simulink model "simulator_prototype_v2"  (R2021b)
(part 9 of 12)

t6280 = -t2307.*(t642+t643-t667+t674+t1587+t1606+t1608+t1609+t2295+t2671+t2683+t2684-t2695+t3272+t3290-t3296+t3576+t3582+t3588-t3593+t4015+t4016);
t6281 = -t2338.*(t642+t643-t667+t674+t1587+t1606+t1608+t1609+t2295+t2671+t2683+t2684-t2695+t3272+t3290-t3296+t3576+t3582+t3588-t3593+t4015+t4016);
t6282 = t5413.*t5588;
t6285 = t2338.*(t642+t643-t667+t674+t1587+t1606+t1608+t1609+t2295+t2671+t2683+t2684-t2695+t3272+t3290-t3296+t3576+t3582+t3588-t3593+t4015+t4016);
t6297 = -t5588.*(t410-t5413);
t6298 = t5588.*(t410-t5413);
t6304 = -t3386.*(t4554+t4572-t18.*t2363.*t3047.*1.02e-6-t23.*t2363.*t3047.*9.0e-8+t18.*t3946.*(t1896-t3232).*1.02e-6+t23.*t3946.*(t1896-t3232).*9.0e-8);
t6305 = t3386.*(t4554+t4572-t18.*t2363.*t3047.*1.02e-6-t23.*t2363.*t3047.*9.0e-8+t18.*t3946.*(t1896-t3232).*1.02e-6+t23.*t3946.*(t1896-t3232).*9.0e-8);
t6307 = t2363.*(t684+t685-t710+t724+t1686-t1690+t1700+t1701+t2371+t2698+t2707-t2716+t2719+t3319-t3327-t3341-t3620+t3622+t3634-t3638+t4076+t4077).*(-7.26735e-3);
t6308 = t2388.*(t684+t685-t710+t724+t1686-t1690+t1700+t1701+t2371+t2698+t2707-t2716+t2719+t3319-t3327-t3341-t3620+t3622+t3634-t3638+t4076+t4077).*(-7.26735e-3);
t6311 = t2419.*(t684+t685-t710+t724+t1686-t1690+t1700+t1701+t2371+t2698+t2707-t2716+t2719+t3319-t3327-t3341-t3620+t3622+t3634-t3638+t4076+t4077).*(-7.26735e-3);
t6314 = t3968+t4203+t4287+t4358+t4411+t4584;
t6315 = t4739+t4748+t4759+t4769;
t6327 = t33.*(t1896-t3232).*(t3424-t3437+t4552+t4556+t3942.*(t1896-t3232).*5.7e-7+t3946.*(t1896-t3232).*4.0e-8);
t6329 = -t33.*t3528.*(t3424-t3437+t4552+t4556+t3942.*(t1896-t3232).*5.7e-7+t3946.*(t1896-t3232).*4.0e-8);
t6331 = t33.*t3528.*(t3424-t3437+t4552+t4556+t3942.*(t1896-t3232).*5.7e-7+t3946.*(t1896-t3232).*4.0e-8);
t6338 = -t3877.*t5843.*(t1488+t1874+t2519+t2740+t2747+t3096+t3097);
t6348 = -t33.*t2363.*(t4737+t4744+t4751+t3942.*(t2694-t2701+t3036-t3043).*5.7e-7);
t6349 = t33.*t2363.*(t4737+t4744+t4751+t3942.*(t2694-t2701+t3036-t3043).*5.7e-7);
t6354 = -t2998.*(t4737+t4744+t4751+t3942.*(t2694-t2701+t3036-t3043).*5.7e-7);
t6355 = t2998.*(t4737+t4744+t4751+t3942.*(t2694-t2701+t3036-t3043).*5.7e-7);
t6357 = -t3057.*(t4737+t4744+t4751+t3942.*(t2694-t2701+t3036-t3043).*5.7e-7);
t6359 = (t1477-t2502).*(t4737+t4744+t4751+t3942.*(t2694-t2701+t3036-t3043).*5.7e-7);
t6360 = t3057.*(t4737+t4744+t4751+t3942.*(t2694-t2701+t3036-t3043).*5.7e-7);
t6369 = t4514.*t6038;
t6389 = t3385.*t6313;
t6394 = -t3985.*(t3424-t3437+t4552+t4556+t3942.*(t1896-t3232).*5.7e-7+t3946.*(t1896-t3232).*4.0e-8);
t6396 = (t3235-t3535).*(t3424-t3437+t4552+t4556+t3942.*(t1896-t3232).*5.7e-7+t3946.*(t1896-t3232).*4.0e-8);
t6397 = -t3992.*(t3424-t3437+t4552+t4556+t3942.*(t1896-t3232).*5.7e-7+t3946.*(t1896-t3232).*4.0e-8);
t6400 = -t3996.*(t3424-t3437+t4552+t4556+t3942.*(t1896-t3232).*5.7e-7+t3946.*(t1896-t3232).*4.0e-8);
t6408 = t33.*(t1896-t3232).*(t4737+t4744+t4751+t3942.*(t2694-t2701+t3036-t3043).*5.7e-7);
t6409 = -t33.*t3528.*(t4737+t4744+t4751+t3942.*(t2694-t2701+t3036-t3043).*5.7e-7);
t6411 = t33.*t3528.*(t4737+t4744+t4751+t3942.*(t2694-t2701+t3036-t3043).*5.7e-7);
t6427 = -t6426;
t6436 = t5588.*t5722;
t6437 = t5589.*t5722;
t6455 = -t3985.*(t4737+t4744+t4751+t3942.*(t2694-t2701+t3036-t3043).*5.7e-7);
t6456 = (t3235-t3535).*(t4737+t4744+t4751+t3942.*(t2694-t2701+t3036-t3043).*5.7e-7);
t6458 = -t3992.*(t4737+t4744+t4751+t3942.*(t2694-t2701+t3036-t3043).*5.7e-7);
t6463 = -t3996.*(t4737+t4744+t4751+t3942.*(t2694-t2701+t3036-t3043).*5.7e-7);
t6464 = t3992.*(t4737+t4744+t4751+t3942.*(t2694-t2701+t3036-t3043).*5.7e-7);
t6473 = t3049+t3256+t3266+t3976+t3980+t4373+t4378+t4387+t4394;
t6480 = -t4510.*(t4554+t4572-t18.*t2363.*t3047.*1.02e-6-t23.*t2363.*t3047.*9.0e-8+t18.*t3946.*(t1896-t3232).*1.02e-6+t23.*t3946.*(t1896-t3232).*9.0e-8);
t6483 = (t3544-t4013).*(t4554+t4572-t18.*t2363.*t3047.*1.02e-6-t23.*t2363.*t3047.*9.0e-8+t18.*t3946.*(t1896-t3232).*1.02e-6+t23.*t3946.*(t1896-t3232).*9.0e-8);
t6489 = t5426.*t5839;
t6490 = t5429.*t5839;
t6492 = -t5840.*(t410-t5413);
t6518 = -t4817.*(t3424-t3437+t4552+t4556+t3942.*(t1896-t3232).*5.7e-7+t3946.*(t1896-t3232).*4.0e-8);
t6519 = -t4824.*(t3424-t3437+t4552+t4556+t3942.*(t1896-t3232).*5.7e-7+t3946.*(t1896-t3232).*4.0e-8);
t6523 = t4514.*t6313;
t6534 = -t6533;
t6539 = t3180+t3196+t4735+t4743+t5017+t5022;
t6545 = -t3057.*(t4819+t4850+t4851+t3057.*(t1456-t2355).*1.02e-6+t3047.*(t1477-t2502).*1.02e-6+t3942.*(t3235-t3535).*1.02e-6);
et198 = -t2137+t2777+t2778+t2779-t2787+t4012-t4205+t4207+t27.*(t1959-t3306+t38.*t1022.*(t855-t878).*2.196325630278387e-1).*6.1855407534e-5;
et199 = t33.*(t1959-t3306+t38.*t1022.*(t855-t878).*2.196325630278387e-1).*1.35652563578e-4;
t6567 = -t5426.*(et198+et199);
et200 = -t2137+t2777+t2778+t2779-t2787+t4012-t4205+t4207+t27.*(t1959-t3306+t38.*t1022.*(t855-t878).*2.196325630278387e-1).*6.1855407534e-5;
et201 = t33.*(t1959-t3306+t38.*t1022.*(t855-t878).*2.196325630278387e-1).*1.35652563578e-4;
t6568 = t5426.*(et200+et201);
et202 = -t2137+t2777+t2778+t2779-t2787+t4012-t4205+t4207+t27.*(t1959-t3306+t38.*t1022.*(t855-t878).*2.196325630278387e-1).*6.1855407534e-5;
et203 = t33.*(t1959-t3306+t38.*t1022.*(t855-t878).*2.196325630278387e-1).*1.35652563578e-4;
t6569 = -t5429.*(et202+et203);
et204 = -t2137+t2777+t2778+t2779-t2787+t4012-t4205+t4207+t27.*(t1959-t3306+t38.*t1022.*(t855-t878).*2.196325630278387e-1).*6.1855407534e-5;
et205 = t33.*(t1959-t3306+t38.*t1022.*(t855-t878).*2.196325630278387e-1).*1.35652563578e-4;
t6570 = t5429.*(et204+et205);
t6572 = -t5992.*(t410-t5413);
t6573 = -t4817.*(t4737+t4744+t4751+t3942.*(t2694-t2701+t3036-t3043).*5.7e-7);
t6574 = -t4824.*(t4737+t4744+t4751+t3942.*(t2694-t2701+t3036-t3043).*5.7e-7);
t6585 = t5548.*t5951;
t6586 = t5588.*t5941;
t6591 = t5589.*t5941;
t6600 = t5588.*t5953;
et206 = t707+t708-t721-t722-t749+t762+t768-t777-t792-t793-t801-t802-t808+t813-t819+t821-t1629+t1637-t1640-t1641-t1659-t1661+t1666+t1667+t1683+t1692+t1705-t1712+t1758+t1759+t1775+t1776+t1973+t1993+t1994+t2023+t2053+t2060-t2089-t2090+t2098+t2099-t14.*t15.*t21.*t50.*t189.*3.670836568391568e-22;
et207 = t16.*t19.*t20.*t50.*t189.*(-3.279367663374749e-19)-t14.*t15.*t17.*t21.*t50.*t189.*7.075931802640439e-19;
et208 = t14.*t17.*t20.*t21.*t50.*t189.*(-1.190170786299927e-18)-t15.*t17.*t19.*t21.*t50.*t189.*1.190170786299927e-18;
et209 = t19.*t20.*t21.*t22.*t50.*t189.*(-3.226512155691387e-19);
t6602 = -t5588.*(et206+et207+et208+et209);
et210 = t707+t708-t721-t722-t749+t762+t768-t777-t792-t793-t801-t802-t808+t813-t819+t821-t1629+t1637-t1640-t1641-t1659-t1661+t1666+t1667+t1683+t1692+t1705-t1712+t1758+t1759+t1775+t1776+t1973+t1993+t1994+t2023+t2053+t2060-t2089-t2090+t2098+t2099-t14.*t15.*t21.*t50.*t189.*3.670836568391568e-22;
et211 = t16.*t19.*t20.*t50.*t189.*(-3.279367663374749e-19)-t14.*t15.*t17.*t21.*t50.*t189.*7.075931802640439e-19;
et212 = t14.*t17.*t20.*t21.*t50.*t189.*(-1.190170786299927e-18)-t15.*t17.*t19.*t21.*t50.*t189.*1.190170786299927e-18;
et213 = t19.*t20.*t21.*t22.*t50.*t189.*(-3.226512155691387e-19);
t6603 = t5588.*(et210+et211+et212+et213);
t6604 = t5589.*t5953;
t6635 = -t6633;
t6660 = (t3235-t3535).*(t4819+t4850+t4851+t3057.*(t1456-t2355).*1.02e-6+t3047.*(t1477-t2502).*1.02e-6+t3942.*(t3235-t3535).*1.02e-6);
t6662 = -t3992.*(t4819+t4850+t4851+t3057.*(t1456-t2355).*1.02e-6+t3047.*(t1477-t2502).*1.02e-6+t3942.*(t3235-t3535).*1.02e-6);
t6664 = t3992.*(t4819+t4850+t4851+t3057.*(t1456-t2355).*1.02e-6+t3047.*(t1477-t2502).*1.02e-6+t3942.*(t3235-t3535).*1.02e-6);
t6703 = t3057.*t6646;
t6706 = t5176+t5177+t5179+t5180;
t6753 = t5413.*t6183;
et214 = t1288+t1289+t1302+t1303-t1319-t1320+t1336-t1348+t1350+t1351-t1360+t1369-t1378+t1396-t1425+t1435-t2174+t2183-t2187+t2193-t2194-t2195+t2199-t2203-t2215+t2219-t2222-t2223+t2239+t2240-t2256-t2257+t2555+t2556+t2572+t2583-t2605-t2606+t2612+t2613-t2618-t2619+t2651+t2652;
et215 = t24.*t25.*t26.*t50.*t202.*(-3.566935413776081e-21);
et216 = t30.*t31.*t32.*t50.*t202.*(-3.992732227073824e-24);
et217 = t24.*t25.*t32.*t33.*t50.*t202.*(-3.509445006623964e-21);
et218 = t27.*t30.*t31.*t32.*t50.*t202.*(-7.696420262413979e-21);
t6763 = -t5426.*(et214+et215+et216+et217+et218);
et219 = t1288+t1289+t1302+t1303-t1319-t1320+t1336-t1348+t1350+t1351-t1360+t1369-t1378+t1396-t1425+t1435-t2174+t2183-t2187+t2193-t2194-t2195+t2199-t2203-t2215+t2219-t2222-t2223+t2239+t2240-t2256-t2257+t2555+t2556+t2572+t2583-t2605-t2606+t2612+t2613-t2618-t2619+t2651+t2652;
et220 = t24.*t25.*t26.*t50.*t202.*(-3.566935413776081e-21);
et221 = t30.*t31.*t32.*t50.*t202.*(-3.992732227073824e-24);
et222 = t24.*t25.*t32.*t33.*t50.*t202.*(-3.509445006623964e-21);
et223 = t27.*t30.*t31.*t32.*t50.*t202.*(-7.696420262413979e-21);
t6764 = t5426.*(et219+et220+et221+et222+et223);
t6776 = -t27.*t2363.*(-t4437-t4438+t4741+t4767+t3942.*(t2694-t2701+t3036-t3043).*4.0e-8+t3946.*(t2694-t2701+t3036-t3043).*2.4e-7);
t6777 = t27.*t2363.*(-t4437-t4438+t4741+t4767+t3942.*(t2694-t2701+t3036-t3043).*4.0e-8+t3946.*(t2694-t2701+t3036-t3043).*2.4e-7);
t6789 = -t3003.*(-t4437-t4438+t4741+t4767+t3942.*(t2694-t2701+t3036-t3043).*4.0e-8+t3946.*(t2694-t2701+t3036-t3043).*2.4e-7);
t6790 = t3003.*(-t4437-t4438+t4741+t4767+t3942.*(t2694-t2701+t3036-t3043).*4.0e-8+t3946.*(t2694-t2701+t3036-t3043).*2.4e-7);
t6793 = -t3057.*(-t4437-t4438+t4741+t4767+t3942.*(t2694-t2701+t3036-t3043).*4.0e-8+t3946.*(t2694-t2701+t3036-t3043).*2.4e-7);
t6794 = (t1477-t2502).*(-t4437-t4438+t4741+t4767+t3942.*(t2694-t2701+t3036-t3043).*4.0e-8+t3946.*(t2694-t2701+t3036-t3043).*2.4e-7);
t6796 = -t6646.*(t3235-t3535);
t6797 = t3992.*t6646;
t6804 = t4307+t4314+t4876+t4877+t4978+t4979;
t6805 = t5053+t5676+t5690;
t6807 = t3876+t4274+t4968+t4969+t5003+t5004;
t6814 = t27.*(t1896-t3232).*(-t4437-t4438+t4741+t4767+t3942.*(t2694-t2701+t3036-t3043).*4.0e-8+t3946.*(t2694-t2701+t3036-t3043).*2.4e-7);
t6815 = -t27.*t3528.*(-t4437-t4438+t4741+t4767+t3942.*(t2694-t2701+t3036-t3043).*4.0e-8+t3946.*(t2694-t2701+t3036-t3043).*2.4e-7);
t6835 = t3133+t3160+t3161+t3379+t4236+t4240+t4249+t4250+t4255+t4256+t4499+t4505;
t6885 = -t3985.*(-t4437-t4438+t4741+t4767+t3942.*(t2694-t2701+t3036-t3043).*4.0e-8+t3946.*(t2694-t2701+t3036-t3043).*2.4e-7);
t6887 = (t3235-t3535).*(-t4437-t4438+t4741+t4767+t3942.*(t2694-t2701+t3036-t3043).*4.0e-8+t3946.*(t2694-t2701+t3036-t3043).*2.4e-7);
t6888 = -t3992.*(-t4437-t4438+t4741+t4767+t3942.*(t2694-t2701+t3036-t3043).*4.0e-8+t3946.*(t2694-t2701+t3036-t3043).*2.4e-7);
t6890 = -t3996.*(-t4437-t4438+t4741+t4767+t3942.*(t2694-t2701+t3036-t3043).*4.0e-8+t3946.*(t2694-t2701+t3036-t3043).*2.4e-7);
t6908 = t5229+t5237+t5274+t5279;
t6909 = t3918.*(t4758.*(t1861-t3214)+t2297.*(t642+t643-t667+t674+t1587+t1606+t1608+t1609+t2295+t2671+t2683+t2684-t2695+t3272+t3290-t3296+t3576+t3582+t3588-t3593+t4015+t4016)).*(t2694-t2701+t3036-t3043).*7.26735e-3;
t6920 = t3984.*(t4758.*(t1861-t3214)+t2297.*(t642+t643-t667+t674+t1587+t1606+t1608+t1609+t2295+t2671+t2683+t2684-t2695+t3272+t3290-t3296+t3576+t3582+t3588-t3593+t4015+t4016)).*(t2694-t2701+t3036-t3043).*7.26735e-3;
t6923 = -t3877.*t6566.*(t1488+t1874+t2519+t2740+t2747+t3096+t3097);
t6925 = t3877.*t6566.*(t1488+t1874+t2519+t2740+t2747+t3096+t3097);
t6926 = t4149.*(t4758.*(t1861-t3214)+t2297.*(t642+t643-t667+t674+t1587+t1606+t1608+t1609+t2295+t2671+t2683+t2684-t2695+t3272+t3290-t3296+t3576+t3582+t3588-t3593+t4015+t4016)).*(t2694-t2701+t3036-t3043).*7.26735e-3;
t6958 = t3941.*(t4795.*(t1896-t3232).*7.26735e-3+t2363.*(t684+t685-t710+t724+t1686-t1690+t1700+t1701+t2371+t2698+t2707-t2716+t2719+t3319-t3327-t3341-t3620+t3622+t3634-t3638+t4076+t4077).*7.26735e-3).*(t2674-t2676+t3022-t3027);
t6972 = t4108.*(t4795.*(t1896-t3232).*7.26735e-3+t2363.*(t684+t685-t710+t724+t1686-t1690+t1700+t1701+t2371+t2698+t2707-t2716+t2719+t3319-t3327-t3341-t3620+t3622+t3634-t3638+t4076+t4077).*7.26735e-3).*(t2674-t2676+t3022-t3027);
t6974 = t5209+t5753+t5766;
t6984 = t4298.*(t4795.*(t1896-t3232).*7.26735e-3+t2363.*(t684+t685-t710+t724+t1686-t1690+t1700+t1701+t2371+t2698+t2707-t2716+t2719+t3319-t3327-t3341-t3620+t3622+t3634-t3638+t4076+t4077).*7.26735e-3).*(t2674-t2676+t3022-t3027);
t6986 = t3158+t3171+t3438+t3442+t4253+t4260+t4262+t4267+t4516+t4537+t4562+t4566;
t6992 = -t4814.*(-t4437-t4438+t4741+t4767+t3942.*(t2694-t2701+t3036-t3043).*4.0e-8+t3946.*(t2694-t2701+t3036-t3043).*2.4e-7);
et224 = t4127+t33.*(t1959-t3306+t38.*t1022.*(t855-t878).*2.196325630278387e-1);
et225 = -t4437-t4438+t4741+t4767+t3942.*(t2694-t2701+t3036-t3043).*4.0e-8+t3946.*(t2694-t2701+t3036-t3043).*2.4e-7;
t6993 = et224.*et225;
t7046 = t3558+t3559+t5260+t5261+t5268+t5269;
et226 = t3563.*1.33637554986e-4+t3693-t3694+t33.*(t1896-t3232).*4.36041e-5;
et227 = t33.*t34.*(t1896-t3232).*7.26350557185e-5;
t7050 = (et226+et227).*(t4758.*(t1861-t3214)+t2297.*(t642+t643-t667+t674+t1587+t1606+t1608+t1609+t2295+t2671+t2683+t2684-t2695+t3272+t3290-t3296+t3576+t3582+t3588-t3593+t4015+t4016));
et228 = t4758.*(t1861-t3214)+t2297.*(t642+t643-t667+t674+t1587+t1606+t1608+t1609+t2295+t2671+t2683+t2684-t2695+t3272+t3290-t3296+t3576+t3582+t3588-t3593+t4015+t4016);
et229 = t3349-t3649+t28.*(t3235-t3535).*1.33637554986e-4+t34.*(t3235-t3535).*7.26350557185e-5;
t7053 = et228.*et229;
t7056 = -t6975.*(-t1901+t3122+t3270);
et230 = t4795.*(t1896-t3232).*7.26735e-3+t2363.*(t684+t685-t710+t724+t1686-t1690+t1700+t1701+t2371+t2698+t2707-t2716+t2719+t3319-t3327-t3341-t3620+t3622+t3634-t3638+t4076+t4077).*7.26735e-3;
et231 = t3505.*1.838876e-2-t3570+t3571+t22.*(t1861-t3214).*(3.0./5.0e+2)+t22.*t23.*(t1861-t3214).*9.99471e-3;
t7057 = et230.*et231;
t7058 = t50.*t202.*t7042.*6.935255936130809e-19;
tau_c = ft_13({t1005,t1022,t1089,t1104,t1105,t1108,t1115,t1121,t1158,t1159,t1196,t1205,t1210,t1212,t1217,t1218,t123,t1237,t1238,t1288,t1289,t1302,t1303,t1319,t1320,t1336,t1348,t1350,t1351,t1360,t1369,t1378,t1396,t14,t140,t1425,t1435,t1456,t1477,t1488,t15,t1513,t1539,t1554,t1577,t1578,t1586,t1587,t16,t1600,t1604,t1605,t1606,t1607,t1608,t1609,t1615,t1616,t1628,t1629,t1637,t1640,t1641,t1659,t1660,t1661,t1666,t1667,t1683,t1686,t1690,t1692,t17,t1700,t1701,t1705,t1712,t1717,t1741,t1742,t1750,t1754,t1758,t1759,t1775,t1776,t18,t1861,t1874,t1879,t188,t1881,t189,t1896,t19,t1901,t1941,t1959,t1973,t1993,t1994,t2,t20,t201,t202,t2023,t2053,t2060,t2089,t2090,t2098,t2099,t21,t2117,t2120,t2122,t2123,t2139,t2140,t2147,t2152,t2154,t2155,t2159,t2165,t2174,t2183,t2187,t2193,t2194,t2195,t2199,t22,t2203,t2215,t2219,t2222,t2223,t2239,t2240,t2256,t2257,t2292,t2295,t2297,t23,t2302,t2303,t2306,t2307,t2308,t2317,t2337,t2338,t2339,t2355,t236,t2361,t2362,t2363,t2367,t2368,t237,t2371,t2378,t238,t2388,t24,t2401,t2403,t241,t2414,t2419,t244,t2493,t25,t2502,t2510,t2519,t2527,t2530,t2555,t2556,t2572,t2583,t2598,t26,t2605,t2606,t2612,t2613,t2618,t2619,t262,t264,t2651,t2652,t2670,t2671,t2673,t2674,t2676,t2680,t2683,t2684,t2685,t2686,t2687,t2689,t2692,t2693,t2694,t2695,t2697,t2698,t27,t2700,t2701,t2704,t2707,t2708,t2709,t2712,t2715,t2716,t2719,t2720,t2721,t2740,t2747,t2754,t28,t2801,t2804,t2813,t2814,t2820,t2831,t2834,t2835,t2838,t2850,t2851,t2945,t2950,t2953,t2955,t2957,t2963,t2964,t2975,t2979,t2990,t2991,t2993,t2994,t2998,t3,t30,t3003,t3009,t3017,t3022,t3027,t3030,t3036,t3043,t3045,t3047,t3054,t3055,t3056,t3057,t3063,t3064,t3072,t3079,t3080,t3096,t3097,t31,t3109,t3117,t3118,t3121,t3122,t3128,t3129,t313,t3130,t3131,t3132,t3134,t3135,t3139,t314,t3140,t3141,t3142,t3144,t3147,t3155,t3156,t3157,t3164,t3166,t3170,t3172,t3184,t3186,t3187,t3188,t3189,t3190,t3191,t3193,t3194,t3197,t3198,t3199,t32,t3200,t3201,t3206,t3209,t321,t3210,t3214,t3225,t3228,t3229,t3230,t3231,t3232,t3235,t3245,t3250,t3254,t3260,t3261,t3263,t3269,t3270,t3272,t3276,t3283,t329,t3290,t3291,t3292,t3296,t33,t3305,t3306,t3307,t3308,t3313,t3316,t3318,t3319,t332,t3324,t3326,t3327,t3330,t3334,t3335,t3336,t3337,t3341,t3344,t3349,t335,t3353,t3354,t3357,t3359,t3360,t3376,t3385,t3386,t3395,t3399,t34,t3405,t3409,t3410,t3412,t3415,t3417,t3419,t3420,t3421,t3423,t3424,t3428,t3432,t3433,t3435,t3437,t3440,t3444,t3449,t3450,t3451,t3453,t3455,t3456,t346,t3465,t3468,t3470,t3473,t3475,t3477,t3479,t3480,t3481,t3483,t3484,t3493,t3498,t35,t350,t3505,t3518,t3522,t3524,t3526,t3527,t3528,t3530,t3531,t3532,t3533,t3535,t3539,t354,t3542,t3544,t3547,t3560,t3563,t3569,t3570,t3571,t3576,t358,t3582,t3585,t3586,t3587,t3588,t3589,t359,t3590,t3593,t3596,t36,t3600,t3603,t3616,t3617,t3618,t3619,t3620,t3621,t3622,t3628,t3631,t3632,t3633,t3634,t3635,t3637,t3638,t3639,t3641,t3643,t3649,t3657,t366,t3663,t3664,t3665,t3667,t3669,t3670,t3672,t3673,t3674,t3676,t3678,t3679,t3680,t3681,t3682,t3683,t3684,t3685,t3686,t3687,t3689,t3690,t3693,t3694,t3705,t3706,t3708,t3709,t3712,t3713,t3714,t3715,t3716,t3718,t3723,t3724,t3729,t3732,t3734,t3735,t3736,t3744,t3745,t3746,t3748,t3749,t3751,t3753,t3755,t3756,t3757,t3758,t3759,t3760,t3762,t3763,t3764,t3765,t3766,t3767,t3768,t3769,t3770,t3771,t3772,t3774,t3775,t3776,t3778,t3779,t378,t3782,t3783,t3784,t3790,t3791,t3794,t3795,t3797,t3798,t3799,t38,t3801,t3803,t3804,t3806,t3811,t3814,t3815,t3816,t3817,t3819,t382,t3821,t3822,t3826,t3827,t3828,t3833,t3834,t3844,t3847,t3849,t3850,t3860,t3861,t3862,t3863,t3865,t3866,t3869,t387,t3870,t3871,t3872,t3875,t3877,t3880,t3882,t3891,t3892,t3893,t3898,t39,t3901,t3904,t3910,t3918,t3922,t3928,t3934,t3940,t3941,t3942,t3943,t3946,t3951,t3957,t3959,t3967,t3972,t3974,t3984,t3985,t3992,t3996,t4,t4007,t4011,t4013,t4015,t4016,t4027,t4034,t4035,t4036,t4037,t4062,t4071,t4072,t4076,t4077,t4080,t4086,t4089,t4090,t4091,t410,t4106,t4108,t4109,t4113,t4119,t4120,t4122,t4125,t4127,t4133,t4134,t4145,t4146,t4147,t4148,t4149,t4152,t4154,t4155,t4160,t4163,t4168,t4173,t4175,t4196,t42,t4200,t4201,t4219,t4220,t4221,t4227,t4228,t4230,t4231,t4233,t4234,t4235,t4237,t4238,t4239,t4242,t4243,t4244,t4245,t4246,t4247,t4248,t4255,t4256,t4257,t4259,t4263,t4264,t4266,t4268,t4276,t4277,t4279,t4280,t4281,t4285,t4287,t4291,t4292,t4295,t4296,t4297,t4298,t43,t4304,t4308,t4310,t4311,t4313,t4316,t4320,t4321,t4322,t4323,t4324,t4356,t4362,t4363,t4374,t4376,t4377,t4379,t4382,t4388,t4397,t4398,t4400,t4405,t4406,t4409,t4410,t4412,t4413,t4421,t4424,t4427,t4428,t4429,t4432,t4436,t4437,t4438,t4439,t4440,t4444,t4447,t4458,t4473,t4475,t4491,t4494,t4496,t4499,t4500,t4504,t4507,t4508,t4510,t4511,t4513,t4514,t4515,t4517,t4519,t4520,t4523,t4525,t4529,t4531,t4534,t4535,t4536,t4540,t4541,t4543,t4552,t4554,t4555,t4556,t4559,t4560,t4561,t4565,t4568,t4571,t4572,t4575,t4576,t4579,t4580,t4581,t4582,t4588,t4589,t4591,t4593,t4594,t4595,t4597,t4599,t46,t4600,t4602,t4610,t4612,t4613,t4614,t4615,t4617,t4620,t4623,t4625,t4627,t4628,t4629,t4631,t4633,t4634,t4635,t4636,t4638,t4640,t4641,t4642,t4644,t4645,t4647,t4650,t4651,t4652,t4655,t4658,t4659,t4661,t4663,t4664,t4666,t4667,t4669,t4676,t4677,t4678,t4679,t4680,t4682,t4683,t4685,t4686,t4688,t4699,t47,t4702,t4703,t4704,t4705,t4706,t4709,t4713,t4715,t4718,t4719,t4720,t4721,t4725,t4727,t4728,t4729,t4732,t4733,t4737,t4738,t4741,t4742,t4744,t4751,t4752,t4753,t4755,t4757,t4758,t4760,t4761,t4762,t4763,t4766,t4767,t4770,t4771,t4772,t4773,t4775,t4777,t4780,t4785,t4786,t4787,t4788,t4789,t4790,t4791,t4792,t4793,t4794,t4795,t4796,t4798,t4799,t4800,t4801,t4805,t4807,t4808,t4809,t4812,t4814,t4816,t4817,t4818,t4819,t4822,t4823,t4824,t4825,t4826,t4829,t4832,t4833,t4835,t4836,t4839,t4840,t4842,t4843,t4845,t4847,t4848,t4849,t4850,t4851,t4852,t4853,t4854,t4855,t4856,t4857,t4858,t4859,t4860,t4865,t4868,t4869,t4870,t4871,t4872,t4873,t4874,t4875,t4880,t4882,t4883,t4884,t4885,t4887,t4890,t4893,t4895,t4896,t4897,t4898,t4899,t4900,t4902,t4904,t4905,t4906,t4907,t4909,t4911,t4913,t4915,t4917,t4918,t4919,t4920,t4921,t4922,t4924,t4925,t4926,t4927,t4929,t4930,t4931,t4932,t4938,t4941,t4942,t4943,t4946,t4947,t4950,t4952,t4953,t4954,t4956,t4958,t4959,t4960,t4961,t4962,t4963,t4965,t4970,t4972,t4974,t4975,t4976,t4977,t4981,t4982,t4983,t4984,t4985,t4986,t4987,t4992,t4994,t4995,t4996,t4998,t5,t50,t5000,t5001,t5002,t5005,t5007,t5008,t5010,t5012,t5013,t5014,t5015,t5021,t5023,t5025,t5026,t5027,t5028,t5030,t5031,t5032,t5033,t5034,t5035,t5036,t5038,t5039,t5040,t5041,t5042,t5047,t5048,t5049,t5051,t5052,t5054,t5055,t5056,t5057,t5058,t5059,t5061,t5062,t5063,t5064,t5066,t5067,t5068,t5069,t5070,t5071,t5073,t5074,t5075,t5076,t5077,t5083,t5085,t5086,t5087,t5088,t5089,t5092,t5097,t5098,t5099,t5100,t5102,t5103,t5104,t5105,t5106,t5108,t5109,t5111,t5112,t5113,t5114,t5115,t5116,t5117,t5119,t5121,t5123,t5126,t5127,t5128,t5130,t5131,t5135,t5137,t5138,t5139,t5141,t5142,t5143,t5144,t5145,t5146,t5147,t5148,t5149,t5150,t5151,t5152,t5153,t5155,t5156,t5157,t5158,t5161,t5162,t5164,t5165,t5166,t5169,t5172,t5173,t5184,t5185,t5186,t5187,t5189,t5190,t5191,t5192,t5193,t5194,t5195,t5196,t5198,t5201,t5202,t5203,t5204,t5206,t5207,t5208,t5209,t5210,t5212,t5214,t5215,t5216,t5217,t5220,t5221,t5222,t5223,t5224,t5225,t5226,t5227,t5228,t5230,t5231,t5233,t5234,t5235,t5236,t5238,t5239,t5240,t5241,t5242,t5243,t5244,t5245,t5246,t5247,t5248,t5250,t5252,t5254,t5255,t5257,t5258,t5262,t5271,t5272,t5273,t5276,t5277,t5278,t5280,t5281,t5282,t5283,t5284,t5285,t5286,t5287,t5288,t5289,t5291,t5293,t5295,t5301,t5302,t5304,t5306,t5307,t5308,t5309,t5311,t5314,t5316,t5317,t5320,t5321,t5322,t5326,t5328,t5329,t5330,t5331,t5332,t5333,t5335,t5336,t5337,t5338,t5339,t5340,t5342,t5344,t5345,t5346,t5347,t5348,t5349,t5350,t5352,t5356,t5357,t5358,t5359,t5361,t5362,t5365,t5367,t5371,t5377,t5379,t5380,t5381,t5383,t5384,t5385,t5386,t5387,t5388,t5389,t5390,t5391,t5392,t5393,t5395,t5396,t5397,t5399,t5400,t5402,t5403,t5405,t5407,t5408,t5409,t5411,t5412,t5413,t5414,t5416,t5418,t5419,t5420,t5423,t5424,t5426,t5427,t5428,t5429,t5430,t5432,t5433,t5434,t5435,t5437,t5438,t5440,t5441,t5443,t5444,t5445,t5446,t5447,t5448,t5449,t5450,t5451,t5452,t5453,t5454,t5455,t5456,t5457,t5458,t5459,t5461,t5462,t5464,t5465,t5466,t5467,t5468,t5469,t5473,t5474,t5476,t5477,t5479,t5480,t5481,t5482,t5483,t5484,t5485,t5486,t5487,t5488,t5489,t5490,t5491,t5492,t5493,t5494,t5496,t5498,t5499,t5500,t5503,t5504,t5505,t5506,t5507,t5509,t5512,t5513,t5514,t5515,t5516,t5517,t5518,t5520,t5521,t5522,t5523,t5524,t5525,t5526,t5528,t5530,t5531,t5532,t5533,t5534,t5535,t5536,t5537,t5538,t5539,t5541,t5542,t5543,t5544,t5545,t5546,t5547,t5550,t5551,t5552,t5553,t5554,t5556,t5557,t5558,t5559,t5561,t5563,t5564,t5566,t5568,t5569,t5570,t5573,t5574,t5575,t5576,t5577,t5578,t5579,t5580,t5581,t5582,t5583,t5585,t5588,t5589,t5590,t5592,t5593,t5594,t5595,t5596,t5597,t56,t5600,t5601,t5602,t5603,t5604,t5605,t5606,t5610,t5615,t5617,t5619,t5620,t5621,t5622,t5623,t5624,t5625,t5626,t5627,t5628,t5629,t5631,t5632,t5635,t5636,t5639,t5641,t5644,t5648,t5651,t5653,t5655,t5658,t5659,t5660,t5661,t5662,t5663,t5664,t5665,t5666,t5667,t5670,t5671,t5674,t5675,t5678,t5679,t5680,t5681,t5682,t5685,t5686,t5687,t5689,t5691,t5693,t5694,t5695,t5696,t5698,t5699,t5700,t5701,t5702,t5703,t5704,t5705,t5706,t5707,t5708,t5709,t5711,t5712,t5714,t5715,t5717,t5718,t5720,t5721,t5722,t5723,t5725,t5726,t5727,t5728,t5730,t5731,t5733,t5735,t5737,t5739,t5740,t5741,t5742,t5748,t5749,t5750,t5751,t5756,t5757,t5760,t5761,t5762,t5764,t5765,t5768,t5770,t5771,t5772,t5773,t5775,t5776,t5777,t5778,t5779,t5780,t5782,t5783,t5785,t5786,t5787,t5788,t5791,t5792,t5793,t5794,t5796,t5798,t5799,t5804,t5805,t5807,t5808,t5809,t5813,t5815,t5816,t5818,t5820,t5821,t5824,t5825,t5828,t5829,t5831,t5832,t5833,t5835,t5836,t5838,t5840,t5842,t5843,t5845,t5846,t5850,t5851,t5852,t5853,t5854,t5855,t5857,t5858,t5859,t5860,t5861,t5862,t5863,t5864,t5865,t5866,t5868,t5870,t5871,t5873,t5876,t5877,t5879,t5881,t5882,t5883,t5884,t5887,t5888,t5889,t5890,t5891,t5894,t5896,t5899,t5900,t5902,t5904,t5907,t5908,t5910,t5911,t5912,t5913,t5914,t5916,t5917,t5918,t5922,t5923,t5924,t5926,t5927,t5929,t5930,t5932,t5933,t5935,t5937,t5940,t5943,t5944,t5945,t5947,t5951,t5952,t5953,t5954,t5956,t5957,t5958,t5959,t5960,t5963,t5966,t5968,t5969,t5970,t5972,t5975,t5977,t5978,t5979,t5980,t5981,t5986,t5988,t5991,t5992,t5994,t5996,t5997,t5998,t6,t60,t6000,t6001,t6002,t6004,t6008,t6009,t6010,t6012,t6015,t6016,t6017,t6018,t6019,t6020,t6021,t6028,t6030,t6031,t6034,t6035,t6038,t6039,t6042,t6043,t6046,t6047,t6049,t6050,t6051,t6054,t6057,t6058,t6060,t6062,t6064,t6066,t6067,t6075,t6076,t6087,t6088,t6091,t6092,t6095,t6096,t6100,t6101,t6103,t6104,t6112,t6119,t6135,t6137,t6138,t6140,t6143,t6144,t6147,t6150,t6151,t6156,t6160,t6161,t6162,t6165,t6168,t6169,t6173,t6175,t6183,t6184,t6185,t6189,t6198,t6199,t6200,t6201,t6202,t6206,t6207,t6209,t6210,t6211,t6219,t6221,t6223,t6224,t6232,t6238,t6244,t6245,t6247,t6248,t6251,t6253,t6257,t6267,t6271,t6279,t6280,t6282,t6285,t6293,t6297,t6298,t6302,t6303,t6304,t6305,t6307,t6308,t6311,t6313,t6315,t6317,t6321,t6322,t6323,t6327,t6331,t6338,t6339,t6341,t6343,t6344,t6348,t6349,t6354,t6356,t6357,t6359,t6360,t6365,t6366,t6367,t6369,t6375,t6378,t6387,t6388,t6389,t6394,t6396,t6397,t640,t6400,t6406,t6407,t6408,t6411,t6414,t642,t6427,t643,t6431,t6436,t6437,t6441,t6442,t6450,t6451,t6452,t6453,t6455,t6456,t6463,t6464,t6473,t6480,t6481,t6483,t6484,t6485,t6486,t6489,t649,t6490,t6492,t6493,t6497,t6507,t6508,t6511,t6515,t6518,t6519,t6521,t6523,t6528,t6529,t6533,t6534,t6539,t6543,t6544,t6545,t656,t6565,t6566,t6568,t6570,t6572,t6573,t6574,t6575,t6584,t6585,t6586,t659,t6591,t6593,t660,t6600,t6603,t6604,t6611,t6612,t6634,t6635,t6658,t6660,t6663,t6664,t667,t668,t6689,t669,t6691,t6692,t67,t670,t6703,t6706,t674,t6752,t6753,t6763,t6764,t677,t6776,t6777,t6789,t6793,t6794,t6796,t6797,t68,t6804,t6805,t6807,t681,t6811,t6812,t6813,t6814,t6815,t682,t684,t685,t686,t6860,t6861,t687,t6873,t6885,t6887,t6888,t6890,t6892,t6893,t6909,t6913,t6916,t6917,t6920,t6924,t6925,t6926,t6927,t6928,t6937,t694,t6954,t6955,t6958,t6972,t6975,t6979,t6984,t6986,t6987,t6988,t6989,t6990,t6992,t6993,t7,t7012,t7015,t7027,t7028,t7029,t7039,t7041,t7044,t7046,t7049,t7050,t7051,t7053,t7054,t7055,t7056,t7057,t7058,t7062,t7065,t707,t708,t7091,t71,t710,t7107,t715,t716,t7181,t7193,t7204,t721,t7219,t722,t7228,t7229,t724,t725,t7280,t7291,t7292,t7294,t73,t736,t740,t741,t749,t762,t768,t7723,t7731,t7732,t7734,t777,t7790,t792,t793,t801,t802,t808,t813,t819,t821,t850,t855,t874,t878,t89,t92,t941,t948,t951,t97});
end
function tau_c = ft_13(ct)
t1005 = ct{1};
t1022 = ct{2};
t1089 = ct{3};
t1104 = ct{4};
t1105 = ct{5};
t1108 = ct{6};
t1115 = ct{7};
t1121 = ct{8};
t1158 = ct{9};
t1159 = ct{10};
t1196 = ct{11};
t1205 = ct{12};
t1210 = ct{13};
t1212 = ct{14};
t1217 = ct{15};
t1218 = ct{16};
t123 = ct{17};
t1237 = ct{18};
t1238 = ct{19};
t1288 = ct{20};
t1289 = ct{21};
t1302 = ct{22};
t1303 = ct{23};
t1319 = ct{24};
t1320 = ct{25};
t1336 = ct{26};
t1348 = ct{27};
t1350 = ct{28};
t1351 = ct{29};
t1360 = ct{30};
t1369 = ct{31};
t1378 = ct{32};
t1396 = ct{33};
t14 = ct{34};
t140 = ct{35};
t1425 = ct{36};
t1435 = ct{37};
t1456 = ct{38};
t1477 = ct{39};
t1488 = ct{40};
t15 = ct{41};
t1513 = ct{42};
t1539 = ct{43};
t1554 = ct{44};
t1577 = ct{45};
t1578 = ct{46};
t1586 = ct{47};
t1587 = ct{48};
t16 = ct{49};
t1600 = ct{50};
t1604 = ct{51};
t1605 = ct{52};
t1606 = ct{53};
t1607 = ct{54};
t1608 = ct{55};
t1609 = ct{56};
t1615 = ct{57};
t1616 = ct{58};
t1628 = ct{59};
t1629 = ct{60};
t1637 = ct{61};
t1640 = ct{62};
t1641 = ct{63};
t1659 = ct{64};
t1660 = ct{65};
t1661 = ct{66};
t1666 = ct{67};
t1667 = ct{68};
t1683 = ct{69};
t1686 = ct{70};
t1690 = ct{71};
t1692 = ct{72};
t17 = ct{73};
t1700 = ct{74};
t1701 = ct{75};
t1705 = ct{76};
t1712 = ct{77};
t1717 = ct{78};
t1741 = ct{79};
t1742 = ct{80};
t1750 = ct{81};
t1754 = ct{82};
t1758 = ct{83};
t1759 = ct{84};
t1775 = ct{85};
t1776 = ct{86};
t18 = ct{87};
t1861 = ct{88};
t1874 = ct{89};
t1879 = ct{90};
t188 = ct{91};
t1881 = ct{92};
t189 = ct{93};
t1896 = ct{94};
t19 = ct{95};
t1901 = ct{96};
t1941 = ct{97};
t1959 = ct{98};
t1973 = ct{99};
t1993 = ct{100};
t1994 = ct{101};
t2 = ct{102};
t20 = ct{103};
t201 = ct{104};
t202 = ct{105};
t2023 = ct{106};
t2053 = ct{107};
t2060 = ct{108};
t2089 = ct{109};
t2090 = ct{110};
t2098 = ct{111};
t2099 = ct{112};
t21 = ct{113};
t2117 = ct{114};
t2120 = ct{115};
t2122 = ct{116};
t2123 = ct{117};
t2139 = ct{118};
t2140 = ct{119};
t2147 = ct{120};
t2152 = ct{121};
t2154 = ct{122};
t2155 = ct{123};
t2159 = ct{124};
t2165 = ct{125};
t2174 = ct{126};
t2183 = ct{127};
t2187 = ct{128};
t2193 = ct{129};
t2194 = ct{130};
t2195 = ct{131};
t2199 = ct{132};
t22 = ct{133};
t2203 = ct{134};
t2215 = ct{135};
t2219 = ct{136};
t2222 = ct{137};
t2223 = ct{138};
t2239 = ct{139};
t2240 = ct{140};
t2256 = ct{141};
t2257 = ct{142};
t2292 = ct{143};
t2295 = ct{144};
t2297 = ct{145};
t23 = ct{146};
t2302 = ct{147};
t2303 = ct{148};
t2306 = ct{149};
t2307 = ct{150};
t2308 = ct{151};
t2317 = ct{152};
t2337 = ct{153};
t2338 = ct{154};
t2339 = ct{155};
t2355 = ct{156};
t236 = ct{157};
t2361 = ct{158};
t2362 = ct{159};
t2363 = ct{160};
t2367 = ct{161};
t2368 = ct{162};
t237 = ct{163};
t2371 = ct{164};
t2378 = ct{165};
t238 = ct{166};
t2388 = ct{167};
t24 = ct{168};
t2401 = ct{169};
t2403 = ct{170};
t241 = ct{171};
t2414 = ct{172};
t2419 = ct{173};
t244 = ct{174};
t2493 = ct{175};
t25 = ct{176};
t2502 = ct{177};
t2510 = ct{178};
t2519 = ct{179};
t2527 = ct{180};
t2530 = ct{181};
t2555 = ct{182};
t2556 = ct{183};
t2572 = ct{184};
t2583 = ct{185};
t2598 = ct{186};
t26 = ct{187};
t2605 = ct{188};
t2606 = ct{189};
t2612 = ct{190};
t2613 = ct{191};
t2618 = ct{192};
t2619 = ct{193};
t262 = ct{194};
t264 = ct{195};
t2651 = ct{196};
t2652 = ct{197};
t2670 = ct{198};
t2671 = ct{199};
t2673 = ct{200};
t2674 = ct{201};
t2676 = ct{202};
t2680 = ct{203};
t2683 = ct{204};
t2684 = ct{205};
t2685 = ct{206};
t2686 = ct{207};
t2687 = ct{208};
t2689 = ct{209};
t2692 = ct{210};
t2693 = ct{211};
t2694 = ct{212};
t2695 = ct{213};
t2697 = ct{214};
t2698 = ct{215};
t27 = ct{216};
t2700 = ct{217};
t2701 = ct{218};
t2704 = ct{219};
t2707 = ct{220};
t2708 = ct{221};
t2709 = ct{222};
t2712 = ct{223};
t2715 = ct{224};
t2716 = ct{225};
t2719 = ct{226};
t2720 = ct{227};
t2721 = ct{228};
t2740 = ct{229};
t2747 = ct{230};
t2754 = ct{231};
t28 = ct{232};
t2801 = ct{233};
t2804 = ct{234};
t2813 = ct{235};
t2814 = ct{236};
t2820 = ct{237};
t2831 = ct{238};
t2834 = ct{239};
t2835 = ct{240};
t2838 = ct{241};
t2850 = ct{242};
t2851 = ct{243};
t2945 = ct{244};
t2950 = ct{245};
t2953 = ct{246};
t2955 = ct{247};
t2957 = ct{248};
t2963 = ct{249};
t2964 = ct{250};
t2975 = ct{251};
t2979 = ct{252};
t2990 = ct{253};
t2991 = ct{254};
t2993 = ct{255};
t2994 = ct{256};
t2998 = ct{257};
t3 = ct{258};
t30 = ct{259};
t3003 = ct{260};
t3009 = ct{261};
t3017 = ct{262};
t3022 = ct{263};
t3027 = ct{264};
t3030 = ct{265};
t3036 = ct{266};
t3043 = ct{267};
t3045 = ct{268};
t3047 = ct{269};
t3054 = ct{270};
t3055 = ct{271};
t3056 = ct{272};
t3057 = ct{273};
t3063 = ct{274};
t3064 = ct{275};
t3072 = ct{276};
t3079 = ct{277};
t3080 = ct{278};
t3096 = ct{279};
t3097 = ct{280};
t31 = ct{281};
t3109 = ct{282};
t3117 = ct{283};
t3118 = ct{284};
t3121 = ct{285};
t3122 = ct{286};
t3128 = ct{287};
t3129 = ct{288};
t313 = ct{289};
t3130 = ct{290};
t3131 = ct{291};
t3132 = ct{292};
t3134 = ct{293};
t3135 = ct{294};
t3139 = ct{295};
t314 = ct{296};
t3140 = ct{297};
t3141 = ct{298};
t3142 = ct{299};
t3144 = ct{300};
t3147 = ct{301};
t3155 = ct{302};
t3156 = ct{303};
t3157 = ct{304};
t3164 = ct{305};
t3166 = ct{306};
t3170 = ct{307};
t3172 = ct{308};
t3184 = ct{309};
t3186 = ct{310};
t3187 = ct{311};
t3188 = ct{312};
t3189 = ct{313};
t3190 = ct{314};
t3191 = ct{315};
t3193 = ct{316};
t3194 = ct{317};
t3197 = ct{318};
t3198 = ct{319};
t3199 = ct{320};
t32 = ct{321};
t3200 = ct{322};
t3201 = ct{323};
t3206 = ct{324};
t3209 = ct{325};
t321 = ct{326};
t3210 = ct{327};
t3214 = ct{328};
t3225 = ct{329};
t3228 = ct{330};
t3229 = ct{331};
t3230 = ct{332};
t3231 = ct{333};
t3232 = ct{334};
t3235 = ct{335};
t3245 = ct{336};
t3250 = ct{337};
t3254 = ct{338};
t3260 = ct{339};
t3261 = ct{340};
t3263 = ct{341};
t3269 = ct{342};
t3270 = ct{343};
t3272 = ct{344};
t3276 = ct{345};
t3283 = ct{346};
t329 = ct{347};
t3290 = ct{348};
t3291 = ct{349};
t3292 = ct{350};
t3296 = ct{351};
t33 = ct{352};
t3305 = ct{353};
t3306 = ct{354};
t3307 = ct{355};
t3308 = ct{356};
t3313 = ct{357};
t3316 = ct{358};
t3318 = ct{359};
t3319 = ct{360};
t332 = ct{361};
t3324 = ct{362};
t3326 = ct{363};
t3327 = ct{364};
t3330 = ct{365};
t3334 = ct{366};
t3335 = ct{367};
t3336 = ct{368};
t3337 = ct{369};
t3341 = ct{370};
t3344 = ct{371};
t3349 = ct{372};
t335 = ct{373};
t3353 = ct{374};
t3354 = ct{375};
t3357 = ct{376};
t3359 = ct{377};
t3360 = ct{378};
t3376 = ct{379};
t3385 = ct{380};
t3386 = ct{381};
t3395 = ct{382};
t3399 = ct{383};
t34 = ct{384};
t3405 = ct{385};
t3409 = ct{386};
t3410 = ct{387};
t3412 = ct{388};
t3415 = ct{389};
t3417 = ct{390};
t3419 = ct{391};
t3420 = ct{392};
t3421 = ct{393};
t3423 = ct{394};
t3424 = ct{395};
t3428 = ct{396};
t3432 = ct{397};
t3433 = ct{398};
t3435 = ct{399};
t3437 = ct{400};
t3440 = ct{401};
t3444 = ct{402};
t3449 = ct{403};
t3450 = ct{404};
t3451 = ct{405};
t3453 = ct{406};
t3455 = ct{407};
t3456 = ct{408};
t346 = ct{409};
t3465 = ct{410};
t3468 = ct{411};
t3470 = ct{412};
t3473 = ct{413};
t3475 = ct{414};
t3477 = ct{415};
t3479 = ct{416};
t3480 = ct{417};
t3481 = ct{418};
t3483 = ct{419};
t3484 = ct{420};
t3493 = ct{421};
t3498 = ct{422};
t35 = ct{423};
t350 = ct{424};
t3505 = ct{425};
t3518 = ct{426};
t3522 = ct{427};
t3524 = ct{428};
t3526 = ct{429};
t3527 = ct{430};
t3528 = ct{431};
t3530 = ct{432};
t3531 = ct{433};
t3532 = ct{434};
t3533 = ct{435};
t3535 = ct{436};
t3539 = ct{437};
t354 = ct{438};
t3542 = ct{439};
t3544 = ct{440};
t3547 = ct{441};
t3560 = ct{442};
t3563 = ct{443};
t3569 = ct{444};
t3570 = ct{445};
t3571 = ct{446};
t3576 = ct{447};
t358 = ct{448};
t3582 = ct{449};
t3585 = ct{450};
t3586 = ct{451};
t3587 = ct{452};
t3588 = ct{453};
t3589 = ct{454};
t359 = ct{455};
t3590 = ct{456};
t3593 = ct{457};
t3596 = ct{458};
t36 = ct{459};
t3600 = ct{460};
t3603 = ct{461};
t3616 = ct{462};
t3617 = ct{463};
t3618 = ct{464};
t3619 = ct{465};
t3620 = ct{466};
t3621 = ct{467};
t3622 = ct{468};
t3628 = ct{469};
t3631 = ct{470};
t3632 = ct{471};
t3633 = ct{472};
t3634 = ct{473};
t3635 = ct{474};
t3637 = ct{475};
t3638 = ct{476};
t3639 = ct{477};
t3641 = ct{478};
t3643 = ct{479};
t3649 = ct{480};
t3657 = ct{481};
t366 = ct{482};
t3663 = ct{483};
t3664 = ct{484};
t3665 = ct{485};
t3667 = ct{486};
t3669 = ct{487};
t3670 = ct{488};
t3672 = ct{489};
t3673 = ct{490};
t3674 = ct{491};
t3676 = ct{492};
t3678 = ct{493};
t3679 = ct{494};
t3680 = ct{495};
t3681 = ct{496};
t3682 = ct{497};
t3683 = ct{498};
t3684 = ct{499};
t3685 = ct{500};
t3686 = ct{501};
t3687 = ct{502};
t3689 = ct{503};
t3690 = ct{504};
t3693 = ct{505};
t3694 = ct{506};
t3705 = ct{507};
t3706 = ct{508};
t3708 = ct{509};
t3709 = ct{510};
t3712 = ct{511};
t3713 = ct{512};
t3714 = ct{513};
t3715 = ct{514};
t3716 = ct{515};
t3718 = ct{516};
t3723 = ct{517};
t3724 = ct{518};
t3729 = ct{519};
t3732 = ct{520};
t3734 = ct{521};
t3735 = ct{522};
t3736 = ct{523};
t3744 = ct{524};
t3745 = ct{525};
t3746 = ct{526};
t3748 = ct{527};
t3749 = ct{528};
t3751 = ct{529};
t3753 = ct{530};
t3755 = ct{531};
t3756 = ct{532};
t3757 = ct{533};
t3758 = ct{534};
t3759 = ct{535};
t3760 = ct{536};
t3762 = ct{537};
t3763 = ct{538};
t3764 = ct{539};
t3765 = ct{540};
t3766 = ct{541};
t3767 = ct{542};
t3768 = ct{543};
t3769 = ct{544};
t3770 = ct{545};
t3771 = ct{546};
t3772 = ct{547};
t3774 = ct{548};
t3775 = ct{549};
t3776 = ct{550};
t3778 = ct{551};
t3779 = ct{552};
t378 = ct{553};
t3782 = ct{554};
t3783 = ct{555};
t3784 = ct{556};
t3790 = ct{557};
t3791 = ct{558};
t3794 = ct{559};
t3795 = ct{560};
t3797 = ct{561};
t3798 = ct{562};
t3799 = ct{563};
t38 = ct{564};
t3801 = ct{565};
t3803 = ct{566};
t3804 = ct{567};
t3806 = ct{568};
t3811 = ct{569};
t3814 = ct{570};
t3815 = ct{571};
t3816 = ct{572};
t3817 = ct{573};
t3819 = ct{574};
t382 = ct{575};
t3821 = ct{576};
t3822 = ct{577};
t3826 = ct{578};
t3827 = ct{579};
t3828 = ct{580};
t3833 = ct{581};
t3834 = ct{582};
t3844 = ct{583};
t3847 = ct{584};
t3849 = ct{585};
t3850 = ct{586};
t3860 = ct{587};
t3861 = ct{588};
t3862 = ct{589};
t3863 = ct{590};
t3865 = ct{591};
t3866 = ct{592};
t3869 = ct{593};
t387 = ct{594};
t3870 = ct{595};
t3871 = ct{596};
t3872 = ct{597};
t3875 = ct{598};
t3877 = ct{599};
t3880 = ct{600};
t3882 = ct{601};
t3891 = ct{602};
t3892 = ct{603};
t3893 = ct{604};
t3898 = ct{605};
t39 = ct{606};
t3901 = ct{607};
t3904 = ct{608};
t3910 = ct{609};
t3918 = ct{610};
t3922 = ct{611};
t3928 = ct{612};
t3934 = ct{613};
t3940 = ct{614};
t3941 = ct{615};
t3942 = ct{616};
t3943 = ct{617};
t3946 = ct{618};
t3951 = ct{619};
t3957 = ct{620};
t3959 = ct{621};
t3967 = ct{622};
t3972 = ct{623};
t3974 = ct{624};
t3984 = ct{625};
t3985 = ct{626};
t3992 = ct{627};
t3996 = ct{628};
t4 = ct{629};
t4007 = ct{630};
t4011 = ct{631};
t4013 = ct{632};
t4015 = ct{633};
t4016 = ct{634};
t4027 = ct{635};
t4034 = ct{636};
t4035 = ct{637};
t4036 = ct{638};
t4037 = ct{639};
t4062 = ct{640};
t4071 = ct{641};
t4072 = ct{642};
t4076 = ct{643};
t4077 = ct{644};
t4080 = ct{645};
t4086 = ct{646};
t4089 = ct{647};
t4090 = ct{648};
t4091 = ct{649};
t410 = ct{650};
t4106 = ct{651};
t4108 = ct{652};
t4109 = ct{653};
t4113 = ct{654};
t4119 = ct{655};
t4120 = ct{656};
t4122 = ct{657};
t4125 = ct{658};
t4127 = ct{659};
t4133 = ct{660};
t4134 = ct{661};
t4145 = ct{662};
t4146 = ct{663};
t4147 = ct{664};
t4148 = ct{665};
t4149 = ct{666};
t4152 = ct{667};
t4154 = ct{668};
t4155 = ct{669};
t4160 = ct{670};
t4163 = ct{671};
t4168 = ct{672};
t4173 = ct{673};
t4175 = ct{674};
t4196 = ct{675};
t42 = ct{676};
t4200 = ct{677};
t4201 = ct{678};
t4219 = ct{679};
t4220 = ct{680};
t4221 = ct{681};
t4227 = ct{682};
t4228 = ct{683};
t4230 = ct{684};
t4231 = ct{685};
t4233 = ct{686};
t4234 = ct{687};
t4235 = ct{688};
t4237 = ct{689};
t4238 = ct{690};
t4239 = ct{691};
t4242 = ct{692};
t4243 = ct{693};
t4244 = ct{694};
t4245 = ct{695};
t4246 = ct{696};
t4247 = ct{697};
t4248 = ct{698};
t4255 = ct{699};
t4256 = ct{700};
t4257 = ct{701};
t4259 = ct{702};
t4263 = ct{703};
t4264 = ct{704};
t4266 = ct{705};
t4268 = ct{706};
t4276 = ct{707};
t4277 = ct{708};
t4279 = ct{709};
t4280 = ct{710};
t4281 = ct{711};
t4285 = ct{712};
t4287 = ct{713};
t4291 = ct{714};
t4292 = ct{715};
t4295 = ct{716};
t4296 = ct{717};
t4297 = ct{718};
t4298 = ct{719};
t43 = ct{720};
t4304 = ct{721};
t4308 = ct{722};
t4310 = ct{723};
t4311 = ct{724};
t4313 = ct{725};
t4316 = ct{726};
t4320 = ct{727};
t4321 = ct{728};
t4322 = ct{729};
t4323 = ct{730};
t4324 = ct{731};
t4356 = ct{732};
t4362 = ct{733};
t4363 = ct{734};
t4374 = ct{735};
t4376 = ct{736};
t4377 = ct{737};
t4379 = ct{738};
t4382 = ct{739};
t4388 = ct{740};
t4397 = ct{741};
t4398 = ct{742};
t4400 = ct{743};
t4405 = ct{744};
t4406 = ct{745};
t4409 = ct{746};
t4410 = ct{747};
t4412 = ct{748};
t4413 = ct{749};
t4421 = ct{750};
t4424 = ct{751};
t4427 = ct{752};
t4428 = ct{753};
t4429 = ct{754};
t4432 = ct{755};
t4436 = ct{756};
t4437 = ct{757};
t4438 = ct{758};
t4439 = ct{759};
t4440 = ct{760};
t4444 = ct{761};
t4447 = ct{762};
t4458 = ct{763};
t4473 = ct{764};
t4475 = ct{765};
t4491 = ct{766};
t4494 = ct{767};
t4496 = ct{768};
t4499 = ct{769};
t4500 = ct{770};
t4504 = ct{771};
t4507 = ct{772};
t4508 = ct{773};
t4510 = ct{774};
t4511 = ct{775};
t4513 = ct{776};
t4514 = ct{777};
t4515 = ct{778};
t4517 = ct{779};
t4519 = ct{780};
t4520 = ct{781};
t4523 = ct{782};
t4525 = ct{783};
t4529 = ct{784};
t4531 = ct{785};
t4534 = ct{786};
t4535 = ct{787};
t4536 = ct{788};
t4540 = ct{789};
t4541 = ct{790};
t4543 = ct{791};
t4552 = ct{792};
t4554 = ct{793};
t4555 = ct{794};
t4556 = ct{795};
t4559 = ct{796};
t4560 = ct{797};
t4561 = ct{798};
t4565 = ct{799};
t4568 = ct{800};
t4571 = ct{801};
t4572 = ct{802};
t4575 = ct{803};
t4576 = ct{804};
t4579 = ct{805};
t4580 = ct{806};
t4581 = ct{807};
t4582 = ct{808};
t4588 = ct{809};
t4589 = ct{810};
t4591 = ct{811};
t4593 = ct{812};
t4594 = ct{813};
t4595 = ct{814};
t4597 = ct{815};
t4599 = ct{816};
t46 = ct{817};
t4600 = ct{818};
t4602 = ct{819};
t4610 = ct{820};
t4612 = ct{821};
t4613 = ct{822};
t4614 = ct{823};
t4615 = ct{824};
t4617 = ct{825};
t4620 = ct{826};
t4623 = ct{827};
t4625 = ct{828};
t4627 = ct{829};
t4628 = ct{830};
t4629 = ct{831};
t4631 = ct{832};
t4633 = ct{833};
t4634 = ct{834};
t4635 = ct{835};
t4636 = ct{836};
t4638 = ct{837};
t4640 = ct{838};
t4641 = ct{839};
t4642 = ct{840};
t4644 = ct{841};
t4645 = ct{842};
t4647 = ct{843};
t4650 = ct{844};
t4651 = ct{845};
t4652 = ct{846};
t4655 = ct{847};
t4658 = ct{848};
t4659 = ct{849};
t4661 = ct{850};
t4663 = ct{851};
t4664 = ct{852};
t4666 = ct{853};
t4667 = ct{854};
t4669 = ct{855};
t4676 = ct{856};
t4677 = ct{857};
t4678 = ct{858};
t4679 = ct{859};
t4680 = ct{860};
t4682 = ct{861};
t4683 = ct{862};
t4685 = ct{863};
t4686 = ct{864};
t4688 = ct{865};
t4699 = ct{866};
t47 = ct{867};
t4702 = ct{868};
t4703 = ct{869};
t4704 = ct{870};
t4705 = ct{871};
t4706 = ct{872};
t4709 = ct{873};
t4713 = ct{874};
t4715 = ct{875};
t4718 = ct{876};
t4719 = ct{877};
t4720 = ct{878};
t4721 = ct{879};
t4725 = ct{880};
t4727 = ct{881};
t4728 = ct{882};
t4729 = ct{883};
t4732 = ct{884};
t4733 = ct{885};
t4737 = ct{886};
t4738 = ct{887};
t4741 = ct{888};
t4742 = ct{889};
t4744 = ct{890};
t4751 = ct{891};
t4752 = ct{892};
t4753 = ct{893};
t4755 = ct{894};
t4757 = ct{895};
t4758 = ct{896};
t4760 = ct{897};
t4761 = ct{898};
t4762 = ct{899};
t4763 = ct{900};
t4766 = ct{901};
t4767 = ct{902};
t4770 = ct{903};
t4771 = ct{904};
t4772 = ct{905};
t4773 = ct{906};
t4775 = ct{907};
t4777 = ct{908};
t4780 = ct{909};
t4785 = ct{910};
t4786 = ct{911};
t4787 = ct{912};
t4788 = ct{913};
t4789 = ct{914};
t4790 = ct{915};
t4791 = ct{916};
t4792 = ct{917};
t4793 = ct{918};
t4794 = ct{919};
t4795 = ct{920};
t4796 = ct{921};
t4798 = ct{922};
t4799 = ct{923};
t4800 = ct{924};
t4801 = ct{925};
t4805 = ct{926};
t4807 = ct{927};
t4808 = ct{928};
t4809 = ct{929};
t4812 = ct{930};
t4814 = ct{931};
t4816 = ct{932};
t4817 = ct{933};
t4818 = ct{934};
t4819 = ct{935};
t4822 = ct{936};
t4823 = ct{937};
t4824 = ct{938};
t4825 = ct{939};
t4826 = ct{940};
t4829 = ct{941};
t4832 = ct{942};
t4833 = ct{943};
t4835 = ct{944};
t4836 = ct{945};
t4839 = ct{946};
t4840 = ct{947};
t4842 = ct{948};
t4843 = ct{949};
t4845 = ct{950};
t4847 = ct{951};
t4848 = ct{952};
t4849 = ct{953};
t4850 = ct{954};
t4851 = ct{955};
t4852 = ct{956};
t4853 = ct{957};
t4854 = ct{958};
t4855 = ct{959};
t4856 = ct{960};
t4857 = ct{961};
t4858 = ct{962};
t4859 = ct{963};
t4860 = ct{964};
t4865 = ct{965};
t4868 = ct{966};
t4869 = ct{967};
t4870 = ct{968};
t4871 = ct{969};
t4872 = ct{970};
t4873 = ct{971};
t4874 = ct{972};
t4875 = ct{973};
t4880 = ct{974};
t4882 = ct{975};
t4883 = ct{976};
t4884 = ct{977};
t4885 = ct{978};
t4887 = ct{979};
t4890 = ct{980};
t4893 = ct{981};
t4895 = ct{982};
t4896 = ct{983};
t4897 = ct{984};
t4898 = ct{985};
t4899 = ct{986};
t4900 = ct{987};
t4902 = ct{988};
t4904 = ct{989};
t4905 = ct{990};
t4906 = ct{991};
t4907 = ct{992};
t4909 = ct{993};
t4911 = ct{994};
t4913 = ct{995};
t4915 = ct{996};
t4917 = ct{997};
t4918 = ct{998};
t4919 = ct{999};
t4920 = ct{1000};
t4921 = ct{1001};
t4922 = ct{1002};
t4924 = ct{1003};
t4925 = ct{1004};
t4926 = ct{1005};
t4927 = ct{1006};
t4929 = ct{1007};
t4930 = ct{1008};
t4931 = ct{1009};
t4932 = ct{1010};
t4938 = ct{1011};
t4941 = ct{1012};
t4942 = ct{1013};
t4943 = ct{1014};
t4946 = ct{1015};
t4947 = ct{1016};
t4950 = ct{1017};
t4952 = ct{1018};
t4953 = ct{1019};
t4954 = ct{1020};
t4956 = ct{1021};
t4958 = ct{1022};
t4959 = ct{1023};
t4960 = ct{1024};
t4961 = ct{1025};
t4962 = ct{1026};
t4963 = ct{1027};
t4965 = ct{1028};
t4970 = ct{1029};
t4972 = ct{1030};
t4974 = ct{1031};
t4975 = ct{1032};
t4976 = ct{1033};
t4977 = ct{1034};
t4981 = ct{1035};
t4982 = ct{1036};
t4983 = ct{1037};
t4984 = ct{1038};
t4985 = ct{1039};
t4986 = ct{1040};
t4987 = ct{1041};
t4992 = ct{1042};
t4994 = ct{1043};
t4995 = ct{1044};
t4996 = ct{1045};
t4998 = ct{1046};
t5 = ct{1047};
t50 = ct{1048};
t5000 = ct{1049};
t5001 = ct{1050};
t5002 = ct{1051};
t5005 = ct{1052};
t5007 = ct{1053};
t5008 = ct{1054};
t5010 = ct{1055};
t5012 = ct{1056};
t5013 = ct{1057};
t5014 = ct{1058};
t5015 = ct{1059};
t5021 = ct{1060};
t5023 = ct{1061};
t5025 = ct{1062};
t5026 = ct{1063};
t5027 = ct{1064};
t5028 = ct{1065};
t5030 = ct{1066};
t5031 = ct{1067};
t5032 = ct{1068};
t5033 = ct{1069};
t5034 = ct{1070};
t5035 = ct{1071};
t5036 = ct{1072};
t5038 = ct{1073};
t5039 = ct{1074};
t5040 = ct{1075};
t5041 = ct{1076};
t5042 = ct{1077};
t5047 = ct{1078};
t5048 = ct{1079};
t5049 = ct{1080};
t5051 = ct{1081};
t5052 = ct{1082};
t5054 = ct{1083};
t5055 = ct{1084};
t5056 = ct{1085};
t5057 = ct{1086};
t5058 = ct{1087};
t5059 = ct{1088};
t5061 = ct{1089};
t5062 = ct{1090};
t5063 = ct{1091};
t5064 = ct{1092};
t5066 = ct{1093};
t5067 = ct{1094};
t5068 = ct{1095};
t5069 = ct{1096};
t5070 = ct{1097};
t5071 = ct{1098};
t5073 = ct{1099};
t5074 = ct{1100};
t5075 = ct{1101};
t5076 = ct{1102};
t5077 = ct{1103};
t5083 = ct{1104};
t5085 = ct{1105};
t5086 = ct{1106};
t5087 = ct{1107};
t5088 = ct{1108};
t5089 = ct{1109};
t5092 = ct{1110};
t5097 = ct{1111};
t5098 = ct{1112};
t5099 = ct{1113};
t5100 = ct{1114};
t5102 = ct{1115};
t5103 = ct{1116};
t5104 = ct{1117};
t5105 = ct{1118};
t5106 = ct{1119};
t5108 = ct{1120};
t5109 = ct{1121};
t5111 = ct{1122};
t5112 = ct{1123};
t5113 = ct{1124};
t5114 = ct{1125};
t5115 = ct{1126};
t5116 = ct{1127};
t5117 = ct{1128};
t5119 = ct{1129};
t5121 = ct{1130};
t5123 = ct{1131};
t5126 = ct{1132};
t5127 = ct{1133};
t5128 = ct{1134};
t5130 = ct{1135};
t5131 = ct{1136};
t5135 = ct{1137};
t5137 = ct{1138};
t5138 = ct{1139};
t5139 = ct{1140};
t5141 = ct{1141};
t5142 = ct{1142};
t5143 = ct{1143};
t5144 = ct{1144};
t5145 = ct{1145};
t5146 = ct{1146};
t5147 = ct{1147};
t5148 = ct{1148};
t5149 = ct{1149};
t5150 = ct{1150};
t5151 = ct{1151};
t5152 = ct{1152};
t5153 = ct{1153};
t5155 = ct{1154};
t5156 = ct{1155};
t5157 = ct{1156};
t5158 = ct{1157};
t5161 = ct{1158};
t5162 = ct{1159};
t5164 = ct{1160};
t5165 = ct{1161};
t5166 = ct{1162};
t5169 = ct{1163};
t5172 = ct{1164};
t5173 = ct{1165};
t5184 = ct{1166};
t5185 = ct{1167};
t5186 = ct{1168};
t5187 = ct{1169};
t5189 = ct{1170};
t5190 = ct{1171};
t5191 = ct{1172};
t5192 = ct{1173};
t5193 = ct{1174};
t5194 = ct{1175};
t5195 = ct{1176};
t5196 = ct{1177};
t5198 = ct{1178};
t5201 = ct{1179};
t5202 = ct{1180};
t5203 = ct{1181};
t5204 = ct{1182};
t5206 = ct{1183};
t5207 = ct{1184};
t5208 = ct{1185};
t5209 = ct{1186};
t5210 = ct{1187};
t5212 = ct{1188};
t5214 = ct{1189};
t5215 = ct{1190};
t5216 = ct{1191};
t5217 = ct{1192};
t5220 = ct{1193};
t5221 = ct{1194};
t5222 = ct{1195};
t5223 = ct{1196};
t5224 = ct{1197};
t5225 = ct{1198};
t5226 = ct{1199};
t5227 = ct{1200};
t5228 = ct{1201};
t5230 = ct{1202};
t5231 = ct{1203};
t5233 = ct{1204};
t5234 = ct{1205};
t5235 = ct{1206};
t5236 = ct{1207};
t5238 = ct{1208};
t5239 = ct{1209};
t5240 = ct{1210};
t5241 = ct{1211};
t5242 = ct{1212};
t5243 = ct{1213};
t5244 = ct{1214};
t5245 = ct{1215};
t5246 = ct{1216};
t5247 = ct{1217};
t5248 = ct{1218};
t5250 = ct{1219};
t5252 = ct{1220};
t5254 = ct{1221};
t5255 = ct{1222};
t5257 = ct{1223};
t5258 = ct{1224};
t5262 = ct{1225};
t5271 = ct{1226};
t5272 = ct{1227};
t5273 = ct{1228};
t5276 = ct{1229};
t5277 = ct{1230};
t5278 = ct{1231};
t5280 = ct{1232};
t5281 = ct{1233};
t5282 = ct{1234};
t5283 = ct{1235};
t5284 = ct{1236};
t5285 = ct{1237};
t5286 = ct{1238};
t5287 = ct{1239};
t5288 = ct{1240};
t5289 = ct{1241};
t5291 = ct{1242};
t5293 = ct{1243};
t5295 = ct{1244};
t5301 = ct{1245};
t5302 = ct{1246};
t5304 = ct{1247};
t5306 = ct{1248};
t5307 = ct{1249};
t5308 = ct{1250};
t5309 = ct{1251};
t5311 = ct{1252};
t5314 = ct{1253};
t5316 = ct{1254};
t5317 = ct{1255};
t5320 = ct{1256};
t5321 = ct{1257};
t5322 = ct{1258};
t5326 = ct{1259};
t5328 = ct{1260};
t5329 = ct{1261};
t5330 = ct{1262};
t5331 = ct{1263};
t5332 = ct{1264};
t5333 = ct{1265};
t5335 = ct{1266};
t5336 = ct{1267};
t5337 = ct{1268};
t5338 = ct{1269};
t5339 = ct{1270};
t5340 = ct{1271};
t5342 = ct{1272};
t5344 = ct{1273};
t5345 = ct{1274};
t5346 = ct{1275};
t5347 = ct{1276};
t5348 = ct{1277};
t5349 = ct{1278};
t5350 = ct{1279};
t5352 = ct{1280};
t5356 = ct{1281};
t5357 = ct{1282};
t5358 = ct{1283};
t5359 = ct{1284};
t5361 = ct{1285};
t5362 = ct{1286};
t5365 = ct{1287};
t5367 = ct{1288};
t5371 = ct{1289};
t5377 = ct{1290};
t5379 = ct{1291};
t5380 = ct{1292};
t5381 = ct{1293};
t5383 = ct{1294};
t5384 = ct{1295};
t5385 = ct{1296};
t5386 = ct{1297};
t5387 = ct{1298};
t5388 = ct{1299};
t5389 = ct{1300};
t5390 = ct{1301};
t5391 = ct{1302};
t5392 = ct{1303};
t5393 = ct{1304};
t5395 = ct{1305};
t5396 = ct{1306};
t5397 = ct{1307};
t5399 = ct{1308};
t5400 = ct{1309};
t5402 = ct{1310};
t5403 = ct{1311};
t5405 = ct{1312};
t5407 = ct{1313};
t5408 = ct{1314};
t5409 = ct{1315};
t5411 = ct{1316};
t5412 = ct{1317};
t5413 = ct{1318};
t5414 = ct{1319};
t5416 = ct{1320};
t5418 = ct{1321};
t5419 = ct{1322};
t5420 = ct{1323};
t5423 = ct{1324};
t5424 = ct{1325};
t5426 = ct{1326};
t5427 = ct{1327};
t5428 = ct{1328};
t5429 = ct{1329};
t5430 = ct{1330};
t5432 = ct{1331};
t5433 = ct{1332};
t5434 = ct{1333};
t5435 = ct{1334};
t5437 = ct{1335};
t5438 = ct{1336};
t5440 = ct{1337};
t5441 = ct{1338};
t5443 = ct{1339};
t5444 = ct{1340};
t5445 = ct{1341};
t5446 = ct{1342};
t5447 = ct{1343};
t5448 = ct{1344};
t5449 = ct{1345};
t5450 = ct{1346};
t5451 = ct{1347};
t5452 = ct{1348};
t5453 = ct{1349};
t5454 = ct{1350};
t5455 = ct{1351};
t5456 = ct{1352};
t5457 = ct{1353};
t5458 = ct{1354};
t5459 = ct{1355};
t5461 = ct{1356};
t5462 = ct{1357};
t5464 = ct{1358};
t5465 = ct{1359};
t5466 = ct{1360};
t5467 = ct{1361};
t5468 = ct{1362};
t5469 = ct{1363};
t5473 = ct{1364};
t5474 = ct{1365};
t5476 = ct{1366};
t5477 = ct{1367};
t5479 = ct{1368};
t5480 = ct{1369};
t5481 = ct{1370};
t5482 = ct{1371};
t5483 = ct{1372};
t5484 = ct{1373};
t5485 = ct{1374};
t5486 = ct{1375};
t5487 = ct{1376};
t5488 = ct{1377};
t5489 = ct{1378};
t5490 = ct{1379};
t5491 = ct{1380};
t5492 = ct{1381};
t5493 = ct{1382};
t5494 = ct{1383};
t5496 = ct{1384};
t5498 = ct{1385};
t5499 = ct{1386};
t5500 = ct{1387};
t5503 = ct{1388};
t5504 = ct{1389};
t5505 = ct{1390};
t5506 = ct{1391};
t5507 = ct{1392};
t5509 = ct{1393};
t5512 = ct{1394};
t5513 = ct{1395};
t5514 = ct{1396};
t5515 = ct{1397};
t5516 = ct{1398};
t5517 = ct{1399};
t5518 = ct{1400};
t5520 = ct{1401};
t5521 = ct{1402};
t5522 = ct{1403};
t5523 = ct{1404};
t5524 = ct{1405};
t5525 = ct{1406};
t5526 = ct{1407};
t5528 = ct{1408};
t5530 = ct{1409};
t5531 = ct{1410};
t5532 = ct{1411};
t5533 = ct{1412};
t5534 = ct{1413};
t5535 = ct{1414};
t5536 = ct{1415};
t5537 = ct{1416};
t5538 = ct{1417};
t5539 = ct{1418};
t5541 = ct{1419};
t5542 = ct{1420};
t5543 = ct{1421};
t5544 = ct{1422};
t5545 = ct{1423};
t5546 = ct{1424};
t5547 = ct{1425};
t5550 = ct{1426};
t5551 = ct{1427};
t5552 = ct{1428};
t5553 = ct{1429};
t5554 = ct{1430};
t5556 = ct{1431};
t5557 = ct{1432};
t5558 = ct{1433};
t5559 = ct{1434};
t5561 = ct{1435};
t5563 = ct{1436};
t5564 = ct{1437};
t5566 = ct{1438};
t5568 = ct{1439};
t5569 = ct{1440};
t5570 = ct{1441};
t5573 = ct{1442};
t5574 = ct{1443};
t5575 = ct{1444};
t5576 = ct{1445};
t5577 = ct{1446};
t5578 = ct{1447};
t5579 = ct{1448};
t5580 = ct{1449};
t5581 = ct{1450};
t5582 = ct{1451};
t5583 = ct{1452};
t5585 = ct{1453};
t5588 = ct{1454};
t5589 = ct{1455};
t5590 = ct{1456};
t5592 = ct{1457};
t5593 = ct{1458};
t5594 = ct{1459};
t5595 = ct{1460};
t5596 = ct{1461};
t5597 = ct{1462};
t56 = ct{1463};
t5600 = ct{1464};
t5601 = ct{1465};
t5602 = ct{1466};
t5603 = ct{1467};
t5604 = ct{1468};
t5605 = ct{1469};
t5606 = ct{1470};
t5610 = ct{1471};
t5615 = ct{1472};
t5617 = ct{1473};
t5619 = ct{1474};
t5620 = ct{1475};
t5621 = ct{1476};
t5622 = ct{1477};
t5623 = ct{1478};
t5624 = ct{1479};
t5625 = ct{1480};
t5626 = ct{1481};
t5627 = ct{1482};
t5628 = ct{1483};
t5629 = ct{1484};
t5631 = ct{1485};
t5632 = ct{1486};
t5635 = ct{1487};
t5636 = ct{1488};
t5639 = ct{1489};
t5641 = ct{1490};
t5644 = ct{1491};
t5648 = ct{1492};
t5651 = ct{1493};
t5653 = ct{1494};
t5655 = ct{1495};
t5658 = ct{1496};
t5659 = ct{1497};
t5660 = ct{1498};
t5661 = ct{1499};
t5662 = ct{1500};
t5663 = ct{1501};
t5664 = ct{1502};
t5665 = ct{1503};
t5666 = ct{1504};
t5667 = ct{1505};
t5670 = ct{1506};
t5671 = ct{1507};
t5674 = ct{1508};
t5675 = ct{1509};
t5678 = ct{1510};
t5679 = ct{1511};
t5680 = ct{1512};
t5681 = ct{1513};
t5682 = ct{1514};
t5685 = ct{1515};
t5686 = ct{1516};
t5687 = ct{1517};
t5689 = ct{1518};
t5691 = ct{1519};
t5693 = ct{1520};
t5694 = ct{1521};
t5695 = ct{1522};
t5696 = ct{1523};
t5698 = ct{1524};
t5699 = ct{1525};
t5700 = ct{1526};
t5701 = ct{1527};
t5702 = ct{1528};
t5703 = ct{1529};
t5704 = ct{1530};
t5705 = ct{1531};
t5706 = ct{1532};
t5707 = ct{1533};
t5708 = ct{1534};
t5709 = ct{1535};
t5711 = ct{1536};
t5712 = ct{1537};
t5714 = ct{1538};
t5715 = ct{1539};
t5717 = ct{1540};
t5718 = ct{1541};
t5720 = ct{1542};
t5721 = ct{1543};
t5722 = ct{1544};
t5723 = ct{1545};
t5725 = ct{1546};
t5726 = ct{1547};
t5727 = ct{1548};
t5728 = ct{1549};
t5730 = ct{1550};
t5731 = ct{1551};
t5733 = ct{1552};
t5735 = ct{1553};
t5737 = ct{1554};
t5739 = ct{1555};
t5740 = ct{1556};
t5741 = ct{1557};
t5742 = ct{1558};
t5748 = ct{1559};
t5749 = ct{1560};
t5750 = ct{1561};
t5751 = ct{1562};
t5756 = ct{1563};
t5757 = ct{1564};
t5760 = ct{1565};
t5761 = ct{1566};
t5762 = ct{1567};
t5764 = ct{1568};
t5765 = ct{1569};
t5768 = ct{1570};
t5770 = ct{1571};
t5771 = ct{1572};
t5772 = ct{1573};
t5773 = ct{1574};
t5775 = ct{1575};
t5776 = ct{1576};
t5777 = ct{1577};
t5778 = ct{1578};
t5779 = ct{1579};
t5780 = ct{1580};
t5782 = ct{1581};
t5783 = ct{1582};
t5785 = ct{1583};
t5786 = ct{1584};
t5787 = ct{1585};
t5788 = ct{1586};
t5791 = ct{1587};
t5792 = ct{1588};
t5793 = ct{1589};
t5794 = ct{1590};
t5796 = ct{1591};
t5798 = ct{1592};
t5799 = ct{1593};
t5804 = ct{1594};
t5805 = ct{1595};
t5807 = ct{1596};
t5808 = ct{1597};
t5809 = ct{1598};
t5813 = ct{1599};
t5815 = ct{1600};
t5816 = ct{1601};
t5818 = ct{1602};
t5820 = ct{1603};
t5821 = ct{1604};
t5824 = ct{1605};
t5825 = ct{1606};
t5828 = ct{1607};
t5829 = ct{1608};
t5831 = ct{1609};
t5832 = ct{1610};
t5833 = ct{1611};
t5835 = ct{1612};
t5836 = ct{1613};
t5838 = ct{1614};
t5840 = ct{1615};
t5842 = ct{1616};
t5843 = ct{1617};
t5845 = ct{1618};
t5846 = ct{1619};
t5850 = ct{1620};
t5851 = ct{1621};
t5852 = ct{1622};
t5853 = ct{1623};
t5854 = ct{1624};
t5855 = ct{1625};
t5857 = ct{1626};
t5858 = ct{1627};
t5859 = ct{1628};
t5860 = ct{1629};
t5861 = ct{1630};
t5862 = ct{1631};
t5863 = ct{1632};
t5864 = ct{1633};
t5865 = ct{1634};
t5866 = ct{1635};
t5868 = ct{1636};
t5870 = ct{1637};
t5871 = ct{1638};
t5873 = ct{1639};
t5876 = ct{1640};
t5877 = ct{1641};
t5879 = ct{1642};
t5881 = ct{1643};
t5882 = ct{1644};
t5883 = ct{1645};
t5884 = ct{1646};
t5887 = ct{1647};
t5888 = ct{1648};
t5889 = ct{1649};
t5890 = ct{1650};
t5891 = ct{1651};
t5894 = ct{1652};
t5896 = ct{1653};
t5899 = ct{1654};
t5900 = ct{1655};
t5902 = ct{1656};
t5904 = ct{1657};
t5907 = ct{1658};
t5908 = ct{1659};
t5910 = ct{1660};
t5911 = ct{1661};
t5912 = ct{1662};
t5913 = ct{1663};
t5914 = ct{1664};
t5916 = ct{1665};
t5917 = ct{1666};
t5918 = ct{1667};
t5922 = ct{1668};
t5923 = ct{1669};
t5924 = ct{1670};
t5926 = ct{1671};
t5927 = ct{1672};
t5929 = ct{1673};
t5930 = ct{1674};
t5932 = ct{1675};
t5933 = ct{1676};
t5935 = ct{1677};
t5937 = ct{1678};
t5940 = ct{1679};
t5943 = ct{1680};
t5944 = ct{1681};
t5945 = ct{1682};
t5947 = ct{1683};
t5951 = ct{1684};
t5952 = ct{1685};
t5953 = ct{1686};
t5954 = ct{1687};
t5956 = ct{1688};
t5957 = ct{1689};
t5958 = ct{1690};
t5959 = ct{1691};
t5960 = ct{1692};
t5963 = ct{1693};
t5966 = ct{1694};
t5968 = ct{1695};
t5969 = ct{1696};
t5970 = ct{1697};
t5972 = ct{1698};
t5975 = ct{1699};
t5977 = ct{1700};
t5978 = ct{1701};
t5979 = ct{1702};
t5980 = ct{1703};
t5981 = ct{1704};
t5986 = ct{1705};
t5988 = ct{1706};
t5991 = ct{1707};
t5992 = ct{1708};
t5994 = ct{1709};
t5996 = ct{1710};
t5997 = ct{1711};
t5998 = ct{1712};
t6 = ct{1713};
t60 = ct{1714};
t6000 = ct{1715};
t6001 = ct{1716};
t6002 = ct{1717};
t6004 = ct{1718};
t6008 = ct{1719};
t6009 = ct{1720};
t6010 = ct{1721};
t6012 = ct{1722};
t6015 = ct{1723};
t6016 = ct{1724};
t6017 = ct{1725};
t6018 = ct{1726};
t6019 = ct{1727};
t6020 = ct{1728};
t6021 = ct{1729};
t6028 = ct{1730};
t6030 = ct{1731};
t6031 = ct{1732};
t6034 = ct{1733};
t6035 = ct{1734};
t6038 = ct{1735};
t6039 = ct{1736};
t6042 = ct{1737};
t6043 = ct{1738};
t6046 = ct{1739};
t6047 = ct{1740};
t6049 = ct{1741};
t6050 = ct{1742};
t6051 = ct{1743};
t6054 = ct{1744};
t6057 = ct{1745};
t6058 = ct{1746};
t6060 = ct{1747};
t6062 = ct{1748};
t6064 = ct{1749};
t6066 = ct{1750};
t6067 = ct{1751};
t6075 = ct{1752};
t6076 = ct{1753};
t6087 = ct{1754};
t6088 = ct{1755};
t6091 = ct{1756};
t6092 = ct{1757};
t6095 = ct{1758};
t6096 = ct{1759};
t6100 = ct{1760};
t6101 = ct{1761};
t6103 = ct{1762};
t6104 = ct{1763};
t6112 = ct{1764};
t6119 = ct{1765};
t6135 = ct{1766};
t6137 = ct{1767};
t6138 = ct{1768};
t6140 = ct{1769};
t6143 = ct{1770};
t6144 = ct{1771};
t6147 = ct{1772};
t6150 = ct{1773};
t6151 = ct{1774};
t6156 = ct{1775};
t6160 = ct{1776};
t6161 = ct{1777};
t6162 = ct{1778};
t6165 = ct{1779};
t6168 = ct{1780};
t6169 = ct{1781};
t6173 = ct{1782};
t6175 = ct{1783};
t6183 = ct{1784};
t6184 = ct{1785};
t6185 = ct{1786};
t6189 = ct{1787};
t6198 = ct{1788};
t6199 = ct{1789};
t6200 = ct{1790};
t6201 = ct{1791};
t6202 = ct{1792};
t6206 = ct{1793};
t6207 = ct{1794};
t6209 = ct{1795};
t6210 = ct{1796};
t6211 = ct{1797};
t6219 = ct{1798};
t6221 = ct{1799};
t6223 = ct{1800};
t6224 = ct{1801};
t6232 = ct{1802};
t6238 = ct{1803};
t6244 = ct{1804};
t6245 = ct{1805};
t6247 = ct{1806};
t6248 = ct{1807};
t6251 = ct{1808};
t6253 = ct{1809};
t6257 = ct{1810};
t6267 = ct{1811};
t6271 = ct{1812};
t6279 = ct{1813};
t6280 = ct{1814};
t6282 = ct{1815};
t6285 = ct{1816};
t6293 = ct{1817};
t6297 = ct{1818};
t6298 = ct{1819};
t6302 = ct{1820};
t6303 = ct{1821};
t6304 = ct{1822};
t6305 = ct{1823};
t6307 = ct{1824};
t6308 = ct{1825};
t6311 = ct{1826};
t6313 = ct{1827};
t6315 = ct{1828};
t6317 = ct{1829};
t6321 = ct{1830};
t6322 = ct{1831};
t6323 = ct{1832};
t6327 = ct{1833};
t6331 = ct{1834};
t6338 = ct{1835};
t6339 = ct{1836};
t6341 = ct{1837};
t6343 = ct{1838};
t6344 = ct{1839};
t6348 = ct{1840};
t6349 = ct{1841};
t6354 = ct{1842};
t6356 = ct{1843};
t6357 = ct{1844};
t6359 = ct{1845};
t6360 = ct{1846};
t6365 = ct{1847};
t6366 = ct{1848};
t6367 = ct{1849};
t6369 = ct{1850};
t6375 = ct{1851};
t6378 = ct{1852};
t6387 = ct{1853};
t6388 = ct{1854};
t6389 = ct{1855};
t6394 = ct{1856};
t6396 = ct{1857};
t6397 = ct{1858};
t640 = ct{1859};
t6400 = ct{1860};
t6406 = ct{1861};
t6407 = ct{1862};
t6408 = ct{1863};
t6411 = ct{1864};
t6414 = ct{1865};
t642 = ct{1866};
t6427 = ct{1867};
t643 = ct{1868};
t6431 = ct{1869};
t6436 = ct{1870};
t6437 = ct{1871};
t6441 = ct{1872};
t6442 = ct{1873};
t6450 = ct{1874};
t6451 = ct{1875};
t6452 = ct{1876};
t6453 = ct{1877};
t6455 = ct{1878};
t6456 = ct{1879};
t6463 = ct{1880};
t6464 = ct{1881};
t6473 = ct{1882};
t6480 = ct{1883};
t6481 = ct{1884};
t6483 = ct{1885};
t6484 = ct{1886};
t6485 = ct{1887};
t6486 = ct{1888};
t6489 = ct{1889};
t649 = ct{1890};
t6490 = ct{1891};
t6492 = ct{1892};
t6493 = ct{1893};
t6497 = ct{1894};
t6507 = ct{1895};
t6508 = ct{1896};
t6511 = ct{1897};
t6515 = ct{1898};
t6518 = ct{1899};
t6519 = ct{1900};
t6521 = ct{1901};
t6523 = ct{1902};
t6528 = ct{1903};
t6529 = ct{1904};
t6533 = ct{1905};
t6534 = ct{1906};
t6539 = ct{1907};
t6543 = ct{1908};
t6544 = ct{1909};
t6545 = ct{1910};
t656 = ct{1911};
t6565 = ct{1912};
t6566 = ct{1913};
t6568 = ct{1914};
t6570 = ct{1915};
t6572 = ct{1916};
t6573 = ct{1917};
t6574 = ct{1918};
t6575 = ct{1919};
t6584 = ct{1920};
t6585 = ct{1921};
t6586 = ct{1922};
t659 = ct{1923};
t6591 = ct{1924};
t6593 = ct{1925};
t660 = ct{1926};
t6600 = ct{1927};
t6603 = ct{1928};
t6604 = ct{1929};
t6611 = ct{1930};
t6612 = ct{1931};
t6634 = ct{1932};
t6635 = ct{1933};
t6658 = ct{1934};
t6660 = ct{1935};
t6663 = ct{1936};
t6664 = ct{1937};
t667 = ct{1938};
t668 = ct{1939};
t6689 = ct{1940};
t669 = ct{1941};
t6691 = ct{1942};
t6692 = ct{1943};
t67 = ct{1944};
t670 = ct{1945};
t6703 = ct{1946};
t6706 = ct{1947};
t674 = ct{1948};
t6752 = ct{1949};
t6753 = ct{1950};
t6763 = ct{1951};
t6764 = ct{1952};
t677 = ct{1953};
t6776 = ct{1954};
t6777 = ct{1955};
t6789 = ct{1956};
t6793 = ct{1957};
t6794 = ct{1958};
t6796 = ct{1959};
t6797 = ct{1960};
t68 = ct{1961};
t6804 = ct{1962};
t6805 = ct{1963};
t6807 = ct{1964};
t681 = ct{1965};
t6811 = ct{1966};
t6812 = ct{1967};
t6813 = ct{1968};
t6814 = ct{1969};
t6815 = ct{1970};
t682 = ct{1971};
t684 = ct{1972};
t685 = ct{1973};
t686 = ct{1974};
t6860 = ct{1975};
t6861 = ct{1976};
t687 = ct{1977};
t6873 = ct{1978};
t6885 = ct{1979};
t6887 = ct{1980};
t6888 = ct{1981};
t6890 = ct{1982};
t6892 = ct{1983};
t6893 = ct{1984};
t6909 = ct{1985};
t6913 = ct{1986};
t6916 = ct{1987};
t6917 = ct{1988};
t6920 = ct{1989};
t6924 = ct{1990};
t6925 = ct{1991};
t6926 = ct{1992};
t6927 = ct{1993};
t6928 = ct{1994};
t6937 = ct{1995};
t694 = ct{1996};
t6954 = ct{1997};
t6955 = ct{1998};
t6958 = ct{1999};
t6972 = ct{2000};
t6975 = ct{2001};
t6979 = ct{2002};
t6984 = ct{2003};
t6986 = ct{2004};
t6987 = ct{2005};
t6988 = ct{2006};
t6989 = ct{2007};
t6990 = ct{2008};
t6992 = ct{2009};
t6993 = ct{2010};
t7 = ct{2011};
t7012 = ct{2012};
t7015 = ct{2013};
t7027 = ct{2014};
t7028 = ct{2015};
t7029 = ct{2016};
t7039 = ct{2017};
t7041 = ct{2018};
t7044 = ct{2019};
t7046 = ct{2020};
t7049 = ct{2021};
t7050 = ct{2022};
t7051 = ct{2023};
t7053 = ct{2024};
t7054 = ct{2025};
t7055 = ct{2026};
t7056 = ct{2027};
t7057 = ct{2028};
t7058 = ct{2029};
t7062 = ct{2030};
t7065 = ct{2031};
t707 = ct{2032};
t708 = ct{2033};
t7091 = ct{2034};
t71 = ct{2035};
t710 = ct{2036};
t7107 = ct{2037};
t715 = ct{2038};
t716 = ct{2039};
t7181 = ct{2040};
t7193 = ct{2041};
t7204 = ct{2042};
t721 = ct{2043};
t7219 = ct{2044};
t722 = ct{2045};
t7228 = ct{2046};
t7229 = ct{2047};
t724 = ct{2048};
t725 = ct{2049};
t7280 = ct{2050};
t7291 = ct{2051};
t7292 = ct{2052};
t7294 = ct{2053};
t73 = ct{2054};
t736 = ct{2055};
t740 = ct{2056};
t741 = ct{2057};
t749 = ct{2058};
t762 = ct{2059};
t768 = ct{2060};
t7723 = ct{2061};
t7731 = ct{2062};
t7732 = ct{2063};
t7734 = ct{2064};
t777 = ct{2065};
t7790 = ct{2066};
t792 = ct{2067};
t793 = ct{2068};
t801 = ct{2069};
t802 = ct{2070};
t808 = ct{2071};
t813 = ct{2072};
t819 = ct{2073};
t821 = ct{2074};
t850 = ct{2075};
t855 = ct{2076};
t874 = ct{2077};
t878 = ct{2078};
t89 = ct{2079};
t92 = ct{2080};
t941 = ct{2081};
t948 = ct{2082};
t951 = ct{2083};
t97 = ct{2084};
t7068 = -t5258.*(t4795.*(t1896-t3232).*7.26735e-3+t2363.*(t684+t685-t710+t724+t1686-t1690+t1700+t1701+t2371+t2698+t2707-t2716+t2719+t3319-t3327-t3341-t3620+t3622+t3634-t3638+t4076+t4077).*7.26735e-3);
t7089 = (t4758.*(t1861-t3214)+t2297.*(t642+t643-t667+t674+t1587+t1606+t1608+t1609+t2295+t2671+t2683+t2684-t2695+t3272+t3290-t3296+t3576+t3582+t3588-t3593+t4015+t4016)).*(t3547.*1.33637554986e-4+t4119-t4120+t34.*(t1896-t3232).*7.26350557185e-5);
t7092 = t2363.*t7065.*7.26735e-3;
et232 = t4795.*(t1896-t3232).*7.26735e-3+t2363.*(t684+t685-t710+t724+t1686-t1690+t1700+t1701+t2371+t2698+t2707-t2716+t2719+t3319-t3327-t3341-t3620+t3622+t3634-t3638+t4076+t4077).*7.26735e-3;
et233 = -t4007+t4011+t18.*(t1861-t3214).*1.838876e-2+t23.*(t1861-t3214).*9.99471e-3;
t7094 = et232.*et233;
t7099 = t4822.*(t4795.*(t1896-t3232).*7.26735e-3+t2363.*(t684+t685-t710+t724+t1686-t1690+t1700+t1701+t2371+t2698+t2707-t2716+t2719+t3319-t3327-t3341-t3620+t3622+t3634-t3638+t4076+t4077).*7.26735e-3).*(t1488+t1874+t2519+t2740+t2747+t3096+t3097);
et234 = -t2306-t2317+t3144+t3147+t35.*t941.*t948.*(t850-t874).*3.775747223193135e-1;
et235 = t36.*t941.*t948.*(t850-t874).*2.244797987218524e-1;
t7108 = -t6975.*(et234+et235);
t7114 = -t5737.*(t4758.*(t1861-t3214)+t2297.*(t642+t643-t667+t674+t1587+t1606+t1608+t1609+t2295+t2671+t2683+t2684-t2695+t3272+t3290-t3296+t3576+t3582+t3588-t3593+t4015+t4016));
t7151 = (t4610+t2363.*(t3547.*1.838876e-2+t4071-t4072+t34.*(t1896-t3232).*9.99471e-3).*7.26735e-3).*(t4758.*(t1861-t3214)+t2297.*(t642+t643-t667+t674+t1587+t1606+t1608+t1609+t2295+t2671+t2683+t2684-t2695+t3272+t3290-t3296+t3576+t3582+t3588-t3593+t4015+t4016));
t7157 = (t5359+t4108.*(t1861-t3214)).*(t4795.*(t1896-t3232).*7.26735e-3+t2363.*(t684+t685-t710+t724+t1686-t1690+t1700+t1701+t2371+t2698+t2707-t2716+t2719+t3319-t3327-t3341-t3620+t3622+t3634-t3638+t4076+t4077).*7.26735e-3);
t7174 = t3017+t3079+t3155+t3166+t4424+t4427+t4473+t4475+t4709+t4713+t5010+t5012;
t7178 = t5194+t5208+t5214+t5216+t5765;
t7179 = t5193+t5212+t5215+t5217+t5768;
t7180 = t5468+t6000+t6012;
t7184 = -t5975.*(t4795.*(t1896-t3232).*7.26735e-3+t2363.*(t684+t685-t710+t724+t1686-t1690+t1700+t1701+t2371+t2698+t2707-t2716+t2719+t3319-t3327-t3341-t3620+t3622+t3634-t3638+t4076+t4077).*7.26735e-3);
t7185 = t5975.*(t4795.*(t1896-t3232).*7.26735e-3+t2363.*(t684+t685-t710+t724+t1686-t1690+t1700+t1701+t2371+t2698+t2707-t2716+t2719+t3319-t3327-t3341-t3620+t3622+t3634-t3638+t4076+t4077).*7.26735e-3);
et236 = t5001+t5097+t5098+t5295.*(-t2804+t2838+t3109+t23.*(t1456-t2355).*9.3e-7)+t3063.*(t3235-t3535);
et237 = (t4840-t34.*(t1005+t26.*(t1941-t3308+t39.*t1022.*(t855-t878).*2.196325630278387e-1))).*(t2813-t2835+t18.*(t1456-t2355).*1.02e-6+t23.*(t1456-t2355).*9.0e-8);
t7194 = -t3209.*(et236+et237);
et238 = t5001+t5097+t5098+t5295.*(-t2804+t2838+t3109+t23.*(t1456-t2355).*9.3e-7)+t3063.*(t3235-t3535);
et239 = (t4840-t34.*(t1005+t26.*(t1941-t3308+t39.*t1022.*(t855-t878).*2.196325630278387e-1))).*(t2813-t2835+t18.*(t1456-t2355).*1.02e-6+t23.*(t1456-t2355).*9.0e-8);
t7195 = t3209.*(et238+et239);
t7198 = t2363.*t7193;
et240 = t5001+t5097+t5098+t5295.*(-t2804+t2838+t3109+t23.*(t1456-t2355).*9.3e-7)+t3063.*(t3235-t3535);
et241 = (t4840-t34.*(t1005+t26.*(t1941-t3308+t39.*t1022.*(t855-t878).*2.196325630278387e-1))).*(t2813-t2835+t18.*(t1456-t2355).*1.02e-6+t23.*(t1456-t2355).*9.0e-8);
t7200 = (et240+et241).*(t1861-t3214);
et242 = t5001+t5097+t5098+t5295.*(-t2804+t2838+t3109+t23.*(t1456-t2355).*9.3e-7)+t3063.*(t3235-t3535);
et243 = (t4840-t34.*(t1005+t26.*(t1941-t3308+t39.*t1022.*(t855-t878).*2.196325630278387e-1))).*(t2813-t2835+t18.*(t1456-t2355).*1.02e-6+t23.*(t1456-t2355).*9.0e-8);
t7209 = (et242+et243).*(t2674-t2676+t3022-t3027);
t7210 = -t7193.*(t1896-t3232);
t7211 = t3528.*t7193;
et244 = t5001+t5097+t5098+t5295.*(-t2804+t2838+t3109+t23.*(t1456-t2355).*9.3e-7)+t3063.*(t3235-t3535);
et245 = (t4840-t34.*(t1005+t26.*(t1941-t3308+t39.*t1022.*(t855-t878).*2.196325630278387e-1))).*(t2813-t2835+t18.*(t1456-t2355).*1.02e-6+t23.*(t1456-t2355).*9.0e-8);
t7214 = -t3946.*(et244+et245);
et246 = t5001+t5097+t5098+t5295.*(-t2804+t2838+t3109+t23.*(t1456-t2355).*9.3e-7)+t3063.*(t3235-t3535);
et247 = (t4840-t34.*(t1005+t26.*(t1941-t3308+t39.*t1022.*(t855-t878).*2.196325630278387e-1))).*(t2813-t2835+t18.*(t1456-t2355).*1.02e-6+t23.*(t1456-t2355).*9.0e-8);
t7215 = t3946.*(et246+et247);
t7222 = -t3057.*(t3130+t3131+t3170+t3435-t4238-t4239-t4257+t4259-t4264+t4266-t4520-t4531+t4560+t4576+t2388.*(t1456-t2355).*4.0e-8+(t3524.*(t1861-t3214))./1.0e+8+(t3481.*(t1896-t3232))./1.0e+8-t17.*t2297.*t2363.*2.4e-7);
et248 = (t4785+t5058+t2307.*(t642+t643-t667+t674+t1587+t1606+t1608+t1609+t2295+t2671+t2683+t2684-t2695+t3272+t3290-t3296+t3576+t3582+t3588-t3593+t4015+t4016)+t2297.*(t2292+t3283+t3505.*1.838876e-2-t3570+t3571+t3590+t22.*(t1861-t3214).*3.131399999999998e-4+t22.*t23.*(t1861-t3214).*9.99471e-3)).*(t2694-t2701+t3036-t3043).*(t1513+t1879+t2598+t2820+t2834+t3117+t3118);
et249 = -7.26735e-3;
t7231 = et248.*et249;
et250 = (t4785+t5058+t2307.*(t642+t643-t667+t674+t1587+t1606+t1608+t1609+t2295+t2671+t2683+t2684-t2695+t3272+t3290-t3296+t3576+t3582+t3588-t3593+t4015+t4016)+t2297.*(t2292+t3283+t3505.*1.838876e-2-t3570+t3571+t3590+t22.*(t1861-t3214).*3.131399999999998e-4+t22.*t23.*(t1861-t3214).*9.99471e-3)).*(t2694-t2701+t3036-t3043).*(t1513+t1879+t2598+t2820+t2834+t3117+t3118);
et251 = 7.26735e-3;
t7232 = et250.*et251;
t7233 = t5322+t5330+t5333+t5336+t5969;
t7236 = (t3235-t3535).*(t3130+t3131+t3170+t3435-t4238-t4239-t4257+t4259-t4264+t4266-t4520-t4531+t4560+t4576+t2388.*(t1456-t2355).*4.0e-8+(t3524.*(t1861-t3214))./1.0e+8+(t3481.*(t1896-t3232))./1.0e+8-t17.*t2297.*t2363.*2.4e-7);
t7237 = -t3992.*(t3130+t3131+t3170+t3435-t4238-t4239-t4257+t4259-t4264+t4266-t4520-t4531+t4560+t4576+t2388.*(t1456-t2355).*4.0e-8+(t3524.*(t1861-t3214))./1.0e+8+(t3481.*(t1896-t3232))./1.0e+8-t17.*t2297.*t2363.*2.4e-7);
t7239 = t3992.*(t3130+t3131+t3170+t3435-t4238-t4239-t4257+t4259-t4264+t4266-t4520-t4531+t4560+t4576+t2388.*(t1456-t2355).*4.0e-8+(t3524.*(t1861-t3214))./1.0e+8+(t3481.*(t1896-t3232))./1.0e+8-t17.*t2297.*t2363.*2.4e-7);
t7241 = t3187+t3188+t3194+t3201+t4728+t4760+t4762+t4766+t5015+t5021+t5026+t5028;
et252 = t2363.*(t2368+t3330+t3563.*1.838876e-2-t3618+t3619+t27.*(t1896-t3232).*1.247162e-2+t33.*(t1896-t3232).*3.131399999999998e-4+t33.*t34.*(t1896-t3232).*9.99471e-3);
et253 = 7.26735e-3;
t7244 = -(t4872+t5144+et252.*et253+t2388.*(t684+t685-t710+t724+t1686-t1690+t1700+t1701+t2371+t2698+t2707-t2716+t2719+t3319-t3327-t3341-t3620+t3622+t3634-t3638+t4076+t4077).*7.26735e-3).*(t2674-t2676+t3022-t3027).*(t1488+t1874+t2519+t2740+t2747+t3096+t3097);
et254 = t2363.*(t2368+t3330+t3563.*1.838876e-2-t3618+t3619+t27.*(t1896-t3232).*1.247162e-2+t33.*(t1896-t3232).*3.131399999999998e-4+t33.*t34.*(t1896-t3232).*9.99471e-3);
et255 = 7.26735e-3;
t7245 = (t4872+t5144+et254.*et255+t2388.*(t684+t685-t710+t724+t1686-t1690+t1700+t1701+t2371+t2698+t2707-t2716+t2719+t3319-t3327-t3341-t3620+t3622+t3634-t3638+t4076+t4077).*7.26735e-3).*(t2674-t2676+t3022-t3027).*(t1488+t1874+t2519+t2740+t2747+t3096+t3097);
t7248 = -(t1477-t2502).*(-t3184-t3191-t3199+t4728+t4760+t4762+t4766+t5015+t5021+t5026+t5028-t201.*(t1456-t2355).*4.899491877593981e-7);
t7256 = -(t4795.*(t1896-t3232).*7.26735e-3+t2363.*(t684+t685-t710+t724+t1686-t1690+t1700+t1701+t2371+t2698+t2707-t2716+t2719+t3319-t3327-t3341-t3620+t3622+t3634-t3638+t4076+t4077).*7.26735e-3).*(-t2308+t2378+t2510-t2530-t2975+t2979+t3893+t4106+t4152+t4155+t4805+t4809);
t7257 = (t4795.*(t1896-t3232).*7.26735e-3+t2363.*(t684+t685-t710+t724+t1686-t1690+t1700+t1701+t2371+t2698+t2707-t2716+t2719+t3319-t3327-t3341-t3620+t3622+t3634-t3638+t4076+t4077).*7.26735e-3).*(-t2308+t2378+t2510-t2530-t2975+t2979+t3893+t4106+t4152+t4155+t4805+t4809);
t7259 = -t6565.*(t4758.*(t1861-t3214)+t2297.*(t642+t643-t667+t674+t1587+t1606+t1608+t1609+t2295+t2671+t2683+t2684-t2695+t3272+t3290-t3296+t3576+t3582+t3588-t3593+t4015+t4016));
t7263 = t3985.*(-t3184-t3191-t3199+t4728+t4760+t4762+t4766+t5015+t5021+t5026+t5028-t201.*(t1456-t2355).*4.899491877593981e-7);
t7265 = t3996.*(-t3184-t3191-t3199+t4728+t4760+t4762+t4766+t5015+t5021+t5026+t5028-t201.*(t1456-t2355).*4.899491877593981e-7);
t7269 = t3316+t3344+t3451+t3453+t4880+t4887+t4893+t4895+t5115+t5123+t5127+t5130;
t7272 = t5408+t5467+t5469+t5477+t6015;
t7273 = t5409+t5473+t5474+t5476+t6016;
t7274 = t4832+t4839+t5165+t5169+t5221+t5222+t5271+t5272;
t7293 = -t7291;
t7328 = (t1477-t2502).*(t5231+t5235-t5273+t5278+t5282-t5285+t4777.*(t2694-t2701+t3036-t3043).*5.7e-7+t4780.*(t2694-t2701+t3036-t3043).*4.0e-8);
t7348 = -t3985.*(t5231+t5235-t5273+t5278+t5282-t5285+t4777.*(t2694-t2701+t3036-t3043).*5.7e-7+t4780.*(t2694-t2701+t3036-t3043).*4.0e-8);
t7349 = t3985.*(t5231+t5235-t5273+t5278+t5282-t5285+t4777.*(t2694-t2701+t3036-t3043).*5.7e-7+t4780.*(t2694-t2701+t3036-t3043).*4.0e-8);
t7350 = -t3996.*(t5231+t5235-t5273+t5278+t5282-t5285+t4777.*(t2694-t2701+t3036-t3043).*5.7e-7+t4780.*(t2694-t2701+t3036-t3043).*4.0e-8);
et256 = t4795.*(t1896-t3232).*7.26735e-3+t2363.*(t684+t685-t710+t724+t1686-t1690+t1700+t1701+t2371+t2698+t2707-t2716+t2719+t3319-t3327-t3341-t3620+t3622+t3634-t3638+t4076+t4077).*7.26735e-3;
et257 = t4785+t5058+t2307.*(t642+t643-t667+t674+t1587+t1606+t1608+t1609+t2295+t2671+t2683+t2684-t2695+t3272+t3290-t3296+t3576+t3582+t3588-t3593+t4015+t4016)+t2297.*(t2292+t3283+t3505.*1.838876e-2-t3570+t3571+t3590+t22.*(t1861-t3214).*3.131399999999998e-4+t22.*t23.*(t1861-t3214).*9.99471e-3);
t7393 = et256.*et257;
et258 = t2363.*(t2368+t3330+t3563.*1.838876e-2-t3618+t3619+t27.*(t1896-t3232).*1.247162e-2+t33.*(t1896-t3232).*3.131399999999998e-4+t33.*t34.*(t1896-t3232).*9.99471e-3);
et259 = 7.26735e-3;
t7406 = (t4758.*(t1861-t3214)+t2297.*(t642+t643-t667+t674+t1587+t1606+t1608+t1609+t2295+t2671+t2683+t2684-t2695+t3272+t3290-t3296+t3576+t3582+t3588-t3593+t4015+t4016)).*(t4872+t5144+et258.*et259+t2388.*(t684+t685-t710+t724+t1686-t1690+t1700+t1701+t2371+t2698+t2707-t2716+t2719+t3319-t3327-t3341-t3620+t3622+t3634-t3638+t4076+t4077).*7.26735e-3);
t7415 = t3139+t3140+t3326+t3335+t3444+t3456+t4591+t4593+t4594+t4597+t4884+t4885+t4890+t4896+t5121+t5126+t5128+t5131;
et260 = t5031-t7091+t4795.*(t1005+t26.*(t1941-t3308+t39.*t1022.*(t855-t878).*2.196325630278387e-1)).*7.26735e-3;
et261 = t2419.*(t684+t685-t710+t724+t1686-t1690+t1700+t1701+t2371+t2698+t2707-t2716+t2719+t3319-t3327-t3341-t3620+t3622+t3634-t3638+t4076+t4077).*7.26735e-3;
t7478 = -(et260+et261).*(t2674-t2676+t3022-t3027).*(t1488+t1874+t2519+t2740+t2747+t3096+t3097);
et262 = t5031-t7091+t4795.*(t1005+t26.*(t1941-t3308+t39.*t1022.*(t855-t878).*2.196325630278387e-1)).*7.26735e-3;
et263 = t2419.*(t684+t685-t710+t724+t1686-t1690+t1700+t1701+t2371+t2698+t2707-t2716+t2719+t3319-t3327-t3341-t3620+t3622+t3634-t3638+t4076+t4077).*7.26735e-3;
t7479 = (et262+et263).*(t2674-t2676+t3022-t3027).*(t1488+t1874+t2519+t2740+t2747+t3096+t3097);
t7552 = -t3057.*(-t5152+t5230+t5241+t5276-t5277-t5281+t5286+(t4865.*(t1861-t3214))./1.0e+8+(t3901.*(t951+t16.*(-t1881+t3121+t3269)))./1.0e+8+(t4080.*(t2694-t2701+t3036-t3043))./1.0e+8+t4777.*(t2694-t2701+t3036-t3043).*4.0e-8+t4780.*(t2694-t2701+t3036-t3043).*2.4e-7);
t7553 = t3057.*(-t5152+t5230+t5241+t5276-t5277-t5281+t5286+(t4865.*(t1861-t3214))./1.0e+8+(t3901.*(t951+t16.*(-t1881+t3121+t3269)))./1.0e+8+(t4080.*(t2694-t2701+t3036-t3043))./1.0e+8+t4777.*(t2694-t2701+t3036-t3043).*4.0e-8+t4780.*(t2694-t2701+t3036-t3043).*2.4e-7);
t7566 = (t3235-t3535).*(-t5152+t5230+t5241+t5276-t5277-t5281+t5286+(t4865.*(t1861-t3214))./1.0e+8+(t3901.*(t951+t16.*(-t1881+t3121+t3269)))./1.0e+8+(t4080.*(t2694-t2701+t3036-t3043))./1.0e+8+t4777.*(t2694-t2701+t3036-t3043).*4.0e-8+t4780.*(t2694-t2701+t3036-t3043).*2.4e-7);
t7567 = -t3992.*(-t5152+t5230+t5241+t5276-t5277-t5281+t5286+(t4865.*(t1861-t3214))./1.0e+8+(t3901.*(t951+t16.*(-t1881+t3121+t3269)))./1.0e+8+(t4080.*(t2694-t2701+t3036-t3043))./1.0e+8+t4777.*(t2694-t2701+t3036-t3043).*4.0e-8+t4780.*(t2694-t2701+t3036-t3043).*2.4e-7);
et264 = t5031-t7091+t4795.*(t1005+t26.*(t1941-t3308+t39.*t1022.*(t855-t878).*2.196325630278387e-1)).*7.26735e-3;
et265 = t2419.*(t684+t685-t710+t724+t1686-t1690+t1700+t1701+t2371+t2698+t2707-t2716+t2719+t3319-t3327-t3341-t3620+t3622+t3634-t3638+t4076+t4077).*7.26735e-3;
t7606 = (et264+et265).*(t4758.*(t1861-t3214)+t2297.*(t642+t643-t667+t674+t1587+t1606+t1608+t1609+t2295+t2671+t2683+t2684-t2695+t3272+t3290-t3296+t3576+t3582+t3588-t3593+t4015+t4016));
t7661 = t5054+t5667+t5691+t6057+t6987+t6990;
t7724 = t5371+t5807+t5828+t6151+t7027+t7044;
t7730 = t3210.*t7723;
t7733 = t3877.*t7723;
t7791 = t5600+t6060+t6087+t6575+t7228+t7229;
t4042 = -t4034;
t4043 = -t4035;
t4044 = -t4036;
t4096 = -t4089;
t4097 = -t4090;
t4098 = -t4091;
t4153 = -t4147;
t4637 = -t4636;
t4639 = -t4638;
t4802 = t3230.*t4494.*9.3e-7;
t4803 = t3230.*t4494.*1.02e-6;
t4806 = t3230.*t4494.*9.0e-8;
t4908 = -t4907;
t4910 = -t4909;
t4933 = t3528.*t4494.*9.3e-7;
t4934 = t3528.*t4494.*1.02e-6;
t4935 = t3531.*t4494.*9.3e-7;
t4936 = t3528.*t4494.*9.0e-8;
t4940 = t3531.*t4494.*9.0e-8;
t4945 = t27.*t4938;
t4948 = t27.*t4943;
t4980 = t3736.*t4541;
t5006 = t3844.*t4541;
t5078 = t3901.*t4494.*9.3e-7;
t5079 = t3901.*t4494.*1.02e-6;
t5080 = t3904.*t4494.*9.3e-7;
t5081 = t3901.*t4494.*9.0e-8;
t5084 = t3904.*t4494.*9.0e-8;
t5101 = t3943.*t4541;
t5132 = t3992.*t4494.*9.3e-7;
t5133 = t3992.*t4494.*1.02e-6;
t5134 = t3992.*t4494.*9.0e-8;
t5136 = t3996.*t4494.*9.3e-7;
t5140 = t3996.*t4494.*9.0e-8;
t5170 = t4113.*t4494.*9.3e-7;
t5171 = t4113.*t4494.*9.0e-8;
t5181 = t4122.*t4541;
t5182 = -t4541.*(-t2804+t2838+t3109+t23.*(t1456-t2355).*9.3e-7);
t5183 = -t4541.*(t2813-t2835+t18.*(t1456-t2355).*1.02e-6+t23.*(t1456-t2355).*9.0e-8);
t5188 = -t5185;
t5310 = -t5309;
t5312 = -t5311;
t5327 = -t5326;
t5372 = t2363.*t5329;
t5421 = t4494.*t4814.*9.3e-7;
t5422 = t4494.*t4814.*9.0e-8;
t5436 = t3057.*t5352;
t5460 = t4494.*t4860.*9.3e-7;
t5463 = t4494.*t4860.*9.0e-8;
t5495 = t2363.*t5430;
t5501 = -t5329.*(t1896-t3232);
t5502 = t3528.*t5329;
t5508 = t4706+t4715;
t5519 = t4719+t4763;
t5527 = t3057.*t5479;
t5586 = -t5585;
t5611 = -t5430.*(t1896-t3232);
t5612 = t3528.*t5430;
t5613 = t5430.*(t1896-t3232);
t5647 = t50.*t189.*t5610.*9.543032792050485e-17;
t5650 = -t5648;
t5652 = -t5352.*(t3235-t3535);
t5654 = t3992.*t5352;
t5657 = -t5655;
t5716 = -t5715;
t5743 = -t5479.*(t3235-t3535);
t5745 = t3992.*t5479;
t5746 = t5479.*(t3235-t3535);
t5763 = -t5762;
t5781 = -t5780;
t5797 = t67+t68+t89+t92+t2673+t2685+t2687+t2692+t3225+t3518+t3585+t3600+t4035+t4036;
t5810 = t3732.*t3901.*t5437.*1.08769e-2;
t5819 = t3484.*t5756;
t5822 = t3784.*t3901.*t5437.*1.08769e-2;
t5837 = -t5836;
t5844 = -t5842;
t5847 = -t5437.*(t3410-t3708+t3714+t26.*t50.*t202.*(t46-t47).*8.687615694748404e-39);
t5848 = t5437.*(t3410-t3708+t3714+t26.*t50.*t202.*(t46-t47).*8.687615694748404e-39);
t5849 = t358+t359+t378+t382+t2945+t2950+t2955+t2957+t3354+t3663+t3712+t3718+t4145+t4148;
t5872 = -t5756.*(-t1901+t3122+t3270);
t5874 = -t5873;
t5875 = t5756.*(-t1901+t3122+t3270);
t5885 = t4175.*t5437.*(t2694-t2701+t3036-t3043).*(-1.08769e-2);
t5886 = t4175.*t5437.*(t2694-t2701+t3036-t3043).*1.08769e-2;
t5892 = t3689.*t3877.*t5590;
t5919 = t3782.*t3877.*t5590;
t5925 = -t5756.*(t951+t16.*(-t1881+t3121+t3269));
t5928 = -t5927;
t5936 = -t5935;
t5938 = -t5937;
t5939 = t4975.*t5437;
t5946 = -t5945;
t5948 = t4651.*t5590;
t5962 = t3877.*t3891.*t5590;
t5973 = -t4134.*t5590.*(t2674-t2676+t3022-t3027);
t5982 = -t5980;
t5983 = t4678+t5641;
t5985 = t4676+t5644;
t5987 = -t5986;
t5989 = -t5988;
t5990 = t4897.*t5590;
t6005 = t4685+t5686;
t6007 = t4770+t5680;
t6022 = t2363.*t6001;
t6023 = t2388.*t6001;
t6024 = t2419.*t6001;
t6036 = t3254+t3263+t4374+t4377+t4382+t4398;
t6037 = t3260+t3261+t4376+t4379+t4388+t4397;
t6044 = -t6042;
t6048 = t3057.*t6008;
et266 = -t2306-t2317+t3144+t3147+t35.*t941.*t948.*(t850-t874).*3.775747223193135e-1;
et267 = t36.*t941.*t948.*(t850-t874).*2.244797987218524e-1;
t6052 = -t5756.*(et266+et267);
et268 = -t2306-t2317+t3144+t3147+t35.*t941.*t948.*(t850-t874).*3.775747223193135e-1;
et269 = t36.*t941.*t948.*(t850-t874).*2.244797987218524e-1;
t6053 = t5756.*(et268+et269);
t6055 = t33.*t2363.*t6035;
t6068 = t3524.*t6001;
t6069 = -t6001.*(t1896-t3232);
t6070 = t3528.*t6001;
t6071 = t3531.*t6001;
t6073 = t2998.*t6035;
t6077 = t3057.*t6035;
t6078 = -t6035.*(t1477-t2502);
t6081 = t6035.*(t1477-t2502);
t6098 = t3918.*t5798.*(t2694-t2701+t3036-t3043).*(-7.26735e-3);
t6099 = t3918.*t5799.*(t2694-t2701+t3036-t3043).*(-7.26735e-3);
t6102 = -t6100;
t6105 = -t6104;
t6107 = t5223.*t5590;
t6113 = t3984.*t5798.*(t2694-t2701+t3036-t3043).*(-7.26735e-3);
t6114 = t3984.*t5798.*(t2694-t2701+t3036-t3043).*7.26735e-3;
t6115 = t3984.*t5799.*(t2694-t2701+t3036-t3043).*(-7.26735e-3);
t6116 = t3984.*t5799.*(t2694-t2701+t3036-t3043).*7.26735e-3;
t6120 = -t6119;
t6121 = t3386.*t6039;
t6123 = t2363.*t6088;
t6124 = t2388.*t6088;
t6126 = t2419.*t6088;
t6129 = t4149.*t5798.*(t2694-t2701+t3036-t3043).*(-7.26735e-3);
t6130 = t4149.*t5799.*(t2694-t2701+t3036-t3043).*(-7.26735e-3);
t6139 = -t6138;
t6141 = -t6140;
et270 = -t2306-t2317+t3144+t3147+t35.*t941.*t948.*(t850-t874).*3.775747223193135e-1;
et271 = t36.*t941.*t948.*(t850-t874).*2.244797987218524e-1;
t6142 = -t4134.*t5590.*(et270+et271);
t6145 = -t33.*t6035.*(t1896-t3232);
t6146 = t33.*t3528.*t6035;
t6148 = t33.*t6035.*(t1896-t3232);
t6152 = -t3484.*(t4311-t5186+t4541.*(-t2804+t2838+t3109+t23.*(t1456-t2355).*9.3e-7));
t6154 = -t17.*t3483.*(t4311-t5186+t4541.*(-t2804+t2838+t3109+t23.*(t1456-t2355).*9.3e-7));
t6155 = t3484.*(t4311-t5186+t4541.*(-t2804+t2838+t3109+t23.*(t1456-t2355).*9.3e-7));
t6157 = t5757.*(t2694-t2701+t3036-t3043).*(t1513+t1879+t2598+t2820+t2834+t3117+t3118).*7.26735e-3;
t6164 = t5437.*t5485;
t6170 = t656+t659+t660+t681+t1577+t1578+t1586+t1600+t2303+t2339+t2673+t2685+t2686+t2687+t3030+t3225+t3292+t3305+t3518+t3585+t3600+t4035+t4036;
t6171 = t3419+t3421+t4507+t4517+t4523+t4540;
t6172 = t3415+t3433+t4508+t4511+t4529+t4534;
t6174 = t3432+t3437+t4515+t4536+t4561+t4565;
t6178 = t5783.*(t2674-t2676+t3022-t3027).*(t1488+t1874+t2519+t2740+t2747+t3096+t3097);
t6179 = t4113.*t6001;
t6180 = -t6001.*(t1005+t26.*(t1941-t3308+t39.*t1022.*(t855-t878).*2.196325630278387e-1));
t6182 = t188.*t6165.*8.595599785252598e-1;
t6190 = -t6008.*(t3235-t3535);
t6191 = t3992.*t6008;
t6195 = t50.*t189.*t6165.*9.543032792050485e-17;
t6203 = t694+t736+t740+t741+t1615+t1616+t1660+t1717+t2403+t2493+t2704+t2708+t2709+t2720+t3045+t3245+t3337+t3353+t3569+t3631+t3641+t4090+t4091;
t6212 = t3524.*t6088;
t6213 = -t6088.*(t1896-t3232);
t6214 = t3528.*t6088;
t6215 = t3531.*t6088;
t6218 = -t3892.*t5884.*(t2674-t2676+t3022-t3027);
t6222 = -t3892.*t5888.*(t2674-t2676+t3022-t3027);
t6225 = t201.*t6201.*6.246723209935546e-3;
t6234 = -t3941.*t5884.*(t2674-t2676+t3022-t3027);
t6235 = t3941.*t5884.*(t2674-t2676+t3022-t3027);
t6237 = -t3941.*t5888.*(t2674-t2676+t3022-t3027);
t6239 = t3941.*t5888.*(t2674-t2676+t3022-t3027);
t6241 = (-t1901+t3122+t3270).*(t4311-t5186+t4541.*(-t2804+t2838+t3109+t23.*(t1456-t2355).*9.3e-7));
t6243 = t50.*t202.*t6201.*6.935255936130809e-19;
t6246 = t5437.*t5539;
t6250 = t3901.*t5798.*(t1513+t1879+t2598+t2820+t2834+t3117+t3118).*(-7.26735e-3);
t6252 = -t6248;
t6258 = t3985.*t6035;
t6260 = -t6035.*(t3235-t3535);
t6262 = t3992.*t6035;
t6264 = t3996.*t6035;
t6268 = -t6173.*(t1477-t2502);
t6269 = -t4108.*t5884.*(t2674-t2676+t3022-t3027);
t6270 = -t3967.*(t4311-t5186+t4541.*(-t2804+t2838+t3109+t23.*(t1456-t2355).*9.3e-7));
t6272 = t6173.*(t1477-t2502);
t6273 = t4108.*t5884.*(t2674-t2676+t3022-t3027);
t6274 = t3057.*t6175;
t6275 = -t6271;
t6276 = -t4108.*t5888.*(t2674-t2676+t3022-t3027);
t6277 = t4108.*t5888.*(t2674-t2676+t3022-t3027);
t6284 = t5412.*t5590;
t6289 = t3057.*t6189;
t6294 = (t951+t16.*(-t1881+t3121+t3269)).*(t4311-t5186+t4541.*(-t2804+t2838+t3109+t23.*(t1456-t2355).*9.3e-7));
t6296 = t5429.*t5590;
t6299 = -t3385.*(t3417-t3421-t4507+t4513+t4519-t4540);
t6309 = t4721+t4725+t4733+t4773;
t6310 = t4718+t4729+t4755+t4761;
t6312 = t4720+t4737+t4744+t4771;
t6328 = -t4298.*t5884.*(t2674-t2676+t3022-t3027);
t6330 = -t6327;
t6332 = t3860+t4623+t4625+t4627+t4677;
t6333 = -t4298.*t5888.*(t2674-t2676+t3022-t3027);
t6345 = t4113.*t6088;
t6346 = -t6088.*(t1005+t26.*(t1941-t3308+t39.*t1022.*(t855-t878).*2.196325630278387e-1));
t6350 = -t3877.*t5884.*(t1488+t1874+t2519+t2740+t2747+t3096+t3097);
t6351 = t3877.*t5884.*(t1488+t1874+t2519+t2740+t2747+t3096+t3097);
t6363 = -t6359;
t6368 = t4510.*t6039;
t6370 = t4541.*t6038;
t6371 = -t6039.*(t3544-t4013);
et272 = t3563.*1.33637554986e-4+t3693-t3694+t33.*(t1896-t3232).*4.36041e-5;
et273 = t33.*t34.*(t1896-t3232).*7.26350557185e-5;
t6372 = -t5798.*(et272+et273);
et274 = t3563.*1.33637554986e-4+t3693-t3694+t33.*(t1896-t3232).*4.36041e-5;
et275 = t33.*t34.*(t1896-t3232).*7.26350557185e-5;
t6373 = t5798.*(et274+et275);
et276 = t3563.*1.33637554986e-4+t3693-t3694+t33.*(t1896-t3232).*4.36041e-5;
et277 = t33.*t34.*(t1896-t3232).*7.26350557185e-5;
t6374 = -t5799.*(et276+et277);
t6381 = -t5798.*(t3349-t3649+t28.*(t3235-t3535).*1.33637554986e-4+t34.*(t3235-t3535).*7.26350557185e-5);
t6382 = t5798.*(t3349-t3649+t28.*(t3235-t3535).*1.33637554986e-4+t34.*(t3235-t3535).*7.26350557185e-5);
t6383 = -t5799.*(t3349-t3649+t28.*(t3235-t3535).*1.33637554986e-4+t34.*(t3235-t3535).*7.26350557185e-5);
t6384 = t5799.*(t3349-t3649+t28.*(t3235-t3535).*1.33637554986e-4+t34.*(t3235-t3535).*7.26350557185e-5);
t6390 = -t6389;
t6391 = t3386.*t6315;
t6393 = t3985.*t6173;
t6398 = -t6175.*(t3235-t3535);
t6399 = t3996.*t6173;
t6401 = t3992.*t6175;
t6402 = -t6189.*(t3235-t3535);
t6403 = t3992.*t6189;
t6404 = t6189.*(t3235-t3535);
t6410 = -t6408;
t6416 = -t5798.*(t3547.*1.33637554986e-4+t4119-t4120+t34.*(t1896-t3232).*7.26350557185e-5);
t6417 = t5798.*(t3547.*1.33637554986e-4+t4119-t4120+t34.*(t1896-t3232).*7.26350557185e-5);
t6418 = -t5799.*(t3547.*1.33637554986e-4+t4119-t4120+t34.*(t1896-t3232).*7.26350557185e-5);
t6419 = t5799.*(t3547.*1.33637554986e-4+t4119-t4120+t34.*(t1896-t3232).*7.26350557185e-5);
t6422 = -t5884.*(t3505.*1.838876e-2-t3570+t3571+t22.*(t1861-t3214).*(3.0./5.0e+2)+t22.*t23.*(t1861-t3214).*9.99471e-3);
t6423 = t5884.*(t3505.*1.838876e-2-t3570+t3571+t22.*(t1861-t3214).*(3.0./5.0e+2)+t22.*t23.*(t1861-t3214).*9.99471e-3);
t6424 = -t5888.*(t3505.*1.838876e-2-t3570+t3571+t22.*(t1861-t3214).*(3.0./5.0e+2)+t22.*t23.*(t1861-t3214).*9.99471e-3);
t6433 = (t17.*((t237.*(t42-t43))./9.007199254740992e+15+t21.*(-t1881+t3121+t3269))+t22.*(-t1901+t3122+t3270)).*(t4311-t5186+t4541.*(-t2804+t2838+t3109+t23.*(t1456-t2355).*9.3e-7));
t6434 = t4817.*t6035;
t6435 = t4824.*t6035;
t6439 = t5590.*t5723;
et278 = -t2306-t2317+t3144+t3147+t35.*t941.*t948.*(t850-t874).*3.775747223193135e-1;
et279 = t36.*t941.*t948.*(t850-t874).*2.244797987218524e-1;
t6445 = (et278+et279).*(t4311-t5186+t4541.*(-t2804+t2838+t3109+t23.*(t1456-t2355).*9.3e-7));
t6446 = t5258.*t5884;
t6447 = t5258.*t5888;
t6465 = -t5884.*(-t4007+t4011+t18.*(t1861-t3214).*1.838876e-2+t23.*(t1861-t3214).*9.99471e-3);
t6466 = t5884.*(-t4007+t4011+t18.*(t1861-t3214).*1.838876e-2+t23.*(t1861-t3214).*9.99471e-3);
t6467 = -t5888.*(-t4007+t4011+t18.*(t1861-t3214).*1.838876e-2+t23.*(t1861-t3214).*9.99471e-3);
t6468 = t5888.*(-t4007+t4011+t18.*(t1861-t3214).*1.838876e-2+t23.*(t1861-t3214).*9.99471e-3);
t6471 = -t4514.*(t3417-t3421-t4507+t4513+t4519-t4540);
t6474 = -t4541.*(t3417-t3421-t4507+t4513+t4519-t4540);
t6482 = -t4541.*(t4555+t4571-t18.*t2363.*t3047.*9.0e-8-t23.*t2363.*t3047.*9.3e-7+t18.*t3946.*(t1896-t3232).*9.0e-8+t23.*t3946.*(t1896-t3232).*9.3e-7);
t6487 = t27.*t2363.*t6473;
t6491 = t5437.*t5840;
t6494 = t3003.*t6473;
t6495 = -t4822.*t5884.*(t1488+t1874+t2519+t2740+t2747+t3096+t3097);
t6496 = -t4822.*t5888.*(t1488+t1874+t2519+t2740+t2747+t3096+t3097);
t6503 = t3057.*t6473;
t6504 = -t6473.*(t1477-t2502);
t6505 = t6473.*(t1477-t2502);
t6517 = t3678+t3679+t4818+t4825+t4854+t4855;
t6522 = t4510.*t6315;
t6525 = -t6523;
t6526 = t4541.*t6313;
t6527 = -t6315.*(t3544-t4013);
t6531 = -t27.*t6473.*(t1896-t3232);
t6532 = t27.*t3528.*t6473;
t6559 = t5737.*t5798;
t6560 = t5737.*t5799;
t6571 = t5437.*t5992;
t6577 = t3057.*t6539;
t6578 = t3985.*t6473;
t6579 = -t6473.*(t3235-t3535);
t6580 = t3992.*t6473;
t6581 = t6473.*(t3235-t3535);
t6582 = t3996.*t6473;
t6592 = -t5590.*(t1554+t2361+t2362+t2367+t2414+t3928+t3934+t4160+t4163+t17.*(-t1901+t3122+t3270).*5.68686e-3);
t6594 = t3129+t3428+t3450+t4235+t4237+t4525+t4535+t4559+t4575;
t6601 = -t6600;
t6605 = -t6604;
t6607 = t5590.*t5951;
t6608 = t5590.*t5954;
t6613 = t5783.*t5798;
t6614 = t5783.*t5799;
t6630 = t5061+t6279;
t6645 = -t5798.*(t4610+t2363.*(t3547.*1.838876e-2+t4071-t4072+t34.*(t1896-t3232).*9.99471e-3).*7.26735e-3);
t6649 = -t5799.*(t4610+t2363.*(t3547.*1.838876e-2+t4071-t4072+t34.*(t1896-t3232).*9.99471e-3).*7.26735e-3);
t6688 = t5757.*t5884;
t6690 = t5757.*t5888;
t6693 = t5145+t6307;
t6707 = -t6539.*(t3235-t3535);
t6708 = t3992.*t6539;
t6719 = -t5884.*(t5359+t4108.*(t1861-t3214));
t6720 = t5884.*(t5359+t4108.*(t1861-t3214));
t6721 = -t5888.*(t5359+t4108.*(t1861-t3214));
t6722 = t5888.*(t5359+t4108.*(t1861-t3214));
t6751 = t4437+t4438+t4721+t4727+t4753+t4773;
t6754 = -t6753;
t6755 = t4814.*t6473;
t6756 = -t6473.*(t4127+t33.*(t1959-t3306+t38.*t1022.*(t855-t878).*2.196325630278387e-1));
t6765 = t5437.*t6183;
t6772 = t3209.*t6706;
t6788 = -t6706.*(t1861-t3214);
t6795 = -t6794;
t6809 = t188.*t6805.*8.595599785252598e-1;
t6816 = -t6706.*(t2674-t2676+t3022-t3027);
t6833 = t3946.*t6706;
t6854 = t3209.*t6804;
t6855 = t4168+t4581+t4600+t4659+t5190+t5206;
t6863 = t3209.*t6807;
t6864 = t5884.*t5975;
t6866 = t5888.*t5975;
t6883 = -t6804.*(t1861-t3214);
t6884 = t6804.*(t1861-t3214);
t6889 = -t6887;
t6900 = -t6807.*(t1861-t3214);
t6910 = -t6909;
t6932 = -t6804.*(t2674-t2676+t3022-t3027);
t6933 = t6804.*(t2674-t2676+t3022-t3027);
t6943 = t3946.*t6804;
t6944 = -t6807.*(t2674-t2676+t3022-t3027);
t6956 = t3946.*t6807;
t6973 = -t6972;
t7018 = -t6986.*(t1477-t2502);
t7060 = -t7057;
t7061 = -t7058;
t7087 = t3057.*t7046;
t7093 = -t7092;
t7096 = t3985.*t6986;
t7098 = t3996.*t6986;
t7101 = -t7046.*(t3235-t3535);
t7102 = t3992.*t7046;
t7103 = t7046.*(t3235-t3535);
t7118 = t5798.*t6565;
t7120 = t5799.*t6565;
t7127 = t5884.*(-t2308+t2378+t2510-t2530-t2975+t2979+t3893+t4106+t4152+t4155+t4805+t4809);
t7128 = t5888.*(-t2308+t2378+t2510-t2530-t2975+t2979+t3893+t4106+t4152+t4155+t4805+t4809);
t7141 = -t5783.*(t4758.*(t1861-t3214)+t2297.*(t642+t643-t667+t674+t1587+t1606+t1608+t1609+t2295+t2671+t2683+t2684-t2695+t3272+t3290-t3296+t3576+t3582+t3588-t3593+t4015+t4016));
t7147 = -t5757.*(t4795.*(t1896-t3232).*7.26735e-3+t2363.*(t684+t685-t710+t724+t1686-t1690+t1700+t1701+t2371+t2698+t2707-t2716+t2719+t3319-t3327-t3341-t3620+t3622+t3634-t3638+t4076+t4077).*7.26735e-3);
t7148 = t5757.*(t4795.*(t1896-t3232).*7.26735e-3+t2363.*(t684+t685-t710+t724+t1686-t1690+t1700+t1701+t2371+t2698+t2707-t2716+t2719+t3319-t3327-t3341-t3620+t3622+t3634-t3638+t4076+t4077).*7.26735e-3);
t7152 = -t7151;
t7177 = t2363.*t7174;
t7182 = t4787+t5064+t5661+t6280;
t7187 = -t7174.*(t1896-t3232);
t7188 = t3528.*t7174;
t7189 = t4873+t5146+t5699+t6308;
t7191 = t4296+t5002+t5099+t5100+t5603+t5605;
t7201 = -t7200;
t7213 = t3134+t3135+t3164+t3172+t3440+t3449+t4233+t4234+t4238+t4239+t4257+t4263+t4264+t4268+t4520+t4531+t4568+t4580;
t7238 = -t7236;
t7240 = t50.*t189.*t7233.*9.543032792050485e-17;
t7264 = -t7263;
t7270 = -t7269.*(t1477-t2502);
t7271 = t7269.*(t1477-t2502);
t7277 = t3209.*t7272;
t7278 = t3210.*t7273;
t7281 = t3985.*t7269;
t7282 = t3996.*t7269;
t7295 = -t7272.*(t2674-t2676+t3022-t3027);
t7296 = t7272.*(t2674-t2676+t3022-t3027);
t7297 = t3877.*t7273;
et280 = t2363.*(t2368+t3330+t3563.*1.838876e-2-t3618+t3619+t27.*(t1896-t3232).*1.247162e-2+t33.*(t1896-t3232).*3.131399999999998e-4+t33.*t34.*(t1896-t3232).*9.99471e-3);
et281 = 7.26735e-3;
t7302 = -t5798.*(t4872+t5144+et280.*et281+t2388.*(t684+t685-t710+t724+t1686-t1690+t1700+t1701+t2371+t2698+t2707-t2716+t2719+t3319-t3327-t3341-t3620+t3622+t3634-t3638+t4076+t4077).*7.26735e-3);
et282 = t2363.*(t2368+t3330+t3563.*1.838876e-2-t3618+t3619+t27.*(t1896-t3232).*1.247162e-2+t33.*(t1896-t3232).*3.131399999999998e-4+t33.*t34.*(t1896-t3232).*9.99471e-3);
et283 = 7.26735e-3;
t7303 = t5798.*(t4872+t5144+et282.*et283+t2388.*(t684+t685-t710+t724+t1686-t1690+t1700+t1701+t2371+t2698+t2707-t2716+t2719+t3319-t3327-t3341-t3620+t3622+t3634-t3638+t4076+t4077).*7.26735e-3);
et284 = t2363.*(t2368+t3330+t3563.*1.838876e-2-t3618+t3619+t27.*(t1896-t3232).*1.247162e-2+t33.*(t1896-t3232).*3.131399999999998e-4+t33.*t34.*(t1896-t3232).*9.99471e-3);
et285 = 7.26735e-3;
t7304 = -t5799.*(t4872+t5144+et284.*et285+t2388.*(t684+t685-t710+t724+t1686-t1690+t1700+t1701+t2371+t2698+t2707-t2716+t2719+t3319-t3327-t3341-t3620+t3622+t3634-t3638+t4076+t4077).*7.26735e-3);
et286 = t2363.*(t2368+t3330+t3563.*1.838876e-2-t3618+t3619+t27.*(t1896-t3232).*1.247162e-2+t33.*(t1896-t3232).*3.131399999999998e-4+t33.*t34.*(t1896-t3232).*9.99471e-3);
et287 = 7.26735e-3;
t7305 = t5799.*(t4872+t5144+et286.*et287+t2388.*(t684+t685-t710+t724+t1686-t1690+t1700+t1701+t2371+t2698+t2707-t2716+t2719+t3319-t3327-t3341-t3620+t3622+t3634-t3638+t4076+t4077).*7.26735e-3);
t7308 = -t5884.*(t4785+t5058+t2307.*(t642+t643-t667+t674+t1587+t1606+t1608+t1609+t2295+t2671+t2683+t2684-t2695+t3272+t3290-t3296+t3576+t3582+t3588-t3593+t4015+t4016)+t2297.*(t2292+t3283+t3505.*1.838876e-2-t3570+t3571+t3590+t22.*(t1861-t3214).*3.131399999999998e-4+t22.*t23.*(t1861-t3214).*9.99471e-3));
t7309 = -t5888.*(t4785+t5058+t2307.*(t642+t643-t667+t674+t1587+t1606+t1608+t1609+t2295+t2671+t2683+t2684-t2695+t3272+t3290-t3296+t3576+t3582+t3588-t3593+t4015+t4016)+t2297.*(t2292+t3283+t3505.*1.838876e-2-t3570+t3571+t3590+t22.*(t1861-t3214).*3.131399999999998e-4+t22.*t23.*(t1861-t3214).*9.99471e-3));
t7327 = t5228+t5236+t5239+t5242+t5273+t5283+t5284+t5285;
t7329 = -t7328;
t7358 = t2993+t3055+t3186+t3193+t3197+t3198+t4410+t4412+t4439+t4440+t4732+t4738+t4757+t4775+t5023+t5025+t5027+t5030;
t7371 = t4996+t5255+t6285+t7049;
t7394 = -t7393;
t7397 = t5032+t5302+t6311+t7091;
t7407 = -t7406;
t7427 = t3057.*t7415;
t7452 = -t7415.*(t3235-t3535);
t7453 = t3992.*t7415;
t7454 = t7415.*(t3235-t3535);
t7459 = -t3481.*(t6887+t3985.*(t4737+t4744+t4751+t3942.*(t2694-t2701+t3036-t3043).*5.7e-7)+t6088.*(t1896-t3232));
et288 = t5031-t7091+t4795.*(t1005+t26.*(t1941-t3308+t39.*t1022.*(t855-t878).*2.196325630278387e-1)).*7.26735e-3;
et289 = t2419.*(t684+t685-t710+t724+t1686-t1690+t1700+t1701+t2371+t2698+t2707-t2716+t2719+t3319-t3327-t3341-t3620+t3622+t3634-t3638+t4076+t4077).*7.26735e-3;
t7530 = -t5798.*(et288+et289);
et290 = t5031-t7091+t4795.*(t1005+t26.*(t1941-t3308+t39.*t1022.*(t855-t878).*2.196325630278387e-1)).*7.26735e-3;
et291 = t2419.*(t684+t685-t710+t724+t1686-t1690+t1700+t1701+t2371+t2698+t2707-t2716+t2719+t3319-t3327-t3341-t3620+t3622+t3634-t3638+t4076+t4077).*7.26735e-3;
t7534 = -t5799.*(et290+et291);
tau_c = ft_14({t1005,t1022,t1089,t1104,t1105,t1108,t1115,t1121,t1158,t1159,t1196,t1205,t1210,t1212,t1217,t1218,t123,t1237,t1238,t1288,t1289,t1302,t1303,t1319,t1320,t1336,t1348,t1350,t1351,t1360,t1369,t1378,t1396,t14,t140,t1425,t1435,t1456,t1477,t1488,t15,t1513,t1539,t1554,t1577,t1578,t1586,t1587,t16,t1600,t1604,t1605,t1606,t1607,t1608,t1609,t1628,t1629,t1637,t1640,t1641,t1659,t1661,t1666,t1667,t1683,t1686,t1690,t1692,t17,t1700,t1701,t1705,t1712,t1741,t1742,t1750,t1754,t1758,t1759,t1775,t1776,t18,t1861,t1874,t1879,t188,t1881,t189,t1896,t19,t1901,t1941,t1959,t1973,t1993,t1994,t2,t20,t201,t202,t2023,t2053,t2060,t2089,t2090,t2098,t2099,t21,t2117,t2120,t2122,t2123,t2139,t2140,t2147,t2152,t2154,t2155,t2159,t2165,t2174,t2183,t2187,t2193,t2194,t2195,t2199,t22,t2203,t2215,t2219,t2222,t2223,t2239,t2240,t2256,t2257,t2292,t2295,t2297,t23,t2302,t2303,t2306,t2307,t2308,t2317,t2337,t2338,t2339,t2355,t236,t2361,t2362,t2363,t2367,t2368,t237,t2371,t2378,t238,t2388,t24,t2401,t241,t2414,t2419,t244,t25,t2502,t2510,t2519,t2527,t2530,t2555,t2556,t2572,t2583,t2598,t26,t2605,t2606,t2612,t2613,t2618,t2619,t262,t264,t2651,t2652,t2670,t2671,t2674,t2676,t2680,t2683,t2684,t2689,t2693,t2694,t2695,t2697,t2698,t27,t2700,t2701,t2707,t2712,t2715,t2716,t2719,t2721,t2740,t2747,t2754,t28,t2801,t2804,t2813,t2814,t2820,t2831,t2834,t2835,t2838,t2850,t2851,t2953,t2963,t2964,t2975,t2979,t2990,t2991,t2994,t3,t30,t3003,t3009,t3022,t3027,t3030,t3036,t3043,t3047,t3054,t3056,t3057,t3064,t3072,t3080,t3096,t3097,t31,t3109,t3117,t3118,t3121,t3122,t3128,t313,t3130,t3131,t3132,t314,t3141,t3142,t3144,t3147,t3156,t3157,t3170,t3189,t3190,t32,t3200,t3206,t3209,t321,t3210,t3214,t3228,t3229,t3230,t3231,t3232,t3235,t3250,t3269,t3270,t3272,t3276,t3283,t329,t3290,t3291,t3292,t3296,t33,t3305,t3306,t3307,t3308,t3313,t3318,t3319,t332,t3324,t3327,t3330,t3334,t3336,t3341,t3349,t335,t3357,t3359,t3360,t3376,t3385,t3386,t3395,t3399,t34,t3405,t3409,t3410,t3412,t3417,t3420,t3421,t3423,t3424,t3435,t3437,t3455,t346,t3465,t3468,t3470,t3473,t3475,t3477,t3479,t3480,t3481,t3483,t3484,t3493,t3498,t35,t350,t3505,t3522,t3524,t3526,t3527,t3528,t3530,t3532,t3533,t3535,t3539,t354,t3542,t3544,t3547,t3560,t3563,t3570,t3571,t3576,t3582,t3586,t3587,t3588,t3589,t3590,t3593,t3596,t36,t3603,t3616,t3617,t3618,t3619,t3620,t3621,t3622,t3628,t3632,t3633,t3634,t3635,t3637,t3638,t3639,t3643,t3649,t3657,t366,t3664,t3665,t3667,t3669,t3670,t3672,t3673,t3674,t3676,t3680,t3681,t3682,t3683,t3684,t3685,t3686,t3687,t3689,t3690,t3693,t3694,t3705,t3706,t3708,t3709,t3713,t3714,t3715,t3716,t3723,t3724,t3729,t3732,t3734,t3735,t3744,t3745,t3746,t3748,t3749,t3751,t3753,t3755,t3756,t3757,t3758,t3759,t3760,t3762,t3763,t3764,t3765,t3766,t3767,t3768,t3769,t3770,t3771,t3772,t3774,t3775,t3776,t3778,t3779,t3782,t3783,t3784,t3790,t3791,t3794,t3795,t3797,t3798,t3799,t38,t3801,t3803,t3804,t3806,t3811,t3814,t3815,t3816,t3817,t3819,t3821,t3822,t3826,t3827,t3828,t3833,t3834,t3847,t3849,t3850,t3861,t3862,t3863,t3865,t3866,t3869,t387,t3870,t3871,t3872,t3875,t3877,t3880,t3882,t3891,t3892,t3893,t3898,t39,t3901,t3904,t3910,t3918,t3922,t3928,t3934,t3940,t3941,t3942,t3946,t3951,t3957,t3959,t3967,t3972,t3974,t3984,t3985,t3992,t3996,t4,t4007,t4011,t4013,t4015,t4016,t4027,t4037,t4042,t4043,t4044,t4062,t4071,t4072,t4076,t4077,t4080,t4086,t4096,t4097,t4098,t410,t4106,t4108,t4109,t4113,t4119,t4120,t4125,t4127,t4133,t4134,t4146,t4149,t4152,t4153,t4154,t4155,t4160,t4163,t4173,t4175,t4196,t42,t4200,t4201,t4219,t4220,t4221,t4227,t4228,t4230,t4231,t4238,t4239,t4242,t4243,t4244,t4245,t4246,t4247,t4248,t4255,t4256,t4257,t4259,t4264,t4266,t4276,t4277,t4279,t4280,t4281,t4285,t4287,t4291,t4292,t4295,t4297,t4298,t43,t4304,t4308,t4310,t4311,t4313,t4316,t4320,t4321,t4322,t4323,t4324,t4356,t4362,t4363,t4400,t4405,t4406,t4409,t4413,t4421,t4428,t4429,t4432,t4436,t4437,t4438,t4444,t4447,t4458,t4491,t4496,t4499,t4500,t4504,t4507,t4510,t4513,t4514,t4519,t4520,t4531,t4540,t4541,t4543,t4552,t4554,t4555,t4556,t4560,t4571,t4572,t4576,t4579,t4582,t4588,t4589,t4595,t4599,t46,t4602,t4610,t4612,t4613,t4614,t4615,t4617,t4620,t4628,t4629,t4631,t4633,t4634,t4635,t4637,t4639,t4640,t4641,t4642,t4644,t4645,t4647,t4650,t4652,t4655,t4658,t4661,t4663,t4664,t4666,t4667,t4669,t4679,t4680,t4682,t4683,t4686,t4688,t4699,t47,t4702,t4703,t4704,t4705,t4737,t4741,t4742,t4744,t4751,t4752,t4758,t4767,t4772,t4777,t4780,t4785,t4786,t4788,t4789,t4790,t4791,t4792,t4793,t4794,t4795,t4796,t4798,t4799,t4800,t4801,t4802,t4803,t4805,t4806,t4807,t4808,t4809,t4812,t4814,t4816,t4817,t4819,t4822,t4823,t4824,t4826,t4829,t4833,t4835,t4836,t4840,t4842,t4843,t4845,t4847,t4848,t4849,t4850,t4851,t4852,t4853,t4856,t4857,t4858,t4859,t4860,t4865,t4868,t4869,t4870,t4871,t4872,t4874,t4875,t4882,t4883,t4898,t4899,t4900,t4902,t4904,t4905,t4906,t4908,t4910,t4911,t4913,t4915,t4917,t4918,t4919,t4920,t4921,t4922,t4924,t4925,t4926,t4927,t4929,t4930,t4931,t4932,t4933,t4934,t4935,t4936,t4938,t4940,t4941,t4942,t4943,t4945,t4946,t4947,t4948,t4950,t4952,t4953,t4954,t4956,t4958,t4959,t4960,t4961,t4962,t4963,t4965,t4970,t4972,t4974,t4975,t4976,t4977,t4980,t4981,t4982,t4983,t4984,t4985,t4986,t4987,t4992,t4994,t4995,t4998,t5,t50,t5000,t5005,t5006,t5007,t5008,t5013,t5014,t5031,t5033,t5034,t5035,t5036,t5038,t5039,t5040,t5041,t5042,t5047,t5048,t5049,t5051,t5052,t5055,t5056,t5057,t5058,t5059,t5062,t5063,t5066,t5067,t5068,t5069,t5070,t5071,t5073,t5074,t5075,t5076,t5077,t5078,t5079,t5080,t5081,t5083,t5084,t5085,t5086,t5087,t5088,t5089,t5092,t5101,t5102,t5103,t5104,t5105,t5106,t5108,t5109,t5111,t5112,t5113,t5114,t5116,t5117,t5119,t5132,t5133,t5134,t5135,t5136,t5137,t5138,t5139,t5140,t5141,t5142,t5143,t5144,t5147,t5148,t5149,t5150,t5151,t5152,t5153,t5155,t5156,t5157,t5158,t5161,t5162,t5164,t5166,t5170,t5171,t5172,t5173,t5181,t5182,t5183,t5184,t5185,t5186,t5187,t5188,t5189,t5191,t5192,t5195,t5196,t5198,t5201,t5202,t5203,t5204,t5207,t5209,t5210,t5220,t5223,t5224,t5225,t5226,t5227,t5230,t5231,t5233,t5234,t5235,t5238,t5240,t5241,t5243,t5244,t5245,t5246,t5247,t5248,t5250,t5252,t5254,t5257,t5258,t5262,t5273,t5276,t5277,t5278,t5280,t5281,t5282,t5285,t5286,t5287,t5288,t5289,t5291,t5293,t5295,t5301,t5304,t5306,t5307,t5308,t5310,t5312,t5314,t5316,t5317,t5320,t5321,t5322,t5327,t5328,t5329,t5330,t5331,t5332,t5335,t5337,t5338,t5339,t5340,t5342,t5344,t5345,t5346,t5347,t5348,t5349,t5350,t5356,t5357,t5358,t5359,t5361,t5362,t5365,t5367,t5372,t5377,t5379,t5380,t5381,t5383,t5384,t5385,t5386,t5387,t5388,t5389,t5390,t5391,t5392,t5393,t5395,t5396,t5397,t5399,t5400,t5402,t5403,t5405,t5407,t5411,t5412,t5413,t5414,t5416,t5418,t5419,t5420,t5421,t5422,t5423,t5424,t5426,t5427,t5428,t5429,t5432,t5433,t5434,t5435,t5436,t5437,t5438,t5440,t5441,t5443,t5444,t5445,t5446,t5447,t5448,t5449,t5450,t5451,t5452,t5453,t5454,t5455,t5456,t5457,t5458,t5459,t5460,t5461,t5462,t5463,t5464,t5465,t5466,t5468,t5480,t5481,t5482,t5483,t5484,t5486,t5487,t5488,t5489,t5490,t5491,t5492,t5493,t5494,t5495,t5496,t5498,t5499,t5500,t5501,t5502,t5503,t5504,t5505,t5506,t5507,t5509,t5512,t5513,t5514,t5515,t5516,t5517,t5518,t5520,t5521,t5522,t5523,t5524,t5525,t5526,t5527,t5528,t5530,t5531,t5532,t5533,t5534,t5535,t5536,t5537,t5538,t5539,t5541,t5542,t5543,t5544,t5545,t5546,t5547,t5550,t5551,t5552,t5553,t5554,t5556,t5557,t5558,t5559,t5561,t5563,t5564,t5566,t5568,t5569,t5570,t5573,t5574,t5575,t5576,t5577,t5578,t5579,t5580,t5581,t5582,t5583,t5585,t5586,t5588,t5589,t5592,t5593,t5594,t5595,t5596,t5597,t56,t5601,t5602,t5604,t5606,t5612,t5613,t5615,t5617,t5619,t5620,t5621,t5622,t5623,t5624,t5625,t5626,t5627,t5628,t5629,t5631,t5632,t5635,t5636,t5639,t5647,t5650,t5651,t5652,t5653,t5654,t5655,t5657,t5658,t5659,t5660,t5662,t5663,t5664,t5665,t5666,t5670,t5671,t5674,t5675,t5678,t5679,t5681,t5682,t5685,t5687,t5689,t5693,t5694,t5695,t5696,t5698,t5700,t5701,t5702,t5703,t5704,t5705,t5706,t5707,t5708,t5709,t5711,t5712,t5714,t5715,t5716,t5717,t5718,t5720,t5721,t5722,t5723,t5725,t5726,t5727,t5728,t5730,t5731,t5733,t5735,t5737,t5739,t5740,t5741,t5742,t5743,t5745,t5746,t5748,t5749,t5750,t5751,t5756,t5757,t5760,t5761,t5762,t5763,t5764,t5765,t5770,t5771,t5772,t5773,t5775,t5776,t5777,t5778,t5779,t5781,t5782,t5783,t5785,t5786,t5787,t5788,t5791,t5792,t5793,t5794,t5796,t5797,t5798,t5799,t5804,t5805,t5808,t5809,t5810,t5813,t5815,t5816,t5818,t5819,t5820,t5821,t5822,t5824,t5825,t5829,t5831,t5832,t5833,t5835,t5836,t5837,t5838,t5842,t5843,t5844,t5845,t5846,t5847,t5848,t5849,t5850,t5851,t5852,t5853,t5854,t5855,t5857,t5858,t5859,t5860,t5861,t5862,t5863,t5864,t5865,t5866,t5868,t5870,t5871,t5873,t5874,t5875,t5876,t5877,t5879,t5881,t5882,t5883,t5884,t5885,t5886,t5887,t5888,t5889,t5890,t5891,t5892,t5894,t5896,t5899,t5900,t5902,t5904,t5907,t5908,t5910,t5911,t5912,t5913,t5914,t5916,t5917,t5918,t5919,t5922,t5923,t5924,t5925,t5926,t5927,t5929,t5930,t5932,t5933,t5936,t5938,t5939,t5940,t5943,t5944,t5945,t5946,t5947,t5948,t5951,t5952,t5953,t5954,t5956,t5957,t5958,t5959,t5960,t5962,t5963,t5966,t5968,t5969,t5970,t5972,t5973,t5975,t5977,t5978,t5979,t5981,t5982,t5983,t5985,t5987,t5989,t5990,t5991,t5994,t5996,t5997,t5998,t6,t60,t6001,t6002,t6004,t6005,t6007,t6008,t6009,t6010,t6017,t6018,t6019,t6020,t6021,t6022,t6023,t6024,t6028,t6030,t6031,t6034,t6035,t6036,t6037,t6039,t6043,t6044,t6046,t6047,t6048,t6049,t6050,t6051,t6053,t6054,t6055,t6058,t6062,t6064,t6066,t6067,t6068,t6069,t6070,t6071,t6073,t6075,t6076,t6077,t6081,t6088,t6091,t6092,t6095,t6096,t6098,t6099,t6101,t6102,t6103,t6104,t6105,t6107,t6112,t6113,t6114,t6116,t6119,t6120,t6121,t6123,t6124,t6126,t6129,t6130,t6135,t6137,t6139,t6141,t6142,t6143,t6144,t6146,t6147,t6148,t6150,t6154,t6155,t6156,t6157,t6160,t6161,t6162,t6164,t6168,t6169,t6170,t6172,t6178,t6179,t6180,t6182,t6183,t6184,t6185,t6190,t6191,t6195,t6198,t6199,t6200,t6202,t6203,t6206,t6207,t6209,t6210,t6211,t6212,t6213,t6214,t6215,t6218,t6219,t6221,t6222,t6223,t6224,t6225,t6232,t6234,t6235,t6237,t6238,t6239,t6241,t6243,t6244,t6245,t6246,t6247,t6248,t6250,t6251,t6252,t6253,t6257,t6258,t6260,t6262,t6264,t6267,t6270,t6272,t6273,t6274,t6275,t6277,t6282,t6284,t6289,t6293,t6294,t6296,t6297,t6298,t6299,t6302,t6303,t6304,t6305,t6309,t6312,t6317,t6321,t6322,t6323,t6327,t6328,t6330,t6331,t6332,t6333,t6338,t6339,t6341,t6343,t6344,t6345,t6346,t6348,t6349,t6351,t6354,t6356,t6357,t6359,t6360,t6363,t6365,t6366,t6367,t6368,t6369,t6370,t6371,t6372,t6373,t6374,t6375,t6378,t6382,t6384,t6387,t6388,t6389,t6390,t6391,t6393,t6394,t6396,t6397,t6398,t6399,t640,t6400,t6401,t6403,t6404,t6406,t6407,t6410,t6411,t6414,t6417,t6419,t642,t6422,t6423,t6424,t6427,t643,t6431,t6433,t6434,t6435,t6436,t6437,t6439,t6441,t6442,t6445,t6446,t6447,t6450,t6451,t6452,t6453,t6455,t6456,t6463,t6464,t6466,t6468,t6471,t6473,t6474,t6480,t6481,t6482,t6483,t6484,t6485,t6486,t6487,t6489,t649,t6490,t6491,t6492,t6493,t6494,t6495,t6496,t6497,t6503,t6504,t6505,t6507,t6508,t6511,t6515,t6518,t6519,t6521,t6522,t6523,t6525,t6526,t6527,t6528,t6529,t6531,t6532,t6533,t6534,t6543,t6544,t6545,t6559,t6560,t6565,t6566,t6568,t6570,t6571,t6572,t6573,t6574,t6577,t6578,t6580,t6581,t6582,t6584,t6585,t6586,t6591,t6592,t6593,t6594,t6600,t6601,t6603,t6604,t6605,t6607,t6608,t6611,t6612,t6613,t6614,t6634,t6635,t6645,t6649,t6658,t6660,t6663,t6664,t667,t668,t6688,t6689,t669,t6690,t6691,t6692,t670,t6703,t6707,t6708,t6720,t6722,t674,t6752,t6753,t6754,t6755,t6756,t6763,t6764,t6765,t677,t6772,t6776,t6777,t6788,t6789,t6793,t6794,t6795,t6796,t6797,t6807,t6809,t6811,t6812,t6813,t6814,t6815,t6816,t682,t6833,t684,t685,t6854,t6855,t686,t6860,t6861,t6863,t6864,t6866,t687,t6873,t6884,t6885,t6887,t6888,t6889,t6890,t6892,t6893,t6900,t6910,t6913,t6916,t6917,t6920,t6924,t6925,t6926,t6927,t6928,t6932,t6933,t6937,t6943,t6944,t6954,t6955,t6956,t6958,t6972,t6973,t6975,t6979,t6984,t6986,t6988,t6989,t6992,t6993,t7,t7012,t7015,t7018,t7028,t7029,t7039,t7041,t7050,t7051,t7053,t7054,t7055,t7056,t7057,t7058,t7060,t7061,t7062,t7068,t707,t708,t7087,t7089,t7091,t7093,t7094,t7096,t7098,t7099,t71,t710,t7101,t7102,t7103,t7107,t7108,t7114,t7118,t7120,t7127,t7128,t7141,t7148,t715,t7152,t7157,t716,t7174,t7177,t7179,t7181,t7185,t7187,t7188,t7193,t7195,t7198,t7200,t7201,t7204,t7209,t721,t7210,t7211,t7215,t7219,t722,t7222,t7232,t7233,t7236,t7238,t7239,t724,t7240,t7245,t7248,t725,t7257,t7259,t7263,t7264,t7265,t7271,t7277,t7278,t7280,t7281,t7282,t7292,t7293,t7294,t7295,t7296,t7297,t73,t7302,t7303,t7304,t7305,t7308,t7309,t7328,t7349,t7350,t7358,t7371,t7394,t7407,t7427,t7452,t7453,t7454,t7459,t7478,t7479,t749,t7530,t7534,t7553,t7566,t7567,t7606,t762,t7661,t768,t7730,t7731,t7732,t7733,t7734,t777,t7790,t7791,t792,t793,t801,t802,t808,t813,t819,t821,t850,t855,t874,t878,t941,t948,t951,t97});
end
function tau_c = ft_14(ct)
t1005 = ct{1};
t1022 = ct{2};
t1089 = ct{3};
t1104 = ct{4};
t1105 = ct{5};
t1108 = ct{6};
t1115 = ct{7};
t1121 = ct{8};
t1158 = ct{9};
t1159 = ct{10};
t1196 = ct{11};
t1205 = ct{12};
t1210 = ct{13};
t1212 = ct{14};
t1217 = ct{15};
t1218 = ct{16};
t123 = ct{17};
t1237 = ct{18};
t1238 = ct{19};
t1288 = ct{20};
t1289 = ct{21};
t1302 = ct{22};
t1303 = ct{23};
t1319 = ct{24};
t1320 = ct{25};
t1336 = ct{26};
t1348 = ct{27};
t1350 = ct{28};
t1351 = ct{29};
t1360 = ct{30};
t1369 = ct{31};
t1378 = ct{32};
t1396 = ct{33};
t14 = ct{34};
t140 = ct{35};
t1425 = ct{36};
t1435 = ct{37};
t1456 = ct{38};
t1477 = ct{39};
t1488 = ct{40};
t15 = ct{41};
t1513 = ct{42};
t1539 = ct{43};
t1554 = ct{44};
t1577 = ct{45};
t1578 = ct{46};
t1586 = ct{47};
t1587 = ct{48};
t16 = ct{49};
t1600 = ct{50};
t1604 = ct{51};
t1605 = ct{52};
t1606 = ct{53};
t1607 = ct{54};
t1608 = ct{55};
t1609 = ct{56};
t1628 = ct{57};
t1629 = ct{58};
t1637 = ct{59};
t1640 = ct{60};
t1641 = ct{61};
t1659 = ct{62};
t1661 = ct{63};
t1666 = ct{64};
t1667 = ct{65};
t1683 = ct{66};
t1686 = ct{67};
t1690 = ct{68};
t1692 = ct{69};
t17 = ct{70};
t1700 = ct{71};
t1701 = ct{72};
t1705 = ct{73};
t1712 = ct{74};
t1741 = ct{75};
t1742 = ct{76};
t1750 = ct{77};
t1754 = ct{78};
t1758 = ct{79};
t1759 = ct{80};
t1775 = ct{81};
t1776 = ct{82};
t18 = ct{83};
t1861 = ct{84};
t1874 = ct{85};
t1879 = ct{86};
t188 = ct{87};
t1881 = ct{88};
t189 = ct{89};
t1896 = ct{90};
t19 = ct{91};
t1901 = ct{92};
t1941 = ct{93};
t1959 = ct{94};
t1973 = ct{95};
t1993 = ct{96};
t1994 = ct{97};
t2 = ct{98};
t20 = ct{99};
t201 = ct{100};
t202 = ct{101};
t2023 = ct{102};
t2053 = ct{103};
t2060 = ct{104};
t2089 = ct{105};
t2090 = ct{106};
t2098 = ct{107};
t2099 = ct{108};
t21 = ct{109};
t2117 = ct{110};
t2120 = ct{111};
t2122 = ct{112};
t2123 = ct{113};
t2139 = ct{114};
t2140 = ct{115};
t2147 = ct{116};
t2152 = ct{117};
t2154 = ct{118};
t2155 = ct{119};
t2159 = ct{120};
t2165 = ct{121};
t2174 = ct{122};
t2183 = ct{123};
t2187 = ct{124};
t2193 = ct{125};
t2194 = ct{126};
t2195 = ct{127};
t2199 = ct{128};
t22 = ct{129};
t2203 = ct{130};
t2215 = ct{131};
t2219 = ct{132};
t2222 = ct{133};
t2223 = ct{134};
t2239 = ct{135};
t2240 = ct{136};
t2256 = ct{137};
t2257 = ct{138};
t2292 = ct{139};
t2295 = ct{140};
t2297 = ct{141};
t23 = ct{142};
t2302 = ct{143};
t2303 = ct{144};
t2306 = ct{145};
t2307 = ct{146};
t2308 = ct{147};
t2317 = ct{148};
t2337 = ct{149};
t2338 = ct{150};
t2339 = ct{151};
t2355 = ct{152};
t236 = ct{153};
t2361 = ct{154};
t2362 = ct{155};
t2363 = ct{156};
t2367 = ct{157};
t2368 = ct{158};
t237 = ct{159};
t2371 = ct{160};
t2378 = ct{161};
t238 = ct{162};
t2388 = ct{163};
t24 = ct{164};
t2401 = ct{165};
t241 = ct{166};
t2414 = ct{167};
t2419 = ct{168};
t244 = ct{169};
t25 = ct{170};
t2502 = ct{171};
t2510 = ct{172};
t2519 = ct{173};
t2527 = ct{174};
t2530 = ct{175};
t2555 = ct{176};
t2556 = ct{177};
t2572 = ct{178};
t2583 = ct{179};
t2598 = ct{180};
t26 = ct{181};
t2605 = ct{182};
t2606 = ct{183};
t2612 = ct{184};
t2613 = ct{185};
t2618 = ct{186};
t2619 = ct{187};
t262 = ct{188};
t264 = ct{189};
t2651 = ct{190};
t2652 = ct{191};
t2670 = ct{192};
t2671 = ct{193};
t2674 = ct{194};
t2676 = ct{195};
t2680 = ct{196};
t2683 = ct{197};
t2684 = ct{198};
t2689 = ct{199};
t2693 = ct{200};
t2694 = ct{201};
t2695 = ct{202};
t2697 = ct{203};
t2698 = ct{204};
t27 = ct{205};
t2700 = ct{206};
t2701 = ct{207};
t2707 = ct{208};
t2712 = ct{209};
t2715 = ct{210};
t2716 = ct{211};
t2719 = ct{212};
t2721 = ct{213};
t2740 = ct{214};
t2747 = ct{215};
t2754 = ct{216};
t28 = ct{217};
t2801 = ct{218};
t2804 = ct{219};
t2813 = ct{220};
t2814 = ct{221};
t2820 = ct{222};
t2831 = ct{223};
t2834 = ct{224};
t2835 = ct{225};
t2838 = ct{226};
t2850 = ct{227};
t2851 = ct{228};
t2953 = ct{229};
t2963 = ct{230};
t2964 = ct{231};
t2975 = ct{232};
t2979 = ct{233};
t2990 = ct{234};
t2991 = ct{235};
t2994 = ct{236};
t3 = ct{237};
t30 = ct{238};
t3003 = ct{239};
t3009 = ct{240};
t3022 = ct{241};
t3027 = ct{242};
t3030 = ct{243};
t3036 = ct{244};
t3043 = ct{245};
t3047 = ct{246};
t3054 = ct{247};
t3056 = ct{248};
t3057 = ct{249};
t3064 = ct{250};
t3072 = ct{251};
t3080 = ct{252};
t3096 = ct{253};
t3097 = ct{254};
t31 = ct{255};
t3109 = ct{256};
t3117 = ct{257};
t3118 = ct{258};
t3121 = ct{259};
t3122 = ct{260};
t3128 = ct{261};
t313 = ct{262};
t3130 = ct{263};
t3131 = ct{264};
t3132 = ct{265};
t314 = ct{266};
t3141 = ct{267};
t3142 = ct{268};
t3144 = ct{269};
t3147 = ct{270};
t3156 = ct{271};
t3157 = ct{272};
t3170 = ct{273};
t3189 = ct{274};
t3190 = ct{275};
t32 = ct{276};
t3200 = ct{277};
t3206 = ct{278};
t3209 = ct{279};
t321 = ct{280};
t3210 = ct{281};
t3214 = ct{282};
t3228 = ct{283};
t3229 = ct{284};
t3230 = ct{285};
t3231 = ct{286};
t3232 = ct{287};
t3235 = ct{288};
t3250 = ct{289};
t3269 = ct{290};
t3270 = ct{291};
t3272 = ct{292};
t3276 = ct{293};
t3283 = ct{294};
t329 = ct{295};
t3290 = ct{296};
t3291 = ct{297};
t3292 = ct{298};
t3296 = ct{299};
t33 = ct{300};
t3305 = ct{301};
t3306 = ct{302};
t3307 = ct{303};
t3308 = ct{304};
t3313 = ct{305};
t3318 = ct{306};
t3319 = ct{307};
t332 = ct{308};
t3324 = ct{309};
t3327 = ct{310};
t3330 = ct{311};
t3334 = ct{312};
t3336 = ct{313};
t3341 = ct{314};
t3349 = ct{315};
t335 = ct{316};
t3357 = ct{317};
t3359 = ct{318};
t3360 = ct{319};
t3376 = ct{320};
t3385 = ct{321};
t3386 = ct{322};
t3395 = ct{323};
t3399 = ct{324};
t34 = ct{325};
t3405 = ct{326};
t3409 = ct{327};
t3410 = ct{328};
t3412 = ct{329};
t3417 = ct{330};
t3420 = ct{331};
t3421 = ct{332};
t3423 = ct{333};
t3424 = ct{334};
t3435 = ct{335};
t3437 = ct{336};
t3455 = ct{337};
t346 = ct{338};
t3465 = ct{339};
t3468 = ct{340};
t3470 = ct{341};
t3473 = ct{342};
t3475 = ct{343};
t3477 = ct{344};
t3479 = ct{345};
t3480 = ct{346};
t3481 = ct{347};
t3483 = ct{348};
t3484 = ct{349};
t3493 = ct{350};
t3498 = ct{351};
t35 = ct{352};
t350 = ct{353};
t3505 = ct{354};
t3522 = ct{355};
t3524 = ct{356};
t3526 = ct{357};
t3527 = ct{358};
t3528 = ct{359};
t3530 = ct{360};
t3532 = ct{361};
t3533 = ct{362};
t3535 = ct{363};
t3539 = ct{364};
t354 = ct{365};
t3542 = ct{366};
t3544 = ct{367};
t3547 = ct{368};
t3560 = ct{369};
t3563 = ct{370};
t3570 = ct{371};
t3571 = ct{372};
t3576 = ct{373};
t3582 = ct{374};
t3586 = ct{375};
t3587 = ct{376};
t3588 = ct{377};
t3589 = ct{378};
t3590 = ct{379};
t3593 = ct{380};
t3596 = ct{381};
t36 = ct{382};
t3603 = ct{383};
t3616 = ct{384};
t3617 = ct{385};
t3618 = ct{386};
t3619 = ct{387};
t3620 = ct{388};
t3621 = ct{389};
t3622 = ct{390};
t3628 = ct{391};
t3632 = ct{392};
t3633 = ct{393};
t3634 = ct{394};
t3635 = ct{395};
t3637 = ct{396};
t3638 = ct{397};
t3639 = ct{398};
t3643 = ct{399};
t3649 = ct{400};
t3657 = ct{401};
t366 = ct{402};
t3664 = ct{403};
t3665 = ct{404};
t3667 = ct{405};
t3669 = ct{406};
t3670 = ct{407};
t3672 = ct{408};
t3673 = ct{409};
t3674 = ct{410};
t3676 = ct{411};
t3680 = ct{412};
t3681 = ct{413};
t3682 = ct{414};
t3683 = ct{415};
t3684 = ct{416};
t3685 = ct{417};
t3686 = ct{418};
t3687 = ct{419};
t3689 = ct{420};
t3690 = ct{421};
t3693 = ct{422};
t3694 = ct{423};
t3705 = ct{424};
t3706 = ct{425};
t3708 = ct{426};
t3709 = ct{427};
t3713 = ct{428};
t3714 = ct{429};
t3715 = ct{430};
t3716 = ct{431};
t3723 = ct{432};
t3724 = ct{433};
t3729 = ct{434};
t3732 = ct{435};
t3734 = ct{436};
t3735 = ct{437};
t3744 = ct{438};
t3745 = ct{439};
t3746 = ct{440};
t3748 = ct{441};
t3749 = ct{442};
t3751 = ct{443};
t3753 = ct{444};
t3755 = ct{445};
t3756 = ct{446};
t3757 = ct{447};
t3758 = ct{448};
t3759 = ct{449};
t3760 = ct{450};
t3762 = ct{451};
t3763 = ct{452};
t3764 = ct{453};
t3765 = ct{454};
t3766 = ct{455};
t3767 = ct{456};
t3768 = ct{457};
t3769 = ct{458};
t3770 = ct{459};
t3771 = ct{460};
t3772 = ct{461};
t3774 = ct{462};
t3775 = ct{463};
t3776 = ct{464};
t3778 = ct{465};
t3779 = ct{466};
t3782 = ct{467};
t3783 = ct{468};
t3784 = ct{469};
t3790 = ct{470};
t3791 = ct{471};
t3794 = ct{472};
t3795 = ct{473};
t3797 = ct{474};
t3798 = ct{475};
t3799 = ct{476};
t38 = ct{477};
t3801 = ct{478};
t3803 = ct{479};
t3804 = ct{480};
t3806 = ct{481};
t3811 = ct{482};
t3814 = ct{483};
t3815 = ct{484};
t3816 = ct{485};
t3817 = ct{486};
t3819 = ct{487};
t3821 = ct{488};
t3822 = ct{489};
t3826 = ct{490};
t3827 = ct{491};
t3828 = ct{492};
t3833 = ct{493};
t3834 = ct{494};
t3847 = ct{495};
t3849 = ct{496};
t3850 = ct{497};
t3861 = ct{498};
t3862 = ct{499};
t3863 = ct{500};
t3865 = ct{501};
t3866 = ct{502};
t3869 = ct{503};
t387 = ct{504};
t3870 = ct{505};
t3871 = ct{506};
t3872 = ct{507};
t3875 = ct{508};
t3877 = ct{509};
t3880 = ct{510};
t3882 = ct{511};
t3891 = ct{512};
t3892 = ct{513};
t3893 = ct{514};
t3898 = ct{515};
t39 = ct{516};
t3901 = ct{517};
t3904 = ct{518};
t3910 = ct{519};
t3918 = ct{520};
t3922 = ct{521};
t3928 = ct{522};
t3934 = ct{523};
t3940 = ct{524};
t3941 = ct{525};
t3942 = ct{526};
t3946 = ct{527};
t3951 = ct{528};
t3957 = ct{529};
t3959 = ct{530};
t3967 = ct{531};
t3972 = ct{532};
t3974 = ct{533};
t3984 = ct{534};
t3985 = ct{535};
t3992 = ct{536};
t3996 = ct{537};
t4 = ct{538};
t4007 = ct{539};
t4011 = ct{540};
t4013 = ct{541};
t4015 = ct{542};
t4016 = ct{543};
t4027 = ct{544};
t4037 = ct{545};
t4042 = ct{546};
t4043 = ct{547};
t4044 = ct{548};
t4062 = ct{549};
t4071 = ct{550};
t4072 = ct{551};
t4076 = ct{552};
t4077 = ct{553};
t4080 = ct{554};
t4086 = ct{555};
t4096 = ct{556};
t4097 = ct{557};
t4098 = ct{558};
t410 = ct{559};
t4106 = ct{560};
t4108 = ct{561};
t4109 = ct{562};
t4113 = ct{563};
t4119 = ct{564};
t4120 = ct{565};
t4125 = ct{566};
t4127 = ct{567};
t4133 = ct{568};
t4134 = ct{569};
t4146 = ct{570};
t4149 = ct{571};
t4152 = ct{572};
t4153 = ct{573};
t4154 = ct{574};
t4155 = ct{575};
t4160 = ct{576};
t4163 = ct{577};
t4173 = ct{578};
t4175 = ct{579};
t4196 = ct{580};
t42 = ct{581};
t4200 = ct{582};
t4201 = ct{583};
t4219 = ct{584};
t4220 = ct{585};
t4221 = ct{586};
t4227 = ct{587};
t4228 = ct{588};
t4230 = ct{589};
t4231 = ct{590};
t4238 = ct{591};
t4239 = ct{592};
t4242 = ct{593};
t4243 = ct{594};
t4244 = ct{595};
t4245 = ct{596};
t4246 = ct{597};
t4247 = ct{598};
t4248 = ct{599};
t4255 = ct{600};
t4256 = ct{601};
t4257 = ct{602};
t4259 = ct{603};
t4264 = ct{604};
t4266 = ct{605};
t4276 = ct{606};
t4277 = ct{607};
t4279 = ct{608};
t4280 = ct{609};
t4281 = ct{610};
t4285 = ct{611};
t4287 = ct{612};
t4291 = ct{613};
t4292 = ct{614};
t4295 = ct{615};
t4297 = ct{616};
t4298 = ct{617};
t43 = ct{618};
t4304 = ct{619};
t4308 = ct{620};
t4310 = ct{621};
t4311 = ct{622};
t4313 = ct{623};
t4316 = ct{624};
t4320 = ct{625};
t4321 = ct{626};
t4322 = ct{627};
t4323 = ct{628};
t4324 = ct{629};
t4356 = ct{630};
t4362 = ct{631};
t4363 = ct{632};
t4400 = ct{633};
t4405 = ct{634};
t4406 = ct{635};
t4409 = ct{636};
t4413 = ct{637};
t4421 = ct{638};
t4428 = ct{639};
t4429 = ct{640};
t4432 = ct{641};
t4436 = ct{642};
t4437 = ct{643};
t4438 = ct{644};
t4444 = ct{645};
t4447 = ct{646};
t4458 = ct{647};
t4491 = ct{648};
t4496 = ct{649};
t4499 = ct{650};
t4500 = ct{651};
t4504 = ct{652};
t4507 = ct{653};
t4510 = ct{654};
t4513 = ct{655};
t4514 = ct{656};
t4519 = ct{657};
t4520 = ct{658};
t4531 = ct{659};
t4540 = ct{660};
t4541 = ct{661};
t4543 = ct{662};
t4552 = ct{663};
t4554 = ct{664};
t4555 = ct{665};
t4556 = ct{666};
t4560 = ct{667};
t4571 = ct{668};
t4572 = ct{669};
t4576 = ct{670};
t4579 = ct{671};
t4582 = ct{672};
t4588 = ct{673};
t4589 = ct{674};
t4595 = ct{675};
t4599 = ct{676};
t46 = ct{677};
t4602 = ct{678};
t4610 = ct{679};
t4612 = ct{680};
t4613 = ct{681};
t4614 = ct{682};
t4615 = ct{683};
t4617 = ct{684};
t4620 = ct{685};
t4628 = ct{686};
t4629 = ct{687};
t4631 = ct{688};
t4633 = ct{689};
t4634 = ct{690};
t4635 = ct{691};
t4637 = ct{692};
t4639 = ct{693};
t4640 = ct{694};
t4641 = ct{695};
t4642 = ct{696};
t4644 = ct{697};
t4645 = ct{698};
t4647 = ct{699};
t4650 = ct{700};
t4652 = ct{701};
t4655 = ct{702};
t4658 = ct{703};
t4661 = ct{704};
t4663 = ct{705};
t4664 = ct{706};
t4666 = ct{707};
t4667 = ct{708};
t4669 = ct{709};
t4679 = ct{710};
t4680 = ct{711};
t4682 = ct{712};
t4683 = ct{713};
t4686 = ct{714};
t4688 = ct{715};
t4699 = ct{716};
t47 = ct{717};
t4702 = ct{718};
t4703 = ct{719};
t4704 = ct{720};
t4705 = ct{721};
t4737 = ct{722};
t4741 = ct{723};
t4742 = ct{724};
t4744 = ct{725};
t4751 = ct{726};
t4752 = ct{727};
t4758 = ct{728};
t4767 = ct{729};
t4772 = ct{730};
t4777 = ct{731};
t4780 = ct{732};
t4785 = ct{733};
t4786 = ct{734};
t4788 = ct{735};
t4789 = ct{736};
t4790 = ct{737};
t4791 = ct{738};
t4792 = ct{739};
t4793 = ct{740};
t4794 = ct{741};
t4795 = ct{742};
t4796 = ct{743};
t4798 = ct{744};
t4799 = ct{745};
t4800 = ct{746};
t4801 = ct{747};
t4802 = ct{748};
t4803 = ct{749};
t4805 = ct{750};
t4806 = ct{751};
t4807 = ct{752};
t4808 = ct{753};
t4809 = ct{754};
t4812 = ct{755};
t4814 = ct{756};
t4816 = ct{757};
t4817 = ct{758};
t4819 = ct{759};
t4822 = ct{760};
t4823 = ct{761};
t4824 = ct{762};
t4826 = ct{763};
t4829 = ct{764};
t4833 = ct{765};
t4835 = ct{766};
t4836 = ct{767};
t4840 = ct{768};
t4842 = ct{769};
t4843 = ct{770};
t4845 = ct{771};
t4847 = ct{772};
t4848 = ct{773};
t4849 = ct{774};
t4850 = ct{775};
t4851 = ct{776};
t4852 = ct{777};
t4853 = ct{778};
t4856 = ct{779};
t4857 = ct{780};
t4858 = ct{781};
t4859 = ct{782};
t4860 = ct{783};
t4865 = ct{784};
t4868 = ct{785};
t4869 = ct{786};
t4870 = ct{787};
t4871 = ct{788};
t4872 = ct{789};
t4874 = ct{790};
t4875 = ct{791};
t4882 = ct{792};
t4883 = ct{793};
t4898 = ct{794};
t4899 = ct{795};
t4900 = ct{796};
t4902 = ct{797};
t4904 = ct{798};
t4905 = ct{799};
t4906 = ct{800};
t4908 = ct{801};
t4910 = ct{802};
t4911 = ct{803};
t4913 = ct{804};
t4915 = ct{805};
t4917 = ct{806};
t4918 = ct{807};
t4919 = ct{808};
t4920 = ct{809};
t4921 = ct{810};
t4922 = ct{811};
t4924 = ct{812};
t4925 = ct{813};
t4926 = ct{814};
t4927 = ct{815};
t4929 = ct{816};
t4930 = ct{817};
t4931 = ct{818};
t4932 = ct{819};
t4933 = ct{820};
t4934 = ct{821};
t4935 = ct{822};
t4936 = ct{823};
t4938 = ct{824};
t4940 = ct{825};
t4941 = ct{826};
t4942 = ct{827};
t4943 = ct{828};
t4945 = ct{829};
t4946 = ct{830};
t4947 = ct{831};
t4948 = ct{832};
t4950 = ct{833};
t4952 = ct{834};
t4953 = ct{835};
t4954 = ct{836};
t4956 = ct{837};
t4958 = ct{838};
t4959 = ct{839};
t4960 = ct{840};
t4961 = ct{841};
t4962 = ct{842};
t4963 = ct{843};
t4965 = ct{844};
t4970 = ct{845};
t4972 = ct{846};
t4974 = ct{847};
t4975 = ct{848};
t4976 = ct{849};
t4977 = ct{850};
t4980 = ct{851};
t4981 = ct{852};
t4982 = ct{853};
t4983 = ct{854};
t4984 = ct{855};
t4985 = ct{856};
t4986 = ct{857};
t4987 = ct{858};
t4992 = ct{859};
t4994 = ct{860};
t4995 = ct{861};
t4998 = ct{862};
t5 = ct{863};
t50 = ct{864};
t5000 = ct{865};
t5005 = ct{866};
t5006 = ct{867};
t5007 = ct{868};
t5008 = ct{869};
t5013 = ct{870};
t5014 = ct{871};
t5031 = ct{872};
t5033 = ct{873};
t5034 = ct{874};
t5035 = ct{875};
t5036 = ct{876};
t5038 = ct{877};
t5039 = ct{878};
t5040 = ct{879};
t5041 = ct{880};
t5042 = ct{881};
t5047 = ct{882};
t5048 = ct{883};
t5049 = ct{884};
t5051 = ct{885};
t5052 = ct{886};
t5055 = ct{887};
t5056 = ct{888};
t5057 = ct{889};
t5058 = ct{890};
t5059 = ct{891};
t5062 = ct{892};
t5063 = ct{893};
t5066 = ct{894};
t5067 = ct{895};
t5068 = ct{896};
t5069 = ct{897};
t5070 = ct{898};
t5071 = ct{899};
t5073 = ct{900};
t5074 = ct{901};
t5075 = ct{902};
t5076 = ct{903};
t5077 = ct{904};
t5078 = ct{905};
t5079 = ct{906};
t5080 = ct{907};
t5081 = ct{908};
t5083 = ct{909};
t5084 = ct{910};
t5085 = ct{911};
t5086 = ct{912};
t5087 = ct{913};
t5088 = ct{914};
t5089 = ct{915};
t5092 = ct{916};
t5101 = ct{917};
t5102 = ct{918};
t5103 = ct{919};
t5104 = ct{920};
t5105 = ct{921};
t5106 = ct{922};
t5108 = ct{923};
t5109 = ct{924};
t5111 = ct{925};
t5112 = ct{926};
t5113 = ct{927};
t5114 = ct{928};
t5116 = ct{929};
t5117 = ct{930};
t5119 = ct{931};
t5132 = ct{932};
t5133 = ct{933};
t5134 = ct{934};
t5135 = ct{935};
t5136 = ct{936};
t5137 = ct{937};
t5138 = ct{938};
t5139 = ct{939};
t5140 = ct{940};
t5141 = ct{941};
t5142 = ct{942};
t5143 = ct{943};
t5144 = ct{944};
t5147 = ct{945};
t5148 = ct{946};
t5149 = ct{947};
t5150 = ct{948};
t5151 = ct{949};
t5152 = ct{950};
t5153 = ct{951};
t5155 = ct{952};
t5156 = ct{953};
t5157 = ct{954};
t5158 = ct{955};
t5161 = ct{956};
t5162 = ct{957};
t5164 = ct{958};
t5166 = ct{959};
t5170 = ct{960};
t5171 = ct{961};
t5172 = ct{962};
t5173 = ct{963};
t5181 = ct{964};
t5182 = ct{965};
t5183 = ct{966};
t5184 = ct{967};
t5185 = ct{968};
t5186 = ct{969};
t5187 = ct{970};
t5188 = ct{971};
t5189 = ct{972};
t5191 = ct{973};
t5192 = ct{974};
t5195 = ct{975};
t5196 = ct{976};
t5198 = ct{977};
t5201 = ct{978};
t5202 = ct{979};
t5203 = ct{980};
t5204 = ct{981};
t5207 = ct{982};
t5209 = ct{983};
t5210 = ct{984};
t5220 = ct{985};
t5223 = ct{986};
t5224 = ct{987};
t5225 = ct{988};
t5226 = ct{989};
t5227 = ct{990};
t5230 = ct{991};
t5231 = ct{992};
t5233 = ct{993};
t5234 = ct{994};
t5235 = ct{995};
t5238 = ct{996};
t5240 = ct{997};
t5241 = ct{998};
t5243 = ct{999};
t5244 = ct{1000};
t5245 = ct{1001};
t5246 = ct{1002};
t5247 = ct{1003};
t5248 = ct{1004};
t5250 = ct{1005};
t5252 = ct{1006};
t5254 = ct{1007};
t5257 = ct{1008};
t5258 = ct{1009};
t5262 = ct{1010};
t5273 = ct{1011};
t5276 = ct{1012};
t5277 = ct{1013};
t5278 = ct{1014};
t5280 = ct{1015};
t5281 = ct{1016};
t5282 = ct{1017};
t5285 = ct{1018};
t5286 = ct{1019};
t5287 = ct{1020};
t5288 = ct{1021};
t5289 = ct{1022};
t5291 = ct{1023};
t5293 = ct{1024};
t5295 = ct{1025};
t5301 = ct{1026};
t5304 = ct{1027};
t5306 = ct{1028};
t5307 = ct{1029};
t5308 = ct{1030};
t5310 = ct{1031};
t5312 = ct{1032};
t5314 = ct{1033};
t5316 = ct{1034};
t5317 = ct{1035};
t5320 = ct{1036};
t5321 = ct{1037};
t5322 = ct{1038};
t5327 = ct{1039};
t5328 = ct{1040};
t5329 = ct{1041};
t5330 = ct{1042};
t5331 = ct{1043};
t5332 = ct{1044};
t5335 = ct{1045};
t5337 = ct{1046};
t5338 = ct{1047};
t5339 = ct{1048};
t5340 = ct{1049};
t5342 = ct{1050};
t5344 = ct{1051};
t5345 = ct{1052};
t5346 = ct{1053};
t5347 = ct{1054};
t5348 = ct{1055};
t5349 = ct{1056};
t5350 = ct{1057};
t5356 = ct{1058};
t5357 = ct{1059};
t5358 = ct{1060};
t5359 = ct{1061};
t5361 = ct{1062};
t5362 = ct{1063};
t5365 = ct{1064};
t5367 = ct{1065};
t5372 = ct{1066};
t5377 = ct{1067};
t5379 = ct{1068};
t5380 = ct{1069};
t5381 = ct{1070};
t5383 = ct{1071};
t5384 = ct{1072};
t5385 = ct{1073};
t5386 = ct{1074};
t5387 = ct{1075};
t5388 = ct{1076};
t5389 = ct{1077};
t5390 = ct{1078};
t5391 = ct{1079};
t5392 = ct{1080};
t5393 = ct{1081};
t5395 = ct{1082};
t5396 = ct{1083};
t5397 = ct{1084};
t5399 = ct{1085};
t5400 = ct{1086};
t5402 = ct{1087};
t5403 = ct{1088};
t5405 = ct{1089};
t5407 = ct{1090};
t5411 = ct{1091};
t5412 = ct{1092};
t5413 = ct{1093};
t5414 = ct{1094};
t5416 = ct{1095};
t5418 = ct{1096};
t5419 = ct{1097};
t5420 = ct{1098};
t5421 = ct{1099};
t5422 = ct{1100};
t5423 = ct{1101};
t5424 = ct{1102};
t5426 = ct{1103};
t5427 = ct{1104};
t5428 = ct{1105};
t5429 = ct{1106};
t5432 = ct{1107};
t5433 = ct{1108};
t5434 = ct{1109};
t5435 = ct{1110};
t5436 = ct{1111};
t5437 = ct{1112};
t5438 = ct{1113};
t5440 = ct{1114};
t5441 = ct{1115};
t5443 = ct{1116};
t5444 = ct{1117};
t5445 = ct{1118};
t5446 = ct{1119};
t5447 = ct{1120};
t5448 = ct{1121};
t5449 = ct{1122};
t5450 = ct{1123};
t5451 = ct{1124};
t5452 = ct{1125};
t5453 = ct{1126};
t5454 = ct{1127};
t5455 = ct{1128};
t5456 = ct{1129};
t5457 = ct{1130};
t5458 = ct{1131};
t5459 = ct{1132};
t5460 = ct{1133};
t5461 = ct{1134};
t5462 = ct{1135};
t5463 = ct{1136};
t5464 = ct{1137};
t5465 = ct{1138};
t5466 = ct{1139};
t5468 = ct{1140};
t5480 = ct{1141};
t5481 = ct{1142};
t5482 = ct{1143};
t5483 = ct{1144};
t5484 = ct{1145};
t5486 = ct{1146};
t5487 = ct{1147};
t5488 = ct{1148};
t5489 = ct{1149};
t5490 = ct{1150};
t5491 = ct{1151};
t5492 = ct{1152};
t5493 = ct{1153};
t5494 = ct{1154};
t5495 = ct{1155};
t5496 = ct{1156};
t5498 = ct{1157};
t5499 = ct{1158};
t5500 = ct{1159};
t5501 = ct{1160};
t5502 = ct{1161};
t5503 = ct{1162};
t5504 = ct{1163};
t5505 = ct{1164};
t5506 = ct{1165};
t5507 = ct{1166};
t5509 = ct{1167};
t5512 = ct{1168};
t5513 = ct{1169};
t5514 = ct{1170};
t5515 = ct{1171};
t5516 = ct{1172};
t5517 = ct{1173};
t5518 = ct{1174};
t5520 = ct{1175};
t5521 = ct{1176};
t5522 = ct{1177};
t5523 = ct{1178};
t5524 = ct{1179};
t5525 = ct{1180};
t5526 = ct{1181};
t5527 = ct{1182};
t5528 = ct{1183};
t5530 = ct{1184};
t5531 = ct{1185};
t5532 = ct{1186};
t5533 = ct{1187};
t5534 = ct{1188};
t5535 = ct{1189};
t5536 = ct{1190};
t5537 = ct{1191};
t5538 = ct{1192};
t5539 = ct{1193};
t5541 = ct{1194};
t5542 = ct{1195};
t5543 = ct{1196};
t5544 = ct{1197};
t5545 = ct{1198};
t5546 = ct{1199};
t5547 = ct{1200};
t5550 = ct{1201};
t5551 = ct{1202};
t5552 = ct{1203};
t5553 = ct{1204};
t5554 = ct{1205};
t5556 = ct{1206};
t5557 = ct{1207};
t5558 = ct{1208};
t5559 = ct{1209};
t5561 = ct{1210};
t5563 = ct{1211};
t5564 = ct{1212};
t5566 = ct{1213};
t5568 = ct{1214};
t5569 = ct{1215};
t5570 = ct{1216};
t5573 = ct{1217};
t5574 = ct{1218};
t5575 = ct{1219};
t5576 = ct{1220};
t5577 = ct{1221};
t5578 = ct{1222};
t5579 = ct{1223};
t5580 = ct{1224};
t5581 = ct{1225};
t5582 = ct{1226};
t5583 = ct{1227};
t5585 = ct{1228};
t5586 = ct{1229};
t5588 = ct{1230};
t5589 = ct{1231};
t5592 = ct{1232};
t5593 = ct{1233};
t5594 = ct{1234};
t5595 = ct{1235};
t5596 = ct{1236};
t5597 = ct{1237};
t56 = ct{1238};
t5601 = ct{1239};
t5602 = ct{1240};
t5604 = ct{1241};
t5606 = ct{1242};
t5612 = ct{1243};
t5613 = ct{1244};
t5615 = ct{1245};
t5617 = ct{1246};
t5619 = ct{1247};
t5620 = ct{1248};
t5621 = ct{1249};
t5622 = ct{1250};
t5623 = ct{1251};
t5624 = ct{1252};
t5625 = ct{1253};
t5626 = ct{1254};
t5627 = ct{1255};
t5628 = ct{1256};
t5629 = ct{1257};
t5631 = ct{1258};
t5632 = ct{1259};
t5635 = ct{1260};
t5636 = ct{1261};
t5639 = ct{1262};
t5647 = ct{1263};
t5650 = ct{1264};
t5651 = ct{1265};
t5652 = ct{1266};
t5653 = ct{1267};
t5654 = ct{1268};
t5655 = ct{1269};
t5657 = ct{1270};
t5658 = ct{1271};
t5659 = ct{1272};
t5660 = ct{1273};
t5662 = ct{1274};
t5663 = ct{1275};
t5664 = ct{1276};
t5665 = ct{1277};
t5666 = ct{1278};
t5670 = ct{1279};
t5671 = ct{1280};
t5674 = ct{1281};
t5675 = ct{1282};
t5678 = ct{1283};
t5679 = ct{1284};
t5681 = ct{1285};
t5682 = ct{1286};
t5685 = ct{1287};
t5687 = ct{1288};
t5689 = ct{1289};
t5693 = ct{1290};
t5694 = ct{1291};
t5695 = ct{1292};
t5696 = ct{1293};
t5698 = ct{1294};
t5700 = ct{1295};
t5701 = ct{1296};
t5702 = ct{1297};
t5703 = ct{1298};
t5704 = ct{1299};
t5705 = ct{1300};
t5706 = ct{1301};
t5707 = ct{1302};
t5708 = ct{1303};
t5709 = ct{1304};
t5711 = ct{1305};
t5712 = ct{1306};
t5714 = ct{1307};
t5715 = ct{1308};
t5716 = ct{1309};
t5717 = ct{1310};
t5718 = ct{1311};
t5720 = ct{1312};
t5721 = ct{1313};
t5722 = ct{1314};
t5723 = ct{1315};
t5725 = ct{1316};
t5726 = ct{1317};
t5727 = ct{1318};
t5728 = ct{1319};
t5730 = ct{1320};
t5731 = ct{1321};
t5733 = ct{1322};
t5735 = ct{1323};
t5737 = ct{1324};
t5739 = ct{1325};
t5740 = ct{1326};
t5741 = ct{1327};
t5742 = ct{1328};
t5743 = ct{1329};
t5745 = ct{1330};
t5746 = ct{1331};
t5748 = ct{1332};
t5749 = ct{1333};
t5750 = ct{1334};
t5751 = ct{1335};
t5756 = ct{1336};
t5757 = ct{1337};
t5760 = ct{1338};
t5761 = ct{1339};
t5762 = ct{1340};
t5763 = ct{1341};
t5764 = ct{1342};
t5765 = ct{1343};
t5770 = ct{1344};
t5771 = ct{1345};
t5772 = ct{1346};
t5773 = ct{1347};
t5775 = ct{1348};
t5776 = ct{1349};
t5777 = ct{1350};
t5778 = ct{1351};
t5779 = ct{1352};
t5781 = ct{1353};
t5782 = ct{1354};
t5783 = ct{1355};
t5785 = ct{1356};
t5786 = ct{1357};
t5787 = ct{1358};
t5788 = ct{1359};
t5791 = ct{1360};
t5792 = ct{1361};
t5793 = ct{1362};
t5794 = ct{1363};
t5796 = ct{1364};
t5797 = ct{1365};
t5798 = ct{1366};
t5799 = ct{1367};
t5804 = ct{1368};
t5805 = ct{1369};
t5808 = ct{1370};
t5809 = ct{1371};
t5810 = ct{1372};
t5813 = ct{1373};
t5815 = ct{1374};
t5816 = ct{1375};
t5818 = ct{1376};
t5819 = ct{1377};
t5820 = ct{1378};
t5821 = ct{1379};
t5822 = ct{1380};
t5824 = ct{1381};
t5825 = ct{1382};
t5829 = ct{1383};
t5831 = ct{1384};
t5832 = ct{1385};
t5833 = ct{1386};
t5835 = ct{1387};
t5836 = ct{1388};
t5837 = ct{1389};
t5838 = ct{1390};
t5842 = ct{1391};
t5843 = ct{1392};
t5844 = ct{1393};
t5845 = ct{1394};
t5846 = ct{1395};
t5847 = ct{1396};
t5848 = ct{1397};
t5849 = ct{1398};
t5850 = ct{1399};
t5851 = ct{1400};
t5852 = ct{1401};
t5853 = ct{1402};
t5854 = ct{1403};
t5855 = ct{1404};
t5857 = ct{1405};
t5858 = ct{1406};
t5859 = ct{1407};
t5860 = ct{1408};
t5861 = ct{1409};
t5862 = ct{1410};
t5863 = ct{1411};
t5864 = ct{1412};
t5865 = ct{1413};
t5866 = ct{1414};
t5868 = ct{1415};
t5870 = ct{1416};
t5871 = ct{1417};
t5873 = ct{1418};
t5874 = ct{1419};
t5875 = ct{1420};
t5876 = ct{1421};
t5877 = ct{1422};
t5879 = ct{1423};
t5881 = ct{1424};
t5882 = ct{1425};
t5883 = ct{1426};
t5884 = ct{1427};
t5885 = ct{1428};
t5886 = ct{1429};
t5887 = ct{1430};
t5888 = ct{1431};
t5889 = ct{1432};
t5890 = ct{1433};
t5891 = ct{1434};
t5892 = ct{1435};
t5894 = ct{1436};
t5896 = ct{1437};
t5899 = ct{1438};
t5900 = ct{1439};
t5902 = ct{1440};
t5904 = ct{1441};
t5907 = ct{1442};
t5908 = ct{1443};
t5910 = ct{1444};
t5911 = ct{1445};
t5912 = ct{1446};
t5913 = ct{1447};
t5914 = ct{1448};
t5916 = ct{1449};
t5917 = ct{1450};
t5918 = ct{1451};
t5919 = ct{1452};
t5922 = ct{1453};
t5923 = ct{1454};
t5924 = ct{1455};
t5925 = ct{1456};
t5926 = ct{1457};
t5927 = ct{1458};
t5929 = ct{1459};
t5930 = ct{1460};
t5932 = ct{1461};
t5933 = ct{1462};
t5936 = ct{1463};
t5938 = ct{1464};
t5939 = ct{1465};
t5940 = ct{1466};
t5943 = ct{1467};
t5944 = ct{1468};
t5945 = ct{1469};
t5946 = ct{1470};
t5947 = ct{1471};
t5948 = ct{1472};
t5951 = ct{1473};
t5952 = ct{1474};
t5953 = ct{1475};
t5954 = ct{1476};
t5956 = ct{1477};
t5957 = ct{1478};
t5958 = ct{1479};
t5959 = ct{1480};
t5960 = ct{1481};
t5962 = ct{1482};
t5963 = ct{1483};
t5966 = ct{1484};
t5968 = ct{1485};
t5969 = ct{1486};
t5970 = ct{1487};
t5972 = ct{1488};
t5973 = ct{1489};
t5975 = ct{1490};
t5977 = ct{1491};
t5978 = ct{1492};
t5979 = ct{1493};
t5981 = ct{1494};
t5982 = ct{1495};
t5983 = ct{1496};
t5985 = ct{1497};
t5987 = ct{1498};
t5989 = ct{1499};
t5990 = ct{1500};
t5991 = ct{1501};
t5994 = ct{1502};
t5996 = ct{1503};
t5997 = ct{1504};
t5998 = ct{1505};
t6 = ct{1506};
t60 = ct{1507};
t6001 = ct{1508};
t6002 = ct{1509};
t6004 = ct{1510};
t6005 = ct{1511};
t6007 = ct{1512};
t6008 = ct{1513};
t6009 = ct{1514};
t6010 = ct{1515};
t6017 = ct{1516};
t6018 = ct{1517};
t6019 = ct{1518};
t6020 = ct{1519};
t6021 = ct{1520};
t6022 = ct{1521};
t6023 = ct{1522};
t6024 = ct{1523};
t6028 = ct{1524};
t6030 = ct{1525};
t6031 = ct{1526};
t6034 = ct{1527};
t6035 = ct{1528};
t6036 = ct{1529};
t6037 = ct{1530};
t6039 = ct{1531};
t6043 = ct{1532};
t6044 = ct{1533};
t6046 = ct{1534};
t6047 = ct{1535};
t6048 = ct{1536};
t6049 = ct{1537};
t6050 = ct{1538};
t6051 = ct{1539};
t6053 = ct{1540};
t6054 = ct{1541};
t6055 = ct{1542};
t6058 = ct{1543};
t6062 = ct{1544};
t6064 = ct{1545};
t6066 = ct{1546};
t6067 = ct{1547};
t6068 = ct{1548};
t6069 = ct{1549};
t6070 = ct{1550};
t6071 = ct{1551};
t6073 = ct{1552};
t6075 = ct{1553};
t6076 = ct{1554};
t6077 = ct{1555};
t6081 = ct{1556};
t6088 = ct{1557};
t6091 = ct{1558};
t6092 = ct{1559};
t6095 = ct{1560};
t6096 = ct{1561};
t6098 = ct{1562};
t6099 = ct{1563};
t6101 = ct{1564};
t6102 = ct{1565};
t6103 = ct{1566};
t6104 = ct{1567};
t6105 = ct{1568};
t6107 = ct{1569};
t6112 = ct{1570};
t6113 = ct{1571};
t6114 = ct{1572};
t6116 = ct{1573};
t6119 = ct{1574};
t6120 = ct{1575};
t6121 = ct{1576};
t6123 = ct{1577};
t6124 = ct{1578};
t6126 = ct{1579};
t6129 = ct{1580};
t6130 = ct{1581};
t6135 = ct{1582};
t6137 = ct{1583};
t6139 = ct{1584};
t6141 = ct{1585};
t6142 = ct{1586};
t6143 = ct{1587};
t6144 = ct{1588};
t6146 = ct{1589};
t6147 = ct{1590};
t6148 = ct{1591};
t6150 = ct{1592};
t6154 = ct{1593};
t6155 = ct{1594};
t6156 = ct{1595};
t6157 = ct{1596};
t6160 = ct{1597};
t6161 = ct{1598};
t6162 = ct{1599};
t6164 = ct{1600};
t6168 = ct{1601};
t6169 = ct{1602};
t6170 = ct{1603};
t6172 = ct{1604};
t6178 = ct{1605};
t6179 = ct{1606};
t6180 = ct{1607};
t6182 = ct{1608};
t6183 = ct{1609};
t6184 = ct{1610};
t6185 = ct{1611};
t6190 = ct{1612};
t6191 = ct{1613};
t6195 = ct{1614};
t6198 = ct{1615};
t6199 = ct{1616};
t6200 = ct{1617};
t6202 = ct{1618};
t6203 = ct{1619};
t6206 = ct{1620};
t6207 = ct{1621};
t6209 = ct{1622};
t6210 = ct{1623};
t6211 = ct{1624};
t6212 = ct{1625};
t6213 = ct{1626};
t6214 = ct{1627};
t6215 = ct{1628};
t6218 = ct{1629};
t6219 = ct{1630};
t6221 = ct{1631};
t6222 = ct{1632};
t6223 = ct{1633};
t6224 = ct{1634};
t6225 = ct{1635};
t6232 = ct{1636};
t6234 = ct{1637};
t6235 = ct{1638};
t6237 = ct{1639};
t6238 = ct{1640};
t6239 = ct{1641};
t6241 = ct{1642};
t6243 = ct{1643};
t6244 = ct{1644};
t6245 = ct{1645};
t6246 = ct{1646};
t6247 = ct{1647};
t6248 = ct{1648};
t6250 = ct{1649};
t6251 = ct{1650};
t6252 = ct{1651};
t6253 = ct{1652};
t6257 = ct{1653};
t6258 = ct{1654};
t6260 = ct{1655};
t6262 = ct{1656};
t6264 = ct{1657};
t6267 = ct{1658};
t6270 = ct{1659};
t6272 = ct{1660};
t6273 = ct{1661};
t6274 = ct{1662};
t6275 = ct{1663};
t6277 = ct{1664};
t6282 = ct{1665};
t6284 = ct{1666};
t6289 = ct{1667};
t6293 = ct{1668};
t6294 = ct{1669};
t6296 = ct{1670};
t6297 = ct{1671};
t6298 = ct{1672};
t6299 = ct{1673};
t6302 = ct{1674};
t6303 = ct{1675};
t6304 = ct{1676};
t6305 = ct{1677};
t6309 = ct{1678};
t6312 = ct{1679};
t6317 = ct{1680};
t6321 = ct{1681};
t6322 = ct{1682};
t6323 = ct{1683};
t6327 = ct{1684};
t6328 = ct{1685};
t6330 = ct{1686};
t6331 = ct{1687};
t6332 = ct{1688};
t6333 = ct{1689};
t6338 = ct{1690};
t6339 = ct{1691};
t6341 = ct{1692};
t6343 = ct{1693};
t6344 = ct{1694};
t6345 = ct{1695};
t6346 = ct{1696};
t6348 = ct{1697};
t6349 = ct{1698};
t6351 = ct{1699};
t6354 = ct{1700};
t6356 = ct{1701};
t6357 = ct{1702};
t6359 = ct{1703};
t6360 = ct{1704};
t6363 = ct{1705};
t6365 = ct{1706};
t6366 = ct{1707};
t6367 = ct{1708};
t6368 = ct{1709};
t6369 = ct{1710};
t6370 = ct{1711};
t6371 = ct{1712};
t6372 = ct{1713};
t6373 = ct{1714};
t6374 = ct{1715};
t6375 = ct{1716};
t6378 = ct{1717};
t6382 = ct{1718};
t6384 = ct{1719};
t6387 = ct{1720};
t6388 = ct{1721};
t6389 = ct{1722};
t6390 = ct{1723};
t6391 = ct{1724};
t6393 = ct{1725};
t6394 = ct{1726};
t6396 = ct{1727};
t6397 = ct{1728};
t6398 = ct{1729};
t6399 = ct{1730};
t640 = ct{1731};
t6400 = ct{1732};
t6401 = ct{1733};
t6403 = ct{1734};
t6404 = ct{1735};
t6406 = ct{1736};
t6407 = ct{1737};
t6410 = ct{1738};
t6411 = ct{1739};
t6414 = ct{1740};
t6417 = ct{1741};
t6419 = ct{1742};
t642 = ct{1743};
t6422 = ct{1744};
t6423 = ct{1745};
t6424 = ct{1746};
t6427 = ct{1747};
t643 = ct{1748};
t6431 = ct{1749};
t6433 = ct{1750};
t6434 = ct{1751};
t6435 = ct{1752};
t6436 = ct{1753};
t6437 = ct{1754};
t6439 = ct{1755};
t6441 = ct{1756};
t6442 = ct{1757};
t6445 = ct{1758};
t6446 = ct{1759};
t6447 = ct{1760};
t6450 = ct{1761};
t6451 = ct{1762};
t6452 = ct{1763};
t6453 = ct{1764};
t6455 = ct{1765};
t6456 = ct{1766};
t6463 = ct{1767};
t6464 = ct{1768};
t6466 = ct{1769};
t6468 = ct{1770};
t6471 = ct{1771};
t6473 = ct{1772};
t6474 = ct{1773};
t6480 = ct{1774};
t6481 = ct{1775};
t6482 = ct{1776};
t6483 = ct{1777};
t6484 = ct{1778};
t6485 = ct{1779};
t6486 = ct{1780};
t6487 = ct{1781};
t6489 = ct{1782};
t649 = ct{1783};
t6490 = ct{1784};
t6491 = ct{1785};
t6492 = ct{1786};
t6493 = ct{1787};
t6494 = ct{1788};
t6495 = ct{1789};
t6496 = ct{1790};
t6497 = ct{1791};
t6503 = ct{1792};
t6504 = ct{1793};
t6505 = ct{1794};
t6507 = ct{1795};
t6508 = ct{1796};
t6511 = ct{1797};
t6515 = ct{1798};
t6518 = ct{1799};
t6519 = ct{1800};
t6521 = ct{1801};
t6522 = ct{1802};
t6523 = ct{1803};
t6525 = ct{1804};
t6526 = ct{1805};
t6527 = ct{1806};
t6528 = ct{1807};
t6529 = ct{1808};
t6531 = ct{1809};
t6532 = ct{1810};
t6533 = ct{1811};
t6534 = ct{1812};
t6543 = ct{1813};
t6544 = ct{1814};
t6545 = ct{1815};
t6559 = ct{1816};
t6560 = ct{1817};
t6565 = ct{1818};
t6566 = ct{1819};
t6568 = ct{1820};
t6570 = ct{1821};
t6571 = ct{1822};
t6572 = ct{1823};
t6573 = ct{1824};
t6574 = ct{1825};
t6577 = ct{1826};
t6578 = ct{1827};
t6580 = ct{1828};
t6581 = ct{1829};
t6582 = ct{1830};
t6584 = ct{1831};
t6585 = ct{1832};
t6586 = ct{1833};
t6591 = ct{1834};
t6592 = ct{1835};
t6593 = ct{1836};
t6594 = ct{1837};
t6600 = ct{1838};
t6601 = ct{1839};
t6603 = ct{1840};
t6604 = ct{1841};
t6605 = ct{1842};
t6607 = ct{1843};
t6608 = ct{1844};
t6611 = ct{1845};
t6612 = ct{1846};
t6613 = ct{1847};
t6614 = ct{1848};
t6634 = ct{1849};
t6635 = ct{1850};
t6645 = ct{1851};
t6649 = ct{1852};
t6658 = ct{1853};
t6660 = ct{1854};
t6663 = ct{1855};
t6664 = ct{1856};
t667 = ct{1857};
t668 = ct{1858};
t6688 = ct{1859};
t6689 = ct{1860};
t669 = ct{1861};
t6690 = ct{1862};
t6691 = ct{1863};
t6692 = ct{1864};
t670 = ct{1865};
t6703 = ct{1866};
t6707 = ct{1867};
t6708 = ct{1868};
t6720 = ct{1869};
t6722 = ct{1870};
t674 = ct{1871};
t6752 = ct{1872};
t6753 = ct{1873};
t6754 = ct{1874};
t6755 = ct{1875};
t6756 = ct{1876};
t6763 = ct{1877};
t6764 = ct{1878};
t6765 = ct{1879};
t677 = ct{1880};
t6772 = ct{1881};
t6776 = ct{1882};
t6777 = ct{1883};
t6788 = ct{1884};
t6789 = ct{1885};
t6793 = ct{1886};
t6794 = ct{1887};
t6795 = ct{1888};
t6796 = ct{1889};
t6797 = ct{1890};
t6807 = ct{1891};
t6809 = ct{1892};
t6811 = ct{1893};
t6812 = ct{1894};
t6813 = ct{1895};
t6814 = ct{1896};
t6815 = ct{1897};
t6816 = ct{1898};
t682 = ct{1899};
t6833 = ct{1900};
t684 = ct{1901};
t685 = ct{1902};
t6854 = ct{1903};
t6855 = ct{1904};
t686 = ct{1905};
t6860 = ct{1906};
t6861 = ct{1907};
t6863 = ct{1908};
t6864 = ct{1909};
t6866 = ct{1910};
t687 = ct{1911};
t6873 = ct{1912};
t6884 = ct{1913};
t6885 = ct{1914};
t6887 = ct{1915};
t6888 = ct{1916};
t6889 = ct{1917};
t6890 = ct{1918};
t6892 = ct{1919};
t6893 = ct{1920};
t6900 = ct{1921};
t6910 = ct{1922};
t6913 = ct{1923};
t6916 = ct{1924};
t6917 = ct{1925};
t6920 = ct{1926};
t6924 = ct{1927};
t6925 = ct{1928};
t6926 = ct{1929};
t6927 = ct{1930};
t6928 = ct{1931};
t6932 = ct{1932};
t6933 = ct{1933};
t6937 = ct{1934};
t6943 = ct{1935};
t6944 = ct{1936};
t6954 = ct{1937};
t6955 = ct{1938};
t6956 = ct{1939};
t6958 = ct{1940};
t6972 = ct{1941};
t6973 = ct{1942};
t6975 = ct{1943};
t6979 = ct{1944};
t6984 = ct{1945};
t6986 = ct{1946};
t6988 = ct{1947};
t6989 = ct{1948};
t6992 = ct{1949};
t6993 = ct{1950};
t7 = ct{1951};
t7012 = ct{1952};
t7015 = ct{1953};
t7018 = ct{1954};
t7028 = ct{1955};
t7029 = ct{1956};
t7039 = ct{1957};
t7041 = ct{1958};
t7050 = ct{1959};
t7051 = ct{1960};
t7053 = ct{1961};
t7054 = ct{1962};
t7055 = ct{1963};
t7056 = ct{1964};
t7057 = ct{1965};
t7058 = ct{1966};
t7060 = ct{1967};
t7061 = ct{1968};
t7062 = ct{1969};
t7068 = ct{1970};
t707 = ct{1971};
t708 = ct{1972};
t7087 = ct{1973};
t7089 = ct{1974};
t7091 = ct{1975};
t7093 = ct{1976};
t7094 = ct{1977};
t7096 = ct{1978};
t7098 = ct{1979};
t7099 = ct{1980};
t71 = ct{1981};
t710 = ct{1982};
t7101 = ct{1983};
t7102 = ct{1984};
t7103 = ct{1985};
t7107 = ct{1986};
t7108 = ct{1987};
t7114 = ct{1988};
t7118 = ct{1989};
t7120 = ct{1990};
t7127 = ct{1991};
t7128 = ct{1992};
t7141 = ct{1993};
t7148 = ct{1994};
t715 = ct{1995};
t7152 = ct{1996};
t7157 = ct{1997};
t716 = ct{1998};
t7174 = ct{1999};
t7177 = ct{2000};
